simulink library "MBDS_Subsystems"  (R2018b)
settings: Solver=ode45  StartTime=0.0  StopTime=10.0  RelTol=1e-3
libraries: KIBES_Signal x1429, MBDS_Modules x44, simulink x2
(part 12 of 15)

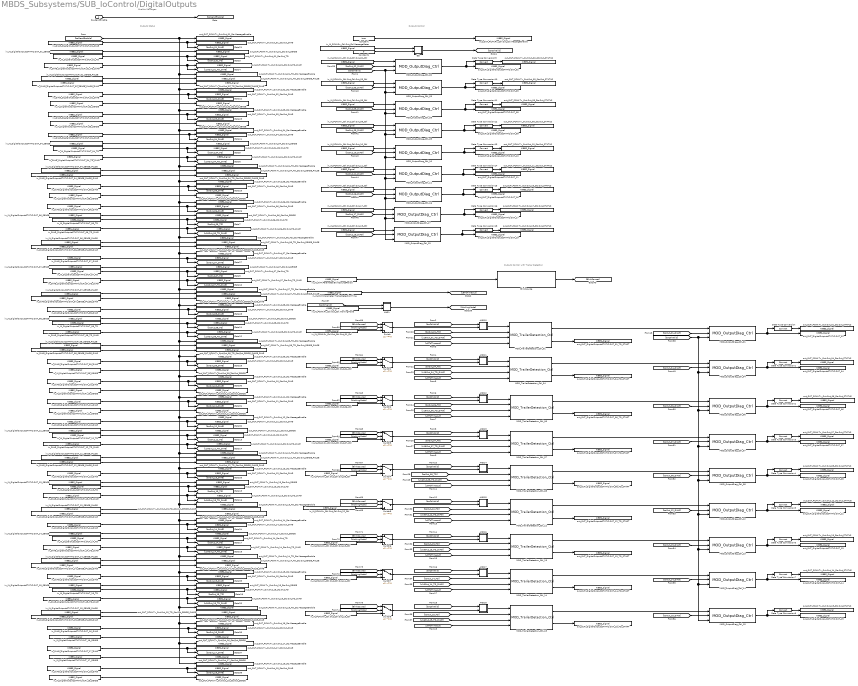
== system MBDS_Subsystems/SUB_IoControl/DigitalOutputs ==
  note: Outputs Control with Trailer Detection
  note: Outputs Control
  note: Enable Messages
  note: Outputs Status
  bo_SendEnable : Inport
  AND1 : Subsystem  InitFcn=|  mask(AND){MBDS_LibraryBlock=on, BitwiseMode=off, Inputs=2, UseBitMask=off, BitMask='A7', OutDataTypeStr=Inherit: Inherit via back propagation, MBDS_BlockVersion=08.20.02}
      | if(exist('MBDS_BlockCallback', 'file'))
      |    MBDS_BlockCallback('Update', gcb);
      | end
      mask prompts: MBDS_LibraryBlock "MBDS library block"; BitwiseMode "Use 'bitwise' mode"; Inputs "Number of input ports:"; UseBitMask "Use bit mask"; BitMask "Bit mask:"; OutDataTypeStr "Output data type:"; MBDS_BlockVersion "Version:"
      mask help: Logical or bitwise AND operator. For multiple inputs, operators are applied across the inputs. For a single input, operators are applied across the input vector. In bitwise mode a bit mask can be applied onto single input signals.
      mask init: same as MBDS_Subsystems/SUB_DateTime/AND
      mask Help: eval(['open([workdir(''library_dir:''),''\Blockset\help\'',get_param(gcb,''MaskType''),''.html''])'])
      mask Callback BitwiseMode:
      | if(exist('MBDS_BlockCallback', 'file'))
      |    MBDS_BlockCallback('BitwiseMode', gcb);
      | end
      mask Callback Inputs:
      | if(exist('MBDS_BlockCallback', 'file'))
      |    MBDS_BlockCallback('Inputs', gcb);
      | end
      mask Callback UseBitMask:
      | if(exist('MBDS_BlockCallback', 'file'))
      |    MBDS_BlockCallback('UseBitMask', gcb);
      | end
      mask Callback BitMask:
      | if(exist('MBDS_BlockCallback', 'file'))
      |    MBDS_BlockCallback('BitMask', gcb);
      | end
      mask TypeOptions OutDataTypeStr: Inherit: Inherit via back propagation | int8 | uint8 | int16 | uint16 | int32 | uint32 | boolean
      mask Callback OutDataTypeStr:
      | % Adopt Value
      | if(exist('MBDS_BlockCallback', 'file'))
      |    MBDS_BlockCallback('OutDataTypeStr', gcb);
      | end
      mask DialogControl ParameterTabVar0 Prompt: Main
      mask DialogControl ParameterTabVar01 Prompt: Signal Attributes
      mask DialogControl ParameterTabVar012 Prompt: Version
      mask Display:
      | % Show icon or block text
      | if(UseBitMask)
      |    if(isnumeric(BitMask))
      |       BitMaskString = ['0x',dec2hex(floor(BitMask))];
      |    elseif(ischar(BitMask))
      |       BitMaskString = ['0x',upper(BitMask)];
      |    else
      |       BitMaskString = '???';
      |    end
      |    disp(sprintf(['AND\n', BitMaskString]))
      | else
      |    disp('AND')
      | end
  AND10 : Subsystem  InitFcn=|  mask(AND){MBDS_LibraryBlock=on, BitwiseMode=off, Inputs=2, UseBitMask=off, BitMask='A7', OutDataTypeStr=Inherit: Inherit via back propagation, MBDS_BlockVersion=08.20.02}
      | if(exist('MBDS_BlockCallback', 'file'))
      |    MBDS_BlockCallback('Update', gcb);
      | end
      mask prompts: MBDS_LibraryBlock "MBDS library block"; BitwiseMode "Use 'bitwise' mode"; Inputs "Number of input ports:"; UseBitMask "Use bit mask"; BitMask "Bit mask:"; OutDataTypeStr "Output data type:"; MBDS_BlockVersion "Version:"
      mask help: Logical or bitwise AND operator. For multiple inputs, operators are applied across the inputs. For a single input, operators are applied across the input vector. In bitwise mode a bit mask can be applied onto single input signals.
      mask init: same as MBDS_Subsystems/SUB_DateTime/AND
      mask Help: eval(['open([workdir(''library_dir:''),''\Blockset\help\'',get_param(gcb,''MaskType''),''.html''])'])
      mask Callback BitwiseMode:
      | if(exist('MBDS_BlockCallback', 'file'))
      |    MBDS_BlockCallback('BitwiseMode', gcb);
      | end
      mask Callback Inputs:
      | if(exist('MBDS_BlockCallback', 'file'))
      |    MBDS_BlockCallback('Inputs', gcb);
      | end
      mask Callback UseBitMask:
      | if(exist('MBDS_BlockCallback', 'file'))
      |    MBDS_BlockCallback('UseBitMask', gcb);
      | end
      mask Callback BitMask:
      | if(exist('MBDS_BlockCallback', 'file'))
      |    MBDS_BlockCallback('BitMask', gcb);
      | end
      mask TypeOptions OutDataTypeStr: Inherit: Inherit via back propagation | int8 | uint8 | int16 | uint16 | int32 | uint32 | boolean
      mask Callback OutDataTypeStr:
      | % Adopt Value
      | if(exist('MBDS_BlockCallback', 'file'))
      |    MBDS_BlockCallback('OutDataTypeStr', gcb);
      | end
      mask DialogControl ParameterTabVar0 Prompt: Main
      mask DialogControl ParameterTabVar01 Prompt: Signal Attributes
      mask DialogControl ParameterTabVar012 Prompt: Version
      mask Display:
      | % Show icon or block text
      | if(UseBitMask)
      |    if(isnumeric(BitMask))
      |       BitMaskString = ['0x',dec2hex(floor(BitMask))];
      |    elseif(ischar(BitMask))
      |       BitMaskString = ['0x',upper(BitMask)];
      |    else
      |       BitMaskString = '???';
      |    end
      |    disp(sprintf(['AND\n', BitMaskString]))
      | else
      |    disp('AND')
      | end
  AND11 : Subsystem  InitFcn=|  mask(AND){MBDS_LibraryBlock=on, BitwiseMode=off, Inputs=2, UseBitMask=off, BitMask='A7', OutDataTypeStr=Inherit: Inherit via back propagation, MBDS_BlockVersion=08.20.02}
      | if(exist('MBDS_BlockCallback', 'file'))
      |    MBDS_BlockCallback('Update', gcb);
      | end
      mask prompts: MBDS_LibraryBlock "MBDS library block"; BitwiseMode "Use 'bitwise' mode"; Inputs "Number of input ports:"; UseBitMask "Use bit mask"; BitMask "Bit mask:"; OutDataTypeStr "Output data type:"; MBDS_BlockVersion "Version:"
      mask help: Logical or bitwise AND operator. For multiple inputs, operators are applied across the inputs. For a single input, operators are applied across the input vector. In bitwise mode a bit mask can be applied onto single input signals.
      mask init: same as MBDS_Subsystems/SUB_DateTime/AND
      mask Help: eval(['open([workdir(''library_dir:''),''\Blockset\help\'',get_param(gcb,''MaskType''),''.html''])'])
      mask Callback BitwiseMode:
      | if(exist('MBDS_BlockCallback', 'file'))
      |    MBDS_BlockCallback('BitwiseMode', gcb);
      | end
      mask Callback Inputs:
      | if(exist('MBDS_BlockCallback', 'file'))
      |    MBDS_BlockCallback('Inputs', gcb);
      | end
      mask Callback UseBitMask:
      | if(exist('MBDS_BlockCallback', 'file'))
      |    MBDS_BlockCallback('UseBitMask', gcb);
      | end
      mask Callback BitMask:
      | if(exist('MBDS_BlockCallback', 'file'))
      |    MBDS_BlockCallback('BitMask', gcb);
      | end
      mask TypeOptions OutDataTypeStr: Inherit: Inherit via back propagation | int8 | uint8 | int16 | uint16 | int32 | uint32 | boolean
      mask Callback OutDataTypeStr:
      | % Adopt Value
      | if(exist('MBDS_BlockCallback', 'file'))
      |    MBDS_BlockCallback('OutDataTypeStr', gcb);
      | end
      mask DialogControl ParameterTabVar0 Prompt: Main
      mask DialogControl ParameterTabVar01 Prompt: Signal Attributes
      mask DialogControl ParameterTabVar012 Prompt: Version
      mask Display:
      | % Show icon or block text
      | if(UseBitMask)
      |    if(isnumeric(BitMask))
      |       BitMaskString = ['0x',dec2hex(floor(BitMask))];
      |    elseif(ischar(BitMask))
      |       BitMaskString = ['0x',upper(BitMask)];
      |    else
      |       BitMaskString = '???';
      |    end
      |    disp(sprintf(['AND\n', BitMaskString]))
      | else
      |    disp('AND')
      | end
  AND12 : Subsystem  InitFcn=|  mask(AND){MBDS_LibraryBlock=on, BitwiseMode=off, Inputs=2, UseBitMask=off, BitMask='A7', OutDataTypeStr=Inherit: Inherit via back propagation, MBDS_BlockVersion=08.20.02}
      | if(exist('MBDS_BlockCallback', 'file'))
      |    MBDS_BlockCallback('Update', gcb);
      | end
      mask prompts: MBDS_LibraryBlock "MBDS library block"; BitwiseMode "Use 'bitwise' mode"; Inputs "Number of input ports:"; UseBitMask "Use bit mask"; BitMask "Bit mask:"; OutDataTypeStr "Output data type:"; MBDS_BlockVersion "Version:"
      mask help: Logical or bitwise AND operator. For multiple inputs, operators are applied across the inputs. For a single input, operators are applied across the input vector. In bitwise mode a bit mask can be applied onto single input signals.
      mask init: same as MBDS_Subsystems/SUB_DateTime/AND
      mask Help: eval(['open([workdir(''library_dir:''),''\Blockset\help\'',get_param(gcb,''MaskType''),''.html''])'])
      mask Callback BitwiseMode:
      | if(exist('MBDS_BlockCallback', 'file'))
      |    MBDS_BlockCallback('BitwiseMode', gcb);
      | end
      mask Callback Inputs:
      | if(exist('MBDS_BlockCallback', 'file'))
      |    MBDS_BlockCallback('Inputs', gcb);
      | end
      mask Callback UseBitMask:
      | if(exist('MBDS_BlockCallback', 'file'))
      |    MBDS_BlockCallback('UseBitMask', gcb);
      | end
      mask Callback BitMask:
      | if(exist('MBDS_BlockCallback', 'file'))
      |    MBDS_BlockCallback('BitMask', gcb);
      | end
      mask TypeOptions OutDataTypeStr: Inherit: Inherit via back propagation | int8 | uint8 | int16 | uint16 | int32 | uint32 | boolean
      mask Callback OutDataTypeStr:
      | % Adopt Value
      | if(exist('MBDS_BlockCallback', 'file'))
      |    MBDS_BlockCallback('OutDataTypeStr', gcb);
      | end
      mask DialogControl ParameterTabVar0 Prompt: Main
      mask DialogControl ParameterTabVar01 Prompt: Signal Attributes
      mask DialogControl ParameterTabVar012 Prompt: Version
      mask Display:
      | % Show icon or block text
      | if(UseBitMask)
      |    if(isnumeric(BitMask))
      |       BitMaskString = ['0x',dec2hex(floor(BitMask))];
      |    elseif(ischar(BitMask))
      |       BitMaskString = ['0x',upper(BitMask)];
      |    else
      |       BitMaskString = '???';
      |    end
      |    disp(sprintf(['AND\n', BitMaskString]))
      | else
      |    disp('AND')
      | end
  AND13 : Subsystem  InitFcn=|  mask(AND){MBDS_LibraryBlock=on, BitwiseMode=off, Inputs=2, UseBitMask=off, BitMask='A7', OutDataTypeStr=Inherit: Inherit via back propagation, MBDS_BlockVersion=08.20.02}
      | if(exist('MBDS_BlockCallback', 'file'))
      |    MBDS_BlockCallback('Update', gcb);
      | end
      mask prompts: MBDS_LibraryBlock "MBDS library block"; BitwiseMode "Use 'bitwise' mode"; Inputs "Number of input ports:"; UseBitMask "Use bit mask"; BitMask "Bit mask:"; OutDataTypeStr "Output data type:"; MBDS_BlockVersion "Version:"
      mask help: Logical or bitwise AND operator. For multiple inputs, operators are applied across the inputs. For a single input, operators are applied across the input vector. In bitwise mode a bit mask can be applied onto single input signals.
      mask init: same as MBDS_Subsystems/SUB_DateTime/AND
      mask Help: eval(['open([workdir(''library_dir:''),''\Blockset\help\'',get_param(gcb,''MaskType''),''.html''])'])
      mask Callback BitwiseMode:
      | if(exist('MBDS_BlockCallback', 'file'))
      |    MBDS_BlockCallback('BitwiseMode', gcb);
      | end
      mask Callback Inputs:
      | if(exist('MBDS_BlockCallback', 'file'))
      |    MBDS_BlockCallback('Inputs', gcb);
      | end
      mask Callback UseBitMask:
      | if(exist('MBDS_BlockCallback', 'file'))
      |    MBDS_BlockCallback('UseBitMask', gcb);
      | end
      mask Callback BitMask:
      | if(exist('MBDS_BlockCallback', 'file'))
      |    MBDS_BlockCallback('BitMask', gcb);
      | end
      mask TypeOptions OutDataTypeStr: Inherit: Inherit via back propagation | int8 | uint8 | int16 | uint16 | int32 | uint32 | boolean
      mask Callback OutDataTypeStr:
      | % Adopt Value
      | if(exist('MBDS_BlockCallback', 'file'))
      |    MBDS_BlockCallback('OutDataTypeStr', gcb);
      | end
      mask DialogControl ParameterTabVar0 Prompt: Main
      mask DialogControl ParameterTabVar01 Prompt: Signal Attributes
      mask DialogControl ParameterTabVar012 Prompt: Version
      mask Display:
      | % Show icon or block text
      | if(UseBitMask)
      |    if(isnumeric(BitMask))
      |       BitMaskString = ['0x',dec2hex(floor(BitMask))];
      |    elseif(ischar(BitMask))
      |       BitMaskString = ['0x',upper(BitMask)];
      |    else
      |       BitMaskString = '???';
      |    end
      |    disp(sprintf(['AND\n', BitMaskString]))
      | else
      |    disp('AND')
      | end
  AND14 : Subsystem  InitFcn=|  mask(AND){MBDS_LibraryBlock=on, BitwiseMode=off, Inputs=2, UseBitMask=off, BitMask='A7', OutDataTypeStr=Inherit: Inherit via back propagation, MBDS_BlockVersion=08.20.02}
      | if(exist('MBDS_BlockCallback', 'file'))
      |    MBDS_BlockCallback('Update', gcb);
      | end
      mask prompts: MBDS_LibraryBlock "MBDS library block"; BitwiseMode "Use 'bitwise' mode"; Inputs "Number of input ports:"; UseBitMask "Use bit mask"; BitMask "Bit mask:"; OutDataTypeStr "Output data type:"; MBDS_BlockVersion "Version:"
      mask help: Logical or bitwise AND operator. For multiple inputs, operators are applied across the inputs. For a single input, operators are applied across the input vector. In bitwise mode a bit mask can be applied onto single input signals.
      mask init: same as MBDS_Subsystems/SUB_DateTime/AND
      mask Help: eval(['open([workdir(''library_dir:''),''\Blockset\help\'',get_param(gcb,''MaskType''),''.html''])'])
      mask Callback BitwiseMode:
      | if(exist('MBDS_BlockCallback', 'file'))
      |    MBDS_BlockCallback('BitwiseMode', gcb);
      | end
      mask Callback Inputs:
      | if(exist('MBDS_BlockCallback', 'file'))
      |    MBDS_BlockCallback('Inputs', gcb);
      | end
      mask Callback UseBitMask:
      | if(exist('MBDS_BlockCallback', 'file'))
      |    MBDS_BlockCallback('UseBitMask', gcb);
      | end
      mask Callback BitMask:
      | if(exist('MBDS_BlockCallback', 'file'))
      |    MBDS_BlockCallback('BitMask', gcb);
      | end
      mask TypeOptions OutDataTypeStr: Inherit: Inherit via back propagation | int8 | uint8 | int16 | uint16 | int32 | uint32 | boolean
      mask Callback OutDataTypeStr:
      | % Adopt Value
      | if(exist('MBDS_BlockCallback', 'file'))
      |    MBDS_BlockCallback('OutDataTypeStr', gcb);
      | end
      mask DialogControl ParameterTabVar0 Prompt: Main
      mask DialogControl ParameterTabVar01 Prompt: Signal Attributes
      mask DialogControl ParameterTabVar012 Prompt: Version
      mask Display:
      | % Show icon or block text
      | if(UseBitMask)
      |    if(isnumeric(BitMask))
      |       BitMaskString = ['0x',dec2hex(floor(BitMask))];
      |    elseif(ischar(BitMask))
      |       BitMaskString = ['0x',upper(BitMask)];
      |    else
      |       BitMaskString = '???';
      |    end
      |    disp(sprintf(['AND\n', BitMaskString]))
      | else
      |    disp('AND')
      | end
  AND15 : Subsystem  InitFcn=|  mask(AND){MBDS_LibraryBlock=on, BitwiseMode=off, Inputs=2, UseBitMask=off, BitMask='A7', OutDataTypeStr=Inherit: Inherit via back propagation, MBDS_BlockVersion=08.20.02}
      | if(exist('MBDS_BlockCallback', 'file'))
      |    MBDS_BlockCallback('Update', gcb);
      | end
      mask prompts: MBDS_LibraryBlock "MBDS library block"; BitwiseMode "Use 'bitwise' mode"; Inputs "Number of input ports:"; UseBitMask "Use bit mask"; BitMask "Bit mask:"; OutDataTypeStr "Output data type:"; MBDS_BlockVersion "Version:"
      mask help: Logical or bitwise AND operator. For multiple inputs, operators are applied across the inputs. For a single input, operators are applied across the input vector. In bitwise mode a bit mask can be applied onto single input signals.
      mask init: same as MBDS_Subsystems/SUB_DateTime/AND
      mask Help: eval(['open([workdir(''library_dir:''),''\Blockset\help\'',get_param(gcb,''MaskType''),''.html''])'])
      mask Callback BitwiseMode:
      | if(exist('MBDS_BlockCallback', 'file'))
      |    MBDS_BlockCallback('BitwiseMode', gcb);
      | end
      mask Callback Inputs:
      | if(exist('MBDS_BlockCallback', 'file'))
      |    MBDS_BlockCallback('Inputs', gcb);
      | end
      mask Callback UseBitMask:
      | if(exist('MBDS_BlockCallback', 'file'))
      |    MBDS_BlockCallback('UseBitMask', gcb);
      | end
      mask Callback BitMask:
      | if(exist('MBDS_BlockCallback', 'file'))
      |    MBDS_BlockCallback('BitMask', gcb);
      | end
      mask TypeOptions OutDataTypeStr: Inherit: Inherit via back propagation | int8 | uint8 | int16 | uint16 | int32 | uint32 | boolean
      mask Callback OutDataTypeStr:
      | % Adopt Value
      | if(exist('MBDS_BlockCallback', 'file'))
      |    MBDS_BlockCallback('OutDataTypeStr', gcb);
      | end
      mask DialogControl ParameterTabVar0 Prompt: Main
      mask DialogControl ParameterTabVar01 Prompt: Signal Attributes
      mask DialogControl ParameterTabVar012 Prompt: Version
      mask Display:
      | % Show icon or block text
      | if(UseBitMask)
      |    if(isnumeric(BitMask))
      |       BitMaskString = ['0x',dec2hex(floor(BitMask))];
      |    elseif(ischar(BitMask))
      |       BitMaskString = ['0x',upper(BitMask)];
      |    else
      |       BitMaskString = '???';
      |    end
      |    disp(sprintf(['AND\n', BitMaskString]))
      | else
      |    disp('AND')
      | end
  AND16 : Subsystem  InitFcn=|  mask(AND){MBDS_LibraryBlock=on, BitwiseMode=off, Inputs=2, UseBitMask=off, BitMask='A7', OutDataTypeStr=Inherit: Inherit via back propagation, MBDS_BlockVersion=08.20.02}
      | if(exist('MBDS_BlockCallback', 'file'))
      |    MBDS_BlockCallback('Update', gcb);
      | end
      mask prompts: MBDS_LibraryBlock "MBDS library block"; BitwiseMode "Use 'bitwise' mode"; Inputs "Number of input ports:"; UseBitMask "Use bit mask"; BitMask "Bit mask:"; OutDataTypeStr "Output data type:"; MBDS_BlockVersion "Version:"
      mask help: Logical or bitwise AND operator. For multiple inputs, operators are applied across the inputs. For a single input, operators are applied across the input vector. In bitwise mode a bit mask can be applied onto single input signals.
      mask init: same as MBDS_Subsystems/SUB_DateTime/AND
      mask Help: eval(['open([workdir(''library_dir:''),''\Blockset\help\'',get_param(gcb,''MaskType''),''.html''])'])
      mask Callback BitwiseMode:
      | if(exist('MBDS_BlockCallback', 'file'))
      |    MBDS_BlockCallback('BitwiseMode', gcb);
      | end
      mask Callback Inputs:
      | if(exist('MBDS_BlockCallback', 'file'))
      |    MBDS_BlockCallback('Inputs', gcb);
      | end
      mask Callback UseBitMask:
      | if(exist('MBDS_BlockCallback', 'file'))
      |    MBDS_BlockCallback('UseBitMask', gcb);
      | end
      mask Callback BitMask:
      | if(exist('MBDS_BlockCallback', 'file'))
      |    MBDS_BlockCallback('BitMask', gcb);
      | end
      mask TypeOptions OutDataTypeStr: Inherit: Inherit via back propagation | int8 | uint8 | int16 | uint16 | int32 | uint32 | boolean
      mask Callback OutDataTypeStr:
      | % Adopt Value
      | if(exist('MBDS_BlockCallback', 'file'))
      |    MBDS_BlockCallback('OutDataTypeStr', gcb);
      | end
      mask DialogControl ParameterTabVar0 Prompt: Main
      mask DialogControl ParameterTabVar01 Prompt: Signal Attributes
      mask DialogControl ParameterTabVar012 Prompt: Version
      mask Display:
      | % Show icon or block text
      | if(UseBitMask)
      |    if(isnumeric(BitMask))
      |       BitMaskString = ['0x',dec2hex(floor(BitMask))];
      |    elseif(ischar(BitMask))
      |       BitMaskString = ['0x',upper(BitMask)];
      |    else
      |       BitMaskString = '???';
      |    end
      |    disp(sprintf(['AND\n', BitMaskString]))
      | else
      |    disp('AND')
      | end
  AND17 : Subsystem  InitFcn=|  mask(AND){MBDS_LibraryBlock=on, BitwiseMode=off, Inputs=2, UseBitMask=off, BitMask='A7', OutDataTypeStr=Inherit: Inherit via back propagation, MBDS_BlockVersion=08.20.02}
      | if(exist('MBDS_BlockCallback', 'file'))
      |    MBDS_BlockCallback('Update', gcb);
      | end
      mask prompts: MBDS_LibraryBlock "MBDS library block"; BitwiseMode "Use 'bitwise' mode"; Inputs "Number of input ports:"; UseBitMask "Use bit mask"; BitMask "Bit mask:"; OutDataTypeStr "Output data type:"; MBDS_BlockVersion "Version:"
      mask help: Logical or bitwise AND operator. For multiple inputs, operators are applied across the inputs. For a single input, operators are applied across the input vector. In bitwise mode a bit mask can be applied onto single input signals.
      mask init: same as MBDS_Subsystems/SUB_DateTime/AND
      mask Help: eval(['open([workdir(''library_dir:''),''\Blockset\help\'',get_param(gcb,''MaskType''),''.html''])'])
      mask Callback BitwiseMode:
      | if(exist('MBDS_BlockCallback', 'file'))
      |    MBDS_BlockCallback('BitwiseMode', gcb);
      | end
      mask Callback Inputs:
      | if(exist('MBDS_BlockCallback', 'file'))
      |    MBDS_BlockCallback('Inputs', gcb);
      | end
      mask Callback UseBitMask:
      | if(exist('MBDS_BlockCallback', 'file'))
      |    MBDS_BlockCallback('UseBitMask', gcb);
      | end
      mask Callback BitMask:
      | if(exist('MBDS_BlockCallback', 'file'))
      |    MBDS_BlockCallback('BitMask', gcb);
      | end
      mask TypeOptions OutDataTypeStr: Inherit: Inherit via back propagation | int8 | uint8 | int16 | uint16 | int32 | uint32 | boolean
      mask Callback OutDataTypeStr:
      | % Adopt Value
      | if(exist('MBDS_BlockCallback', 'file'))
      |    MBDS_BlockCallback('OutDataTypeStr', gcb);
      | end
      mask DialogControl ParameterTabVar0 Prompt: Main
      mask DialogControl ParameterTabVar01 Prompt: Signal Attributes
      mask DialogControl ParameterTabVar012 Prompt: Version
      mask Display:
      | % Show icon or block text
      | if(UseBitMask)
      |    if(isnumeric(BitMask))
      |       BitMaskString = ['0x',dec2hex(floor(BitMask))];
      |    elseif(ischar(BitMask))
      |       BitMaskString = ['0x',upper(BitMask)];
      |    else
      |       BitMaskString = '???';
      |    end
      |    disp(sprintf(['AND\n', BitMaskString]))
      | else
      |    disp('AND')
      | end
  AND18 : Subsystem  InitFcn=|  mask(AND){MBDS_LibraryBlock=on, BitwiseMode=off, Inputs=2, UseBitMask=off, BitMask='A7', OutDataTypeStr=Inherit: Inherit via back propagation, MBDS_BlockVersion=08.20.02}
      | if(exist('MBDS_BlockCallback', 'file'))
      |    MBDS_BlockCallback('Update', gcb);
      | end
      mask prompts: MBDS_LibraryBlock "MBDS library block"; BitwiseMode "Use 'bitwise' mode"; Inputs "Number of input ports:"; UseBitMask "Use bit mask"; BitMask "Bit mask:"; OutDataTypeStr "Output data type:"; MBDS_BlockVersion "Version:"
      mask help: Logical or bitwise AND operator. For multiple inputs, operators are applied across the inputs. For a single input, operators are applied across the input vector. In bitwise mode a bit mask can be applied onto single input signals.
      mask init: same as MBDS_Subsystems/SUB_DateTime/AND
      mask Help: eval(['open([workdir(''library_dir:''),''\Blockset\help\'',get_param(gcb,''MaskType''),''.html''])'])
      mask Callback BitwiseMode:
      | if(exist('MBDS_BlockCallback', 'file'))
      |    MBDS_BlockCallback('BitwiseMode', gcb);
      | end
      mask Callback Inputs:
      | if(exist('MBDS_BlockCallback', 'file'))
      |    MBDS_BlockCallback('Inputs', gcb);
      | end
      mask Callback UseBitMask:
      | if(exist('MBDS_BlockCallback', 'file'))
      |    MBDS_BlockCallback('UseBitMask', gcb);
      | end
      mask Callback BitMask:
      | if(exist('MBDS_BlockCallback', 'file'))
      |    MBDS_BlockCallback('BitMask', gcb);
      | end
      mask TypeOptions OutDataTypeStr: Inherit: Inherit via back propagation | int8 | uint8 | int16 | uint16 | int32 | uint32 | boolean
      mask Callback OutDataTypeStr:
      | % Adopt Value
      | if(exist('MBDS_BlockCallback', 'file'))
      |    MBDS_BlockCallback('OutDataTypeStr', gcb);
      | end
      mask DialogControl ParameterTabVar0 Prompt: Main
      mask DialogControl ParameterTabVar01 Prompt: Signal Attributes
      mask DialogControl ParameterTabVar012 Prompt: Version
      mask Display:
      | % Show icon or block text
      | if(UseBitMask)
      |    if(isnumeric(BitMask))
      |       BitMaskString = ['0x',dec2hex(floor(BitMask))];
      |    elseif(ischar(BitMask))
      |       BitMaskString = ['0x',upper(BitMask)];
      |    else
      |       BitMaskString = '???';
      |    end
      |    disp(sprintf(['AND\n', BitMaskString]))
      | else
      |    disp('AND')
      | end
  BlinkSource : Stateflow chart  TreatAsAtomicUnit=on
      settings: CopyFcn=|
      | if(exist('MBDS_BlockCallback', 'file'))
      |    MBDS_BlockCallback('Copy', gcb);
      | end
  Constant : Constant  InitFcn=|  Value=true
      | if(exist('MBDS_BlockCallback', 'file'))
      |    MBDS_BlockCallback('Update', gcb);  
      | end
  Constant1 : Constant  InitFcn=|  Value=0  OutDataTypeStr=uint16
      | if(exist('MBDS_BlockCallback', 'file'))
      |    MBDS_BlockCallback('Update', gcb);  
      | end
  Data Type Conversion : DataTypeConversion  InitFcn=|  SaturateOnIntegerOverflow=on
      | try
      |    MBDS_BlockCallback('Update', gcb);
      | end
      settings: AttributesFormatString=Saturate: %<SaturateOnIntegerOverflow>
  Data Type Conversion1 : DataTypeConversion  InitFcn=|  SaturateOnIntegerOverflow=on
      | try
      |    MBDS_BlockCallback('Update', gcb);
      | end
      settings: AttributesFormatString=Saturate: %<SaturateOnIntegerOverflow>
  Data Type Conversion10 : DataTypeConversion  InitFcn=|  SaturateOnIntegerOverflow=on
      | try
      |    MBDS_BlockCallback('Update', gcb);
      | end
      settings: AttributesFormatString=Saturate: %<SaturateOnIntegerOverflow>
  Data Type Conversion11 : DataTypeConversion  InitFcn=|  SaturateOnIntegerOverflow=on
      | try
      |    MBDS_BlockCallback('Update', gcb);
      | end
      settings: AttributesFormatString=Saturate: %<SaturateOnIntegerOverflow>
  Data Type Conversion12 : DataTypeConversion  InitFcn=|  SaturateOnIntegerOverflow=on
      | try
      |    MBDS_BlockCallback('Update', gcb);
      | end
      settings: AttributesFormatString=Saturate: %<SaturateOnIntegerOverflow>
  Data Type Conversion13 : DataTypeConversion  InitFcn=|  SaturateOnIntegerOverflow=on
      | try
      |    MBDS_BlockCallback('Update', gcb);
      | end
      settings: AttributesFormatString=Saturate: %<SaturateOnIntegerOverflow>
  Data Type Conversion14 : DataTypeConversion  InitFcn=|  SaturateOnIntegerOverflow=on
      | try
      |    MBDS_BlockCallback('Update', gcb);
      | end
      settings: AttributesFormatString=Saturate: %<SaturateOnIntegerOverflow>
  Data Type Conversion15 : DataTypeConversion  InitFcn=|  SaturateOnIntegerOverflow=on
      | try
      |    MBDS_BlockCallback('Update', gcb);
      | end
      settings: AttributesFormatString=Saturate: %<SaturateOnIntegerOverflow>
  Data Type Conversion16 : DataTypeConversion  InitFcn=|  SaturateOnIntegerOverflow=on
      | try
      |    MBDS_BlockCallback('Update', gcb);
      | end
      settings: AttributesFormatString=Saturate: %<SaturateOnIntegerOverflow>
  Data Type Conversion18 : DataTypeConversion  InitFcn=|  SaturateOnIntegerOverflow=on
      | try
      |    MBDS_BlockCallback('Update', gcb);
      | end
      settings: AttributesFormatString=Saturate: %<SaturateOnIntegerOverflow>
  Data Type Conversion2 : DataTypeConversion  InitFcn=|  SaturateOnIntegerOverflow=on
      | try
      |    MBDS_BlockCallback('Update', gcb);
      | end
      settings: AttributesFormatString=Saturate: %<SaturateOnIntegerOverflow>
  Data Type Conversion3 : DataTypeConversion  InitFcn=|  SaturateOnIntegerOverflow=on
      | try
      |    MBDS_BlockCallback('Update', gcb);
      | end
      settings: AttributesFormatString=Saturate: %<SaturateOnIntegerOverflow>
  Data Type Conversion4 : DataTypeConversion  InitFcn=|  SaturateOnIntegerOverflow=on
      | try
      |    MBDS_BlockCallback('Update', gcb);
      | end
      settings: AttributesFormatString=Saturate: %<SaturateOnIntegerOverflow>
  Data Type Conversion5 : DataTypeConversion  InitFcn=|  SaturateOnIntegerOverflow=on
      | try
      |    MBDS_BlockCallback('Update', gcb);
      | end
      settings: AttributesFormatString=Saturate: %<SaturateOnIntegerOverflow>
  Data Type Conversion6 : DataTypeConversion  InitFcn=|  SaturateOnIntegerOverflow=on
      | try
      |    MBDS_BlockCallback('Update', gcb);
      | end
      settings: AttributesFormatString=Saturate: %<SaturateOnIntegerOverflow>
  Data Type Conversion7 : DataTypeConversion  InitFcn=|  SaturateOnIntegerOverflow=on
      | try
      |    MBDS_BlockCallback('Update', gcb);
      | end
      settings: AttributesFormatString=Saturate: %<SaturateOnIntegerOverflow>
  Data Type Conversion8 : DataTypeConversion  InitFcn=|  SaturateOnIntegerOverflow=on
      | try
      |    MBDS_BlockCallback('Update', gcb);
      | end
      settings: AttributesFormatString=Saturate: %<SaturateOnIntegerOverflow>
  Data Type Conversion9 : DataTypeConversion  InitFcn=|  SaturateOnIntegerOverflow=on
      | try
      |    MBDS_BlockCallback('Update', gcb);
      | end
      settings: AttributesFormatString=Saturate: %<SaturateOnIntegerOverflow>
  EQ : Subsystem  InitFcn=|  mask(EQ){MBDS_LibraryBlock=on, InputSameDT=on, MBDS_BlockVersion=08.20.02}
      | if(exist('MBDS_BlockCallback', 'file'))
      |    MBDS_BlockCallback('Update', gcb);
      | end
      mask prompts: MBDS_LibraryBlock "MBDS library block"; InputSameDT "Require all inputs to have the same data type"; MBDS_BlockVersion "Block version:"
      mask help: The block compares if both input signals are equal.
      mask init: same as MBDS_Subsystems/SUB_DateTime/AND
      mask Help: eval(['open([workdir(''library_dir:''),''\Blockset\help\'',get_param(gcb,''MaskType''),''.html''])'])
      mask Callback InputSameDT:
      | % Adopt value
      | if(exist('MBDS_BlockCallback', 'file'))
      |    MBDS_BlockCallback('InputSameDT', gcb);
      | end
      mask DialogControl ParameterTabVar0 Prompt: Signal Attributes
      mask DialogControl ParameterTabVar01 Prompt: Version
      mask Display:
      | % Show icon or block text
      | if(exist('MBDS_BlockCallback', 'file'))
      |    image(imread('EQ.tif','tif'),[0.35,0.35,0.355,0.25])
      |    disp('')
      | else
      |    disp(sprintf('=='));
      | end
  MOD_OutputDiag_Ctrl_01 : MBDS_Modules/MOD_OutputDiag_Ctrl  Description=Controls output based on diagnostic signal  MBDS_ElementType=Module  MBDS_WorkStatus=In Work  MBDS_LastModified=2021-03-24-09:50:46
      settings: SourceProductName=MBDS Project Library
  MOD_OutputDiag_Ctrl_02 : MBDS_Modules/MOD_OutputDiag_Ctrl  Description=Controls output based on diagnostic signal  MBDS_ElementType=Module  MBDS_WorkStatus=In Work  MBDS_LastModified=2021-03-24-09:50:46
      settings: SourceProductName=MBDS Project Library
  MOD_OutputDiag_Ctrl_03 : MBDS_Modules/MOD_OutputDiag_Ctrl  Description=Controls output based on diagnostic signal  MBDS_ElementType=Module  MBDS_WorkStatus=In Work  MBDS_LastModified=2021-03-24-09:50:46
      settings: SourceProductName=MBDS Project Library
  MOD_OutputDiag_Ctrl_04 : MBDS_Modules/MOD_OutputDiag_Ctrl  Description=Controls output based on diagnostic signal  MBDS_ElementType=Module  MBDS_WorkStatus=In Work  MBDS_LastModified=2021-03-24-09:50:46
      settings: SourceProductName=MBDS Project Library
  MOD_OutputDiag_Ctrl_05 : MBDS_Modules/MOD_OutputDiag_Ctrl  Description=Controls output based on diagnostic signal  MBDS_ElementType=Module  MBDS_WorkStatus=In Work  MBDS_LastModified=2021-03-24-09:50:46
      settings: SourceProductName=MBDS Project Library
  MOD_OutputDiag_Ctrl_06 : MBDS_Modules/MOD_OutputDiag_Ctrl  Description=Controls output based on diagnostic signal  MBDS_ElementType=Module  MBDS_WorkStatus=In Work  MBDS_LastModified=2021-03-24-09:50:46
      settings: SourceProductName=MBDS Project Library
  MOD_OutputDiag_Ctrl_07 : MBDS_Modules/MOD_OutputDiag_Ctrl  Description=Controls output based on diagnostic signal  MBDS_ElementType=Module  MBDS_WorkStatus=In Work  MBDS_LastModified=2021-03-24-09:50:46
      settings: SourceProductName=MBDS Project Library
  MOD_OutputDiag_Ctrl_08 : MBDS_Modules/MOD_OutputDiag_Ctrl  Description=Controls output based on diagnostic signal  MBDS_ElementType=Module  MBDS_WorkStatus=In Work  MBDS_LastModified=2021-03-24-09:50:46
      settings: SourceProductName=MBDS Project Library
  MOD_OutputDiag_Ctrl_09 : MBDS_Modules/MOD_OutputDiag_Ctrl  Description=Controls output based on diagnostic signal  MBDS_ElementType=Module  MBDS_WorkStatus=In Work  MBDS_LastModified=2021-03-24-09:50:46
      settings: SourceProductName=MBDS Project Library
  MOD_OutputDiag_Ctrl_{10..17,19} (9 alike) : MBDS_Modules/MOD_OutputDiag_Ctrl  Description=Controls output based on diagnostic signal  MBDS_ElementType=Module  MBDS_WorkStatus=In Work  MBDS_LastModified=2021-03-24-09:50:46
      settings: SourceProductName=MBDS Project Library
  MOD_TrailerDetection_Ctrl_01 : MBDS_Modules/MOD_TrailerDetection_Ctrl  Description=Control outputs with Trailer detection hardware.  MBDS_ElementType=Module  MBDS_WorkStatus=In Work  MBDS_LastModified=2020-12-22-13:33:50
      settings: SourceProductName=MBDS Project Library
  MOD_TrailerDetection_Ctrl_04 : MBDS_Modules/MOD_TrailerDetection_Ctrl  Description=Control outputs with Trailer detection hardware.  MBDS_ElementType=Module  MBDS_WorkStatus=In Work  MBDS_LastModified=2020-12-22-13:33:50
      settings: SourceProductName=MBDS Project Library
  MOD_TrailerDetection_Ctrl_06 : MBDS_Modules/MOD_TrailerDetection_Ctrl  Description=Control outputs with Trailer detection hardware.  MBDS_ElementType=Module  MBDS_WorkStatus=In Work  MBDS_LastModified=2020-12-22-13:33:50
      settings: SourceProductName=MBDS Project Library
  MOD_TrailerDetection_Ctrl_07 : MBDS_Modules/MOD_TrailerDetection_Ctrl  Description=Control outputs with Trailer detection hardware.  MBDS_ElementType=Module  MBDS_WorkStatus=In Work  MBDS_LastModified=2020-12-22-13:33:50
      settings: SourceProductName=MBDS Project Library
  MOD_TrailerDetection_Ctrl_08 : MBDS_Modules/MOD_TrailerDetection_Ctrl  Description=Control outputs with Trailer detection hardware.  MBDS_ElementType=Module  MBDS_WorkStatus=In Work  MBDS_LastModified=2020-12-22-13:33:50
      settings: SourceProductName=MBDS Project Library
  MOD_TrailerDetection_Ctrl_{12..15} (4 alike) : MBDS_Modules/MOD_TrailerDetection_Ctrl  Description=Control outputs with Trailer detection hardware.  MBDS_ElementType=Module  MBDS_WorkStatus=In Work  MBDS_LastModified=2020-12-22-13:33:50
      settings: SourceProductName=MBDS Project Library
  Switch : Switch  InitFcn=|  Criteria=u2 ~= 0  OutDataTypeStr=Inherit: Inherit via back propagation  mask(Switch){MBDS_LibraryBlock=on, OutDataTypeStr_=Inherit: Inherit via back propagation, SaturateOnIntegerOverflow_=off, InputSameDT_=off, MBDS_BlockVersion=08.20.02}
      | if(exist('MBDS_BlockCallback', 'file'))
      |    MBDS_BlockCallback('Update', gcb);  
      | end
      mask prompts: MBDS_LibraryBlock "MBDS library block"; OutDataTypeStr_ "Output data type:"; SaturateOnIntegerOverflow_ "Saturate on integer overflow"; InputSameDT_ "Require all inputs to have the same data type"; MBDS_BlockVersion "Block version:"
      mask help: Pass through input 1 when input 2 is not equal to zero; otherwise pass through input 3. The inputs are numbered top to bottom (or left to right). The first and third input ports are data ports, and the second input port is the control port.
      mask init: same as MBDS_Subsystems/SUB_DateTime/AND
      mask Help: eval(['open([workdir(''library_dir:''),''\Blockset\help\'',get_param(gcb,''MaskType''),''.html''])'])
      mask TypeOptions OutDataTypeStr_: Inherit: Inherit via back propagation | single | int8 | uint8 | int16 | uint16 | int32 | uint32
      mask DialogControl ParameterTabVar0 Prompt: Signal Attributes
      mask DialogControl ParameterTabVar01 Prompt: Version
  Switch1 : Switch  InitFcn=|  Criteria=u2 ~= 0  OutDataTypeStr=Inherit: Inherit via back propagation  mask(Switch){MBDS_LibraryBlock=on, OutDataTypeStr_=Inherit: Inherit via back propagation, SaturateOnIntegerOverflow_=off, InputSameDT_=off, MBDS_BlockVersion=08.20.02}
      | if(exist('MBDS_BlockCallback', 'file'))
      |    MBDS_BlockCallback('Update', gcb);  
      | end
      mask prompts: MBDS_LibraryBlock "MBDS library block"; OutDataTypeStr_ "Output data type:"; SaturateOnIntegerOverflow_ "Saturate on integer overflow"; InputSameDT_ "Require all inputs to have the same data type"; MBDS_BlockVersion "Block version:"
      mask help: Pass through input 1 when input 2 is not equal to zero; otherwise pass through input 3. The inputs are numbered top to bottom (or left to right). The first and third input ports are data ports, and the second input port is the control port.
      mask init: same as MBDS_Subsystems/SUB_DateTime/AND
      mask Help: eval(['open([workdir(''library_dir:''),''\Blockset\help\'',get_param(gcb,''MaskType''),''.html''])'])
      mask TypeOptions OutDataTypeStr_: Inherit: Inherit via back propagation | single | int8 | uint8 | int16 | uint16 | int32 | uint32
      mask DialogControl ParameterTabVar0 Prompt: Signal Attributes
      mask DialogControl ParameterTabVar01 Prompt: Version
  Switch2 : Switch  InitFcn=|  Criteria=u2 ~= 0  OutDataTypeStr=Inherit: Inherit via back propagation  mask(Switch){MBDS_LibraryBlock=on, OutDataTypeStr_=Inherit: Inherit via back propagation, SaturateOnIntegerOverflow_=off, InputSameDT_=off, MBDS_BlockVersion=08.20.02}
      | if(exist('MBDS_BlockCallback', 'file'))
      |    MBDS_BlockCallback('Update', gcb);  
      | end
      mask prompts: MBDS_LibraryBlock "MBDS library block"; OutDataTypeStr_ "Output data type:"; SaturateOnIntegerOverflow_ "Saturate on integer overflow"; InputSameDT_ "Require all inputs to have the same data type"; MBDS_BlockVersion "Block version:"
      mask help: Pass through input 1 when input 2 is not equal to zero; otherwise pass through input 3. The inputs are numbered top to bottom (or left to right). The first and third input ports are data ports, and the second input port is the control port.
      mask init: same as MBDS_Subsystems/SUB_DateTime/AND
      mask Help: eval(['open([workdir(''library_dir:''),''\Blockset\help\'',get_param(gcb,''MaskType''),''.html''])'])
      mask TypeOptions OutDataTypeStr_: Inherit: Inherit via back propagation | single | int8 | uint8 | int16 | uint16 | int32 | uint32
      mask DialogControl ParameterTabVar0 Prompt: Signal Attributes
      mask DialogControl ParameterTabVar01 Prompt: Version
  Switch3 : Switch  InitFcn=|  Criteria=u2 ~= 0  OutDataTypeStr=Inherit: Inherit via back propagation  mask(Switch){MBDS_LibraryBlock=on, OutDataTypeStr_=Inherit: Inherit via back propagation, SaturateOnIntegerOverflow_=off, InputSameDT_=off, MBDS_BlockVersion=08.20.02}
      | if(exist('MBDS_BlockCallback', 'file'))
      |    MBDS_BlockCallback('Update', gcb);  
      | end
      mask prompts: MBDS_LibraryBlock "MBDS library block"; OutDataTypeStr_ "Output data type:"; SaturateOnIntegerOverflow_ "Saturate on integer overflow"; InputSameDT_ "Require all inputs to have the same data type"; MBDS_BlockVersion "Block version:"
      mask help: Pass through input 1 when input 2 is not equal to zero; otherwise pass through input 3. The inputs are numbered top to bottom (or left to right). The first and third input ports are data ports, and the second input port is the control port.
      mask init: same as MBDS_Subsystems/SUB_DateTime/AND
      mask Help: eval(['open([workdir(''library_dir:''),''\Blockset\help\'',get_param(gcb,''MaskType''),''.html''])'])
      mask TypeOptions OutDataTypeStr_: Inherit: Inherit via back propagation | single | int8 | uint8 | int16 | uint16 | int32 | uint32
      mask DialogControl ParameterTabVar0 Prompt: Signal Attributes
      mask DialogControl ParameterTabVar01 Prompt: Version
  Switch4 : Switch  InitFcn=|  Criteria=u2 ~= 0  OutDataTypeStr=Inherit: Inherit via back propagation  mask(Switch){MBDS_LibraryBlock=on, OutDataTypeStr_=Inherit: Inherit via back propagation, SaturateOnIntegerOverflow_=off, InputSameDT_=off, MBDS_BlockVersion=08.20.02}
      | if(exist('MBDS_BlockCallback', 'file'))
      |    MBDS_BlockCallback('Update', gcb);  
      | end
      mask prompts: MBDS_LibraryBlock "MBDS library block"; OutDataTypeStr_ "Output data type:"; SaturateOnIntegerOverflow_ "Saturate on integer overflow"; InputSameDT_ "Require all inputs to have the same data type"; MBDS_BlockVersion "Block version:"
      mask help: Pass through input 1 when input 2 is not equal to zero; otherwise pass through input 3. The inputs are numbered top to bottom (or left to right). The first and third input ports are data ports, and the second input port is the control port.
      mask init: same as MBDS_Subsystems/SUB_DateTime/AND
      mask Help: eval(['open([workdir(''library_dir:''),''\Blockset\help\'',get_param(gcb,''MaskType''),''.html''])'])
      mask TypeOptions OutDataTypeStr_: Inherit: Inherit via back propagation | single | int8 | uint8 | int16 | uint16 | int32 | uint32
      mask DialogControl ParameterTabVar0 Prompt: Signal Attributes
      mask DialogControl ParameterTabVar01 Prompt: Version
  Switch5 : Switch  InitFcn=|  Criteria=u2 ~= 0  OutDataTypeStr=Inherit: Inherit via back propagation  mask(Switch){MBDS_LibraryBlock=on, OutDataTypeStr_=Inherit: Inherit via back propagation, SaturateOnIntegerOverflow_=off, InputSameDT_=off, MBDS_BlockVersion=08.20.02}
      | if(exist('MBDS_BlockCallback', 'file'))
      |    MBDS_BlockCallback('Update', gcb);  
      | end
      mask prompts: MBDS_LibraryBlock "MBDS library block"; OutDataTypeStr_ "Output data type:"; SaturateOnIntegerOverflow_ "Saturate on integer overflow"; InputSameDT_ "Require all inputs to have the same data type"; MBDS_BlockVersion "Block version:"
      mask help: Pass through input 1 when input 2 is not equal to zero; otherwise pass through input 3. The inputs are numbered top to bottom (or left to right). The first and third input ports are data ports, and the second input port is the control port.
      mask init: same as MBDS_Subsystems/SUB_DateTime/AND
      mask Help: eval(['open([workdir(''library_dir:''),''\Blockset\help\'',get_param(gcb,''MaskType''),''.html''])'])
      mask TypeOptions OutDataTypeStr_: Inherit: Inherit via back propagation | single | int8 | uint8 | int16 | uint16 | int32 | uint32
      mask DialogControl ParameterTabVar0 Prompt: Signal Attributes
      mask DialogControl ParameterTabVar01 Prompt: Version
  Switch6 : Switch  InitFcn=|  Criteria=u2 ~= 0  OutDataTypeStr=Inherit: Inherit via back propagation  mask(Switch){MBDS_LibraryBlock=on, OutDataTypeStr_=Inherit: Inherit via back propagation, SaturateOnIntegerOverflow_=off, InputSameDT_=off, MBDS_BlockVersion=08.20.02}
      | if(exist('MBDS_BlockCallback', 'file'))
      |    MBDS_BlockCallback('Update', gcb);  
      | end
      mask prompts: MBDS_LibraryBlock "MBDS library block"; OutDataTypeStr_ "Output data type:"; SaturateOnIntegerOverflow_ "Saturate on integer overflow"; InputSameDT_ "Require all inputs to have the same data type"; MBDS_BlockVersion "Block version:"
      mask help: Pass through input 1 when input 2 is not equal to zero; otherwise pass through input 3. The inputs are numbered top to bottom (or left to right). The first and third input ports are data ports, and the second input port is the control port.
      mask init: same as MBDS_Subsystems/SUB_DateTime/AND
      mask Help: eval(['open([workdir(''library_dir:''),''\Blockset\help\'',get_param(gcb,''MaskType''),''.html''])'])
      mask TypeOptions OutDataTypeStr_: Inherit: Inherit via back propagation | single | int8 | uint8 | int16 | uint16 | int32 | uint32
      mask DialogControl ParameterTabVar0 Prompt: Signal Attributes
      mask DialogControl ParameterTabVar01 Prompt: Version
  Switch7 : Switch  InitFcn=|  Criteria=u2 ~= 0  OutDataTypeStr=Inherit: Inherit via back propagation  mask(Switch){MBDS_LibraryBlock=on, OutDataTypeStr_=Inherit: Inherit via back propagation, SaturateOnIntegerOverflow_=off, InputSameDT_=off, MBDS_BlockVersion=08.20.02}
      | if(exist('MBDS_BlockCallback', 'file'))
      |    MBDS_BlockCallback('Update', gcb);  
      | end
      mask prompts: MBDS_LibraryBlock "MBDS library block"; OutDataTypeStr_ "Output data type:"; SaturateOnIntegerOverflow_ "Saturate on integer overflow"; InputSameDT_ "Require all inputs to have the same data type"; MBDS_BlockVersion "Block version:"
      mask help: Pass through input 1 when input 2 is not equal to zero; otherwise pass through input 3. The inputs are numbered top to bottom (or left to right). The first and third input ports are data ports, and the second input port is the control port.
      mask init: same as MBDS_Subsystems/SUB_DateTime/AND
      mask Help: eval(['open([workdir(''library_dir:''),''\Blockset\help\'',get_param(gcb,''MaskType''),''.html''])'])
      mask TypeOptions OutDataTypeStr_: Inherit: Inherit via back propagation | single | int8 | uint8 | int16 | uint16 | int32 | uint32
      mask DialogControl ParameterTabVar0 Prompt: Signal Attributes
      mask DialogControl ParameterTabVar01 Prompt: Version
  Switch8 : Switch  InitFcn=|  Criteria=u2 ~= 0  OutDataTypeStr=Inherit: Inherit via back propagation  mask(Switch){MBDS_LibraryBlock=on, OutDataTypeStr_=Inherit: Inherit via back propagation, SaturateOnIntegerOverflow_=off, InputSameDT_=off, MBDS_BlockVersion=08.20.02}
      | if(exist('MBDS_BlockCallback', 'file'))
      |    MBDS_BlockCallback('Update', gcb);  
      | end
      mask prompts: MBDS_LibraryBlock "MBDS library block"; OutDataTypeStr_ "Output data type:"; SaturateOnIntegerOverflow_ "Saturate on integer overflow"; InputSameDT_ "Require all inputs to have the same data type"; MBDS_BlockVersion "Block version:"
      mask help: Pass through input 1 when input 2 is not equal to zero; otherwise pass through input 3. The inputs are numbered top to bottom (or left to right). The first and third input ports are data ports, and the second input port is the control port.
      mask init: same as MBDS_Subsystems/SUB_DateTime/AND
      mask Help: eval(['open([workdir(''library_dir:''),''\Blockset\help\'',get_param(gcb,''MaskType''),''.html''])'])
      mask TypeOptions OutDataTypeStr_: Inherit: Inherit via back propagation | single | int8 | uint8 | int16 | uint16 | int32 | uint32
      mask DialogControl ParameterTabVar0 Prompt: Signal Attributes
      mask DialogControl ParameterTabVar01 Prompt: Version
  in_DIAG_DigitalOutputsSTATIC.OUT_01_DIAG : KIBES_Signal/KIBES_Signal  MBDS_LibraryBlock=on  DatabaseKey=305  SignalName=DIAG_DigitalOutputsSTATIC.OUT_01_DIAG  SymbolName=DIAG_DigitalOutputsSTATIC_OUT_01_DIAG_000305  DataType=uint16  Init=1  Slope=1  Bias=0  DataSize=1  fpDataType=uint16  BlockIOType=Inport  DeviceType=0
  in_DIAG_DigitalOutputsSTATIC.OUT_01_SENSE_PULSE_DIAG : KIBES_Signal/KIBES_Signal  MBDS_LibraryBlock=on  DatabaseKey=2209  SignalName=DIAG_DigitalOutputsSTATIC.OUT_01_SENSE_PULSE_DIAG  SymbolName=DIAG_DigitalOutputsSTATIC_OUT_01_SENSE_PULSE_DIAG_002209  DataType=uint16  Init=1  Slope=1  Bias=0  DataSize=1  fpDataType=uint16  BlockIOType=Inport  DeviceType=0
  in_DIAG_DigitalOutputsSTATIC.OUT_01_TD_DIAG : KIBES_Signal/KIBES_Signal  MBDS_LibraryBlock=on  DatabaseKey=264  SignalName=DIAG_DigitalOutputsSTATIC.OUT_01_TD_DIAG  SymbolName=DIAG_DigitalOutputsSTATIC_OUT_01_TD_DIAG_000264  DataType=uint16  Init=1  Slope=1  Bias=0  DataSize=1  fpDataType=uint16  BlockIOType=Inport  DeviceType=0
  in_DIAG_DigitalOutputsSTATIC.OUT_02_DIAG : KIBES_Signal/KIBES_Signal  MBDS_LibraryBlock=on  DatabaseKey=250  SignalName=DIAG_DigitalOutputsSTATIC.OUT_02_DIAG  SymbolName=DIAG_DigitalOutputsSTATIC_OUT_02_DIAG_000250  DataType=uint16  Init=1  Slope=1  Bias=0  DataSize=1  fpDataType=uint16  BlockIOType=Inport  DeviceType=0
  in_DIAG_DigitalOutputsSTATIC.OUT_03_DIAG : KIBES_Signal/KIBES_Signal  MBDS_LibraryBlock=on  DatabaseKey=253  SignalName=DIAG_DigitalOutputsSTATIC.OUT_03_DIAG  SymbolName=DIAG_DigitalOutputsSTATIC_OUT_03_DIAG_000253  DataType=uint16  Init=1  Slope=1  Bias=0  DataSize=1  fpDataType=uint16  BlockIOType=Inport  DeviceType=0
  in_DIAG_DigitalOutputsSTATIC.OUT_04_DIAG : KIBES_Signal/KIBES_Signal  MBDS_LibraryBlock=on  DatabaseKey=256  SignalName=DIAG_DigitalOutputsSTATIC.OUT_04_DIAG  SymbolName=DIAG_DigitalOutputsSTATIC_OUT_04_DIAG_000256  DataType=uint16  Init=1  Slope=1  Bias=0  DataSize=1  fpDataType=uint16  BlockIOType=Inport  DeviceType=0
  in_DIAG_DigitalOutputsSTATIC.OUT_04_SENSE_PULSE_DIAG : KIBES_Signal/KIBES_Signal  MBDS_LibraryBlock=on  DatabaseKey=2211  SignalName=DIAG_DigitalOutputsSTATIC.OUT_04_SENSE_PULSE_DIAG  SymbolName=DIAG_DigitalOutputsSTATIC_OUT_04_SENSE_PULSE_DIAG_002211  DataType=uint16  Init=1  Slope=1  Bias=0  DataSize=1  fpDataType=uint16  BlockIOType=Inport  DeviceType=0
  in_DIAG_DigitalOutputsSTATIC.OUT_04_TD_DIAG : KIBES_Signal/KIBES_Signal  MBDS_LibraryBlock=on  DatabaseKey=319  SignalName=DIAG_DigitalOutputsSTATIC.OUT_04_TD_DIAG  SymbolName=DIAG_DigitalOutputsSTATIC_OUT_04_TD_DIAG_000319  DataType=uint16  Init=1  Slope=1  Bias=0  DataSize=1  fpDataType=uint16  BlockIOType=Inport  DeviceType=0
  in_DIAG_DigitalOutputsSTATIC.OUT_05_DIAG : KIBES_Signal/KIBES_Signal  MBDS_LibraryBlock=on  DatabaseKey=259  SignalName=DIAG_DigitalOutputsSTATIC.OUT_05_DIAG  SymbolName=DIAG_DigitalOutputsSTATIC_OUT_05_DIAG_000259  DataType=uint16  Init=1  Slope=1  Bias=0  DataSize=1  fpDataType=uint16  BlockIOType=Inport  DeviceType=0
  in_DIAG_DigitalOutputsSTATIC.OUT_06_DIAG : KIBES_Signal/KIBES_Signal  MBDS_LibraryBlock=on  DatabaseKey=262  SignalName=DIAG_DigitalOutputsSTATIC.OUT_06_DIAG  SymbolName=DIAG_DigitalOutputsSTATIC_OUT_06_DIAG_000262  DataType=uint16  Init=1  Slope=1  Bias=0  DataSize=1  fpDataType=uint16  BlockIOType=Inport  DeviceType=0
  in_DIAG_DigitalOutputsSTATIC.OUT_06_SENSE_PULSE_DIAG : KIBES_Signal/KIBES_Signal  MBDS_LibraryBlock=on  DatabaseKey=2203  SignalName=DIAG_DigitalOutputsSTATIC.OUT_06_SENSE_PULSE_DIAG  SymbolName=DIAG_DigitalOutputsSTATIC_OUT_06_SENSE_PULSE_DIAG_002203  DataType=uint16  Init=1  Slope=1  Bias=0  DataSize=1  fpDataType=uint16  BlockIOType=Inport  DeviceType=0
  in_DIAG_DigitalOutputsSTATIC.OUT_06_TD_DIAG : KIBES_Signal/KIBES_Signal  MBDS_LibraryBlock=on  DatabaseKey=287  SignalName=DIAG_DigitalOutputsSTATIC.OUT_06_TD_DIAG  SymbolName=DIAG_DigitalOutputsSTATIC_OUT_06_TD_DIAG_000287  DataType=uint16  Init=1  Slope=1  Bias=0  DataSize=1  fpDataType=uint16  BlockIOType=Inport  DeviceType=0
  in_DIAG_DigitalOutputsSTATIC.OUT_07_DIAG : KIBES_Signal/KIBES_Signal  MBDS_LibraryBlock=on  DatabaseKey=289  SignalName=DIAG_DigitalOutputsSTATIC.OUT_07_DIAG  SymbolName=DIAG_DigitalOutputsSTATIC_OUT_07_DIAG_000289  DataType=uint16  Init=1  Slope=1  Bias=0  DataSize=1  fpDataType=uint16  BlockIOType=Inport  DeviceType=0
  in_DIAG_DigitalOutputsSTATIC.OUT_07_SENSE_PULSE_DIAG : KIBES_Signal/KIBES_Signal  MBDS_LibraryBlock=on  DatabaseKey=2205  SignalName=DIAG_DigitalOutputsSTATIC.OUT_07_SENSE_PULSE_DIAG  SymbolName=DIAG_DigitalOutputsSTATIC_OUT_07_SENSE_PULSE_DIAG_002205  DataType=uint16  Init=1  Slope=1  Bias=0  DataSize=1  fpDataType=uint16  BlockIOType=Inport  DeviceType=0
  in_DIAG_DigitalOutputsSTATIC.OUT_07_TD_DIAG : KIBES_Signal/KIBES_Signal  MBDS_LibraryBlock=on  DatabaseKey=294  SignalName=DIAG_DigitalOutputsSTATIC.OUT_07_TD_DIAG  SymbolName=DIAG_DigitalOutputsSTATIC_OUT_07_TD_DIAG_000294  DataType=uint16  Init=1  Slope=1  Bias=0  DataSize=1  fpDataType=uint16  BlockIOType=Inport  DeviceType=0
  in_DIAG_DigitalOutputsSTATIC.OUT_08_DIAG : KIBES_Signal/KIBES_Signal  MBDS_LibraryBlock=on  DatabaseKey=298  SignalName=DIAG_DigitalOutputsSTATIC.OUT_08_DIAG  SymbolName=DIAG_DigitalOutputsSTATIC_OUT_08_DIAG_000298  DataType=uint16  Init=1  Slope=1  Bias=0  DataSize=1  fpDataType=uint16  BlockIOType=Inport  DeviceType=0
  in_DIAG_DigitalOutputsSTATIC.OUT_08_SENSE_PULSE_DIAG : KIBES_Signal/KIBES_Signal  MBDS_LibraryBlock=on  DatabaseKey=2207  SignalName=DIAG_DigitalOutputsSTATIC.OUT_08_SENSE_PULSE_DIAG  SymbolName=DIAG_DigitalOutputsSTATIC_OUT_08_SENSE_PULSE_DIAG_002207  DataType=uint16  Init=1  Slope=1  Bias=0  DataSize=1  fpDataType=uint16  BlockIOType=Inport  DeviceType=0
  in_DIAG_DigitalOutputsSTATIC.OUT_08_TD_DIAG : KIBES_Signal/KIBES_Signal  MBDS_LibraryBlock=on  DatabaseKey=303  SignalName=DIAG_DigitalOutputsSTATIC.OUT_08_TD_DIAG  SymbolName=DIAG_DigitalOutputsSTATIC_OUT_08_TD_DIAG_000303  DataType=uint16  Init=1  Slope=1  Bias=0  DataSize=1  fpDataType=uint16  BlockIOType=Inport  DeviceType=0
  in_DIAG_DigitalOutputsSTATIC.OUT_09_DIAG : KIBES_Signal/KIBES_Signal  MBDS_LibraryBlock=on  DatabaseKey=265  SignalName=DIAG_DigitalOutputsSTATIC.OUT_09_DIAG  SymbolName=DIAG_DigitalOutputsSTATIC_OUT_09_DIAG_000265  DataType=uint16  Init=1  Slope=1  Bias=0  DataSize=1  fpDataType=uint16  BlockIOType=Inport  DeviceType=0
  in_DIAG_DigitalOutputsSTATIC.OUT_10_DIAG : KIBES_Signal/KIBES_Signal  MBDS_LibraryBlock=on  DatabaseKey=269  SignalName=DIAG_DigitalOutputsSTATIC.OUT_10_DIAG  SymbolName=DIAG_DigitalOutputsSTATIC_OUT_10_DIAG_000269  DataType=uint16  Init=1  Slope=1  Bias=0  DataSize=1  fpDataType=uint16  BlockIOType=Inport  DeviceType=0
  in_DIAG_DigitalOutputsSTATIC.OUT_11_DIAG : KIBES_Signal/KIBES_Signal  MBDS_LibraryBlock=on  DatabaseKey=272  SignalName=DIAG_DigitalOutputsSTATIC.OUT_11_DIAG  SymbolName=DIAG_DigitalOutputsSTATIC_OUT_11_DIAG_000272  DataType=uint16  Init=1  Slope=1  Bias=0  DataSize=1  fpDataType=uint16  BlockIOType=Inport  DeviceType=0
  in_DIAG_DigitalOutputsSTATIC.OUT_12_DIAG : KIBES_Signal/KIBES_Signal  MBDS_LibraryBlock=on  DatabaseKey=284  SignalName=DIAG_DigitalOutputsSTATIC.OUT_12_DIAG  SymbolName=DIAG_DigitalOutputsSTATIC_OUT_12_DIAG_000284  DataType=uint16  Init=1  Slope=1  Bias=0  DataSize=1  fpDataType=uint16  BlockIOType=Inport  DeviceType=0
  in_DIAG_DigitalOutputsSTATIC.OUT_12_SENSE_PULSE_DIAG : KIBES_Signal/KIBES_Signal  MBDS_LibraryBlock=on  DatabaseKey=2213  SignalName=DIAG_DigitalOutputsSTATIC.OUT_12_SENSE_PULSE_DIAG  SymbolName=DIAG_DigitalOutputsSTATIC_OUT_12_SENSE_PULSE_DIAG_002213  DataType=uint16  Init=1  Slope=1  Bias=0  DataSize=1  fpDataType=uint16  BlockIOType=Inport  DeviceType=0
  in_DIAG_DigitalOutputsSTATIC.OUT_12_TD_DIAG : KIBES_Signal/KIBES_Signal  MBDS_LibraryBlock=on  DatabaseKey=325  SignalName=DIAG_DigitalOutputsSTATIC.OUT_12_TD_DIAG  SymbolName=DIAG_DigitalOutputsSTATIC_OUT_12_TD_DIAG_000325  DataType=uint16  Init=1  Slope=1  Bias=0  DataSize=1  fpDataType=uint16  BlockIOType=Inport  DeviceType=0
  in_DIAG_DigitalOutputsSTATIC.OUT_13_DIAG : KIBES_Signal/KIBES_Signal  MBDS_LibraryBlock=on  DatabaseKey=327  SignalName=DIAG_DigitalOutputsSTATIC.OUT_13_DIAG  SymbolName=DIAG_DigitalOutputsSTATIC_OUT_13_DIAG_000327  DataType=uint16  Init=1  Slope=1  Bias=0  DataSize=1  fpDataType=uint16  BlockIOType=Inport  DeviceType=0
  in_DIAG_DigitalOutputsSTATIC.OUT_13_SENSE_PULSE_DIAG : KIBES_Signal/KIBES_Signal  MBDS_LibraryBlock=on  DatabaseKey=2215  SignalName=DIAG_DigitalOutputsSTATIC.OUT_13_SENSE_PULSE_DIAG  SymbolName=DIAG_DigitalOutputsSTATIC_OUT_13_SENSE_PULSE_DIAG_002215  DataType=uint16  Init=1  Slope=1  Bias=0  DataSize=1  fpDataType=uint16  BlockIOType=Inport  DeviceType=0
  in_DIAG_DigitalOutputsSTATIC.OUT_13_TD_DIAG : KIBES_Signal/KIBES_Signal  MBDS_LibraryBlock=on  DatabaseKey=332  SignalName=DIAG_DigitalOutputsSTATIC.OUT_13_TD_DIAG  SymbolName=DIAG_DigitalOutputsSTATIC_OUT_13_TD_DIAG_000332  DataType=uint16  Init=1  Slope=1  Bias=0  DataSize=1  fpDataType=uint16  BlockIOType=Inport  DeviceType=0
  in_DIAG_DigitalOutputsSTATIC.OUT_14_DIAG : KIBES_Signal/KIBES_Signal  MBDS_LibraryBlock=on  DatabaseKey=334  SignalName=DIAG_DigitalOutputsSTATIC.OUT_14_DIAG  SymbolName=DIAG_DigitalOutputsSTATIC_OUT_14_DIAG_000334  DataType=uint16  Init=1  Slope=1  Bias=0  DataSize=1  fpDataType=uint16  BlockIOType=Inport  DeviceType=0
  in_DIAG_DigitalOutputsSTATIC.OUT_14_SENSE_PULSE_DIAG : KIBES_Signal/KIBES_Signal  MBDS_LibraryBlock=on  DatabaseKey=2217  SignalName=DIAG_DigitalOutputsSTATIC.OUT_14_SENSE_PULSE_DIAG  SymbolName=DIAG_DigitalOutputsSTATIC_OUT_14_SENSE_PULSE_DIAG_002217  DataType=uint16  Init=1  Slope=1  Bias=0  DataSize=1  fpDataType=uint16  BlockIOType=Inport  DeviceType=0
  in_DIAG_DigitalOutputsSTATIC.OUT_14_TD_DIAG : KIBES_Signal/KIBES_Signal  MBDS_LibraryBlock=on  DatabaseKey=339  SignalName=DIAG_DigitalOutputsSTATIC.OUT_14_TD_DIAG  SymbolName=DIAG_DigitalOutputsSTATIC_OUT_14_TD_DIAG_000339  DataType=uint16  Init=1  Slope=1  Bias=0  DataSize=1  fpDataType=uint16  BlockIOType=Inport  DeviceType=0
  in_DIAG_DigitalOutputsSTATIC.OUT_15_DIAG : KIBES_Signal/KIBES_Signal  MBDS_LibraryBlock=on  DatabaseKey=344  SignalName=DIAG_DigitalOutputsSTATIC.OUT_15_DIAG  SymbolName=DIAG_DigitalOutputsSTATIC_OUT_15_DIAG_000344  DataType=uint16  Init=1  Slope=1  Bias=0  DataSize=1  fpDataType=uint16  BlockIOType=Inport  DeviceType=0
  in_DIAG_DigitalOutputsSTATIC.OUT_15_SENSE_PULSE_DIAG : KIBES_Signal/KIBES_Signal  MBDS_LibraryBlock=on  DatabaseKey=2219  SignalName=DIAG_DigitalOutputsSTATIC.OUT_15_SENSE_PULSE_DIAG  SymbolName=DIAG_DigitalOutputsSTATIC_OUT_15_SENSE_PULSE_DIAG_002219  DataType=uint16  Init=1  Slope=1  Bias=0  DataSize=1  fpDataType=uint16  BlockIOType=Inport  DeviceType=0
  in_DIAG_DigitalOutputsSTATIC.OUT_15_TD_DIAG : KIBES_Signal/KIBES_Signal  MBDS_LibraryBlock=on  DatabaseKey=349  SignalName=DIAG_DigitalOutputsSTATIC.OUT_15_TD_DIAG  SymbolName=DIAG_DigitalOutputsSTATIC_OUT_15_TD_DIAG_000349  DataType=uint16  Init=1  Slope=1  Bias=0  DataSize=1  fpDataType=uint16  BlockIOType=Inport  DeviceType=0
  in_DIAG_DigitalOutputsSTATIC.OUT_16_DIAG : KIBES_Signal/KIBES_Signal  MBDS_LibraryBlock=on  DatabaseKey=275  SignalName=DIAG_DigitalOutputsSTATIC.OUT_16_DIAG  SymbolName=DIAG_DigitalOutputsSTATIC_OUT_16_DIAG_000275  DataType=uint16  Init=1  Slope=1  Bias=0  DataSize=1  fpDataType=uint16  BlockIOType=Inport  DeviceType=0
  in_DIAG_DigitalOutputsSTATIC.OUT_17_DIAG : KIBES_Signal/KIBES_Signal  MBDS_LibraryBlock=on  DatabaseKey=278  SignalName=DIAG_DigitalOutputsSTATIC.OUT_17_DIAG  SymbolName=DIAG_DigitalOutputsSTATIC_OUT_17_DIAG_000278  DataType=uint16  Init=1  Slope=1  Bias=0  DataSize=1  fpDataType=uint16  BlockIOType=Inport  DeviceType=0
  in_DIAG_DigitalOutputsSTATIC.OUT_19_DIAG : KIBES_Signal/KIBES_Signal  MBDS_LibraryBlock=on  DatabaseKey=310  SignalName=DIAG_DigitalOutputsSTATIC.OUT_19_DIAG  SymbolName=DIAG_DigitalOutputsSTATIC_OUT_19_DIAG_000310  DataType=uint16  Init=1  Slope=1  Bias=0  DataSize=1  fpDataType=uint16  BlockIOType=Inport  DeviceType=0
  in_IN_DigitalOutputsSTATIC.OUT_01_SENSE : KIBES_Signal/KIBES_Signal  MBDS_LibraryBlock=on  DatabaseKey=306  SignalName=IN_DigitalOutputsSTATIC.OUT_01_SENSE  SymbolName=IN_DigitalOutputsSTATIC_OUT_01_SENSE_000306  DataType=uint16  Init=0  Slope=1  Bias=0  DataSize=1  fpDataType=uint16  BlockIOType=Inport  DeviceType=0
  in_IN_DigitalOutputsSTATIC.OUT_01_SENSE_PULSE : KIBES_Signal/KIBES_Signal  MBDS_LibraryBlock=on  DatabaseKey=2208  SignalName=IN_DigitalOutputsSTATIC.OUT_01_SENSE_PULSE  SymbolName=IN_DigitalOutputsSTATIC_OUT_01_SENSE_PULSE_002208  DataType=uint16  Init=0  Slope=1  Bias=0  DataSize=1  fpDataType=uint16  BlockIOType=Inport  DeviceType=0
  in_IN_DigitalOutputsSTATIC.OUT_01_TD : KIBES_Signal/KIBES_Signal  MBDS_LibraryBlock=on  DatabaseKey=314  SignalName=IN_DigitalOutputsSTATIC.OUT_01_TD  SymbolName=IN_DigitalOutputsSTATIC_OUT_01_TD_000314  DataType=boolean  Init=0  Slope=1  Bias=0  DataSize=1  fpDataType=boolean  BlockIOType=Inport  DeviceType=0
  in_IN_DigitalOutputsSTATIC.OUT_02_SENSE : KIBES_Signal/KIBES_Signal  MBDS_LibraryBlock=on  DatabaseKey=251  SignalName=IN_DigitalOutputsSTATIC.OUT_02_SENSE  SymbolName=IN_DigitalOutputsSTATIC_OUT_02_SENSE_000251  DataType=uint16  Init=0  Slope=1  Bias=0  DataSize=1  fpDataType=uint16  BlockIOType=Inport  DeviceType=0
  in_IN_DigitalOutputsSTATIC.OUT_03_SENSE : KIBES_Signal/KIBES_Signal  MBDS_LibraryBlock=on  DatabaseKey=254  SignalName=IN_DigitalOutputsSTATIC.OUT_03_SENSE  SymbolName=IN_DigitalOutputsSTATIC_OUT_03_SENSE_000254  DataType=uint16  Init=0  Slope=1  Bias=0  DataSize=1  fpDataType=uint16  BlockIOType=Inport  DeviceType=0
  in_IN_DigitalOutputsSTATIC.OUT_04_SENSE : KIBES_Signal/KIBES_Signal  MBDS_LibraryBlock=on  DatabaseKey=257  SignalName=IN_DigitalOutputsSTATIC.OUT_04_SENSE  SymbolName=IN_DigitalOutputsSTATIC_OUT_04_SENSE_000257  DataType=uint16  Init=0  Slope=1  Bias=0  DataSize=1  fpDataType=uint16  BlockIOType=Inport  DeviceType=0
  in_IN_DigitalOutputsSTATIC.OUT_04_SENSE_PULSE : KIBES_Signal/KIBES_Signal  MBDS_LibraryBlock=on  DatabaseKey=2210  SignalName=IN_DigitalOutputsSTATIC.OUT_04_SENSE_PULSE  SymbolName=IN_DigitalOutputsSTATIC_OUT_04_SENSE_PULSE_002210  DataType=uint16  Init=0  Slope=1  Bias=0  DataSize=1  fpDataType=uint16  BlockIOType=Inport  DeviceType=0
  in_IN_DigitalOutputsSTATIC.OUT_04_TD : KIBES_Signal/KIBES_Signal  MBDS_LibraryBlock=on  DatabaseKey=318  SignalName=IN_DigitalOutputsSTATIC.OUT_04_TD  SymbolName=IN_DigitalOutputsSTATIC_OUT_04_TD_000318  DataType=boolean  Init=0  Slope=1  Bias=0  DataSize=1  fpDataType=boolean  BlockIOType=Inport  DeviceType=0
  in_IN_DigitalOutputsSTATIC.OUT_05_SENSE : KIBES_Signal/KIBES_Signal  MBDS_LibraryBlock=on  DatabaseKey=260  SignalName=IN_DigitalOutputsSTATIC.OUT_05_SENSE  SymbolName=IN_DigitalOutputsSTATIC_OUT_05_SENSE_000260  DataType=uint16  Init=0  Slope=1  Bias=0  DataSize=1  fpDataType=uint16  BlockIOType=Inport  DeviceType=0
  in_IN_DigitalOutputsSTATIC.OUT_06_SENSE : KIBES_Signal/KIBES_Signal  MBDS_LibraryBlock=on  DatabaseKey=263  SignalName=IN_DigitalOutputsSTATIC.OUT_06_SENSE  SymbolName=IN_DigitalOutputsSTATIC_OUT_06_SENSE_000263  DataType=uint16  Init=0  Slope=1  Bias=0  DataSize=1  fpDataType=uint16  BlockIOType=Inport  DeviceType=0
  in_IN_DigitalOutputsSTATIC.OUT_06_SENSE_PULSE : KIBES_Signal/KIBES_Signal  MBDS_LibraryBlock=on  DatabaseKey=2202  SignalName=IN_DigitalOutputsSTATIC.OUT_06_SENSE_PULSE  SymbolName=IN_DigitalOutputsSTATIC_OUT_06_SENSE_PULSE_002202  DataType=uint16  Init=0  Slope=1  Bias=0  DataSize=1  fpDataType=uint16  BlockIOType=Inport  DeviceType=0
  in_IN_DigitalOutputsSTATIC.OUT_06_TD : KIBES_Signal/KIBES_Signal  MBDS_LibraryBlock=on  DatabaseKey=286  SignalName=IN_DigitalOutputsSTATIC.OUT_06_TD  SymbolName=IN_DigitalOutputsSTATIC_OUT_06_TD_000286  DataType=boolean  Init=0  Slope=1  Bias=0  DataSize=1  fpDataType=boolean  BlockIOType=Inport  DeviceType=0
  in_IN_DigitalOutputsSTATIC.OUT_07_SENSE : KIBES_Signal/KIBES_Signal  MBDS_LibraryBlock=on  DatabaseKey=290  SignalName=IN_DigitalOutputsSTATIC.OUT_07_SENSE  SymbolName=IN_DigitalOutputsSTATIC_OUT_07_SENSE_000290  DataType=uint16  Init=0  Slope=1  Bias=0  DataSize=1  fpDataType=uint16  BlockIOType=Inport  DeviceType=0
  in_IN_DigitalOutputsSTATIC.OUT_07_SENSE_PULSE : KIBES_Signal/KIBES_Signal  MBDS_LibraryBlock=on  DatabaseKey=2204  SignalName=IN_DigitalOutputsSTATIC.OUT_07_SENSE_PULSE  SymbolName=IN_DigitalOutputsSTATIC_OUT_07_SENSE_PULSE_002204  DataType=uint16  Init=0  Slope=1  Bias=0  DataSize=1  fpDataType=uint16  BlockIOType=Inport  DeviceType=0
  in_IN_DigitalOutputsSTATIC.OUT_07_TD : KIBES_Signal/KIBES_Signal  MBDS_LibraryBlock=on  DatabaseKey=293  SignalName=IN_DigitalOutputsSTATIC.OUT_07_TD  SymbolName=IN_DigitalOutputsSTATIC_OUT_07_TD_000293  DataType=boolean  Init=0  Slope=1  Bias=0  DataSize=1  fpDataType=boolean  BlockIOType=Inport  DeviceType=0
  in_IN_DigitalOutputsSTATIC.OUT_08_SENSE : KIBES_Signal/KIBES_Signal  MBDS_LibraryBlock=on  DatabaseKey=299  SignalName=IN_DigitalOutputsSTATIC.OUT_08_SENSE  SymbolName=IN_DigitalOutputsSTATIC_OUT_08_SENSE_000299  DataType=uint16  Init=0  Slope=1  Bias=0  DataSize=1  fpDataType=uint16  BlockIOType=Inport  DeviceType=0
  in_IN_DigitalOutputsSTATIC.OUT_08_SENSE_PULSE : KIBES_Signal/KIBES_Signal  MBDS_LibraryBlock=on  DatabaseKey=2206  SignalName=IN_DigitalOutputsSTATIC.OUT_08_SENSE_PULSE  SymbolName=IN_DigitalOutputsSTATIC_OUT_08_SENSE_PULSE_002206  DataType=uint16  Init=0  Slope=1  Bias=0  DataSize=1  fpDataType=uint16  BlockIOType=Inport  DeviceType=0
  in_IN_DigitalOutputsSTATIC.OUT_08_TD : KIBES_Signal/KIBES_Signal  MBDS_LibraryBlock=on  DatabaseKey=302  SignalName=IN_DigitalOutputsSTATIC.OUT_08_TD  SymbolName=IN_DigitalOutputsSTATIC_OUT_08_TD_000302  DataType=boolean  Init=0  Slope=1  Bias=0  DataSize=1  fpDataType=boolean  BlockIOType=Inport  DeviceType=0
  in_IN_DigitalOutputsSTATIC.OUT_09_SENSE : KIBES_Signal/KIBES_Signal  MBDS_LibraryBlock=on  DatabaseKey=267  SignalName=IN_DigitalOutputsSTATIC.OUT_09_SENSE  SymbolName=IN_DigitalOutputsSTATIC_OUT_09_SENSE_000267  DataType=uint16  Init=0  Slope=1  Bias=0  DataSize=1  fpDataType=uint16  BlockIOType=Inport  DeviceType=0
  in_IN_DigitalOutputsSTATIC.OUT_10_SENSE : KIBES_Signal/KIBES_Signal  MBDS_LibraryBlock=on  DatabaseKey=270  SignalName=IN_DigitalOutputsSTATIC.OUT_10_SENSE  SymbolName=IN_DigitalOutputsSTATIC_OUT_10_SENSE_000270  DataType=uint16  Init=0  Slope=1  Bias=0  DataSize=1  fpDataType=uint16  BlockIOType=Inport  DeviceType=0
  in_IN_DigitalOutputsSTATIC.OUT_11_SENSE : KIBES_Signal/KIBES_Signal  MBDS_LibraryBlock=on  DatabaseKey=273  SignalName=IN_DigitalOutputsSTATIC.OUT_11_SENSE  SymbolName=IN_DigitalOutputsSTATIC_OUT_11_SENSE_000273  DataType=uint16  Init=0  Slope=1  Bias=0  DataSize=1  fpDataType=uint16  BlockIOType=Inport  DeviceType=0
  in_IN_DigitalOutputsSTATIC.OUT_12_SENSE : KIBES_Signal/KIBES_Signal  MBDS_LibraryBlock=on  DatabaseKey=285  SignalName=IN_DigitalOutputsSTATIC.OUT_12_SENSE  SymbolName=IN_DigitalOutputsSTATIC_OUT_12_SENSE_000285  DataType=uint16  Init=0  Slope=1  Bias=0  DataSize=1  fpDataType=uint16  BlockIOType=Inport  DeviceType=0
  in_IN_DigitalOutputsSTATIC.OUT_12_SENSE_PULSE : KIBES_Signal/KIBES_Signal  MBDS_LibraryBlock=on  DatabaseKey=2212  SignalName=IN_DigitalOutputsSTATIC.OUT_12_SENSE_PULSE  SymbolName=IN_DigitalOutputsSTATIC_OUT_12_SENSE_PULSE_002212  DataType=uint16  Init=0  Slope=1  Bias=0  DataSize=1  fpDataType=uint16  BlockIOType=Inport  DeviceType=0
  in_IN_DigitalOutputsSTATIC.OUT_12_TD : KIBES_Signal/KIBES_Signal  MBDS_LibraryBlock=on  DatabaseKey=324  SignalName=IN_DigitalOutputsSTATIC.OUT_12_TD  SymbolName=IN_DigitalOutputsSTATIC_OUT_12_TD_000324  DataType=boolean  Init=0  Slope=1  Bias=0  DataSize=1  fpDataType=boolean  BlockIOType=Inport  DeviceType=0
  in_IN_DigitalOutputsSTATIC.OUT_13_SENSE : KIBES_Signal/KIBES_Signal  MBDS_LibraryBlock=on  DatabaseKey=328  SignalName=IN_DigitalOutputsSTATIC.OUT_13_SENSE  SymbolName=IN_DigitalOutputsSTATIC_OUT_13_SENSE_000328  DataType=uint16  Init=0  Slope=1  Bias=0  DataSize=1  fpDataType=uint16  BlockIOType=Inport  DeviceType=0
  in_IN_DigitalOutputsSTATIC.OUT_13_SENSE_PULSE : KIBES_Signal/KIBES_Signal  MBDS_LibraryBlock=on  DatabaseKey=2214  SignalName=IN_DigitalOutputsSTATIC.OUT_13_SENSE_PULSE  SymbolName=IN_DigitalOutputsSTATIC_OUT_13_SENSE_PULSE_002214  DataType=uint16  Init=0  Slope=1  Bias=0  DataSize=1  fpDataType=uint16  BlockIOType=Inport  DeviceType=0
  in_IN_DigitalOutputsSTATIC.OUT_13_TD : KIBES_Signal/KIBES_Signal  MBDS_LibraryBlock=on  DatabaseKey=331  SignalName=IN_DigitalOutputsSTATIC.OUT_13_TD  SymbolName=IN_DigitalOutputsSTATIC_OUT_13_TD_000331  DataType=boolean  Init=0  Slope=1  Bias=0  DataSize=1  fpDataType=boolean  BlockIOType=Inport  DeviceType=0
  in_IN_DigitalOutputsSTATIC.OUT_14_SENSE : KIBES_Signal/KIBES_Signal  MBDS_LibraryBlock=on  DatabaseKey=335  SignalName=IN_DigitalOutputsSTATIC.OUT_14_SENSE  SymbolName=IN_DigitalOutputsSTATIC_OUT_14_SENSE_000335  DataType=uint16  Init=0  Slope=1  Bias=0  DataSize=1  fpDataType=uint16  BlockIOType=Inport  DeviceType=0
  in_IN_DigitalOutputsSTATIC.OUT_14_SENSE_PULSE : KIBES_Signal/KIBES_Signal  MBDS_LibraryBlock=on  DatabaseKey=2216  SignalName=IN_DigitalOutputsSTATIC.OUT_14_SENSE_PULSE  SymbolName=IN_DigitalOutputsSTATIC_OUT_14_SENSE_PULSE_002216  DataType=uint16  Init=0  Slope=1  Bias=0  DataSize=1  fpDataType=uint16  BlockIOType=Inport  DeviceType=0
  in_IN_DigitalOutputsSTATIC.OUT_14_TD : KIBES_Signal/KIBES_Signal  MBDS_LibraryBlock=on  DatabaseKey=338  SignalName=IN_DigitalOutputsSTATIC.OUT_14_TD  SymbolName=IN_DigitalOutputsSTATIC_OUT_14_TD_000338  DataType=boolean  Init=0  Slope=1  Bias=0  DataSize=1  fpDataType=boolean  BlockIOType=Inport  DeviceType=0
  in_IN_DigitalOutputsSTATIC.OUT_15_SENSE : KIBES_Signal/KIBES_Signal  MBDS_LibraryBlock=on  DatabaseKey=345  SignalName=IN_DigitalOutputsSTATIC.OUT_15_SENSE  SymbolName=IN_DigitalOutputsSTATIC_OUT_15_SENSE_000345  DataType=uint16  Init=0  Slope=1  Bias=0  DataSize=1  fpDataType=uint16  BlockIOType=Inport  DeviceType=0
  in_IN_DigitalOutputsSTATIC.OUT_15_SENSE_PULSE : KIBES_Signal/KIBES_Signal  MBDS_LibraryBlock=on  DatabaseKey=2218  SignalName=IN_DigitalOutputsSTATIC.OUT_15_SENSE_PULSE  SymbolName=IN_DigitalOutputsSTATIC_OUT_15_SENSE_PULSE_002218  DataType=uint16  Init=0  Slope=1  Bias=0  DataSize=1  fpDataType=uint16  BlockIOType=Inport  DeviceType=0
  in_IN_DigitalOutputsSTATIC.OUT_15_TD : KIBES_Signal/KIBES_Signal  MBDS_LibraryBlock=on  DatabaseKey=348  SignalName=IN_DigitalOutputsSTATIC.OUT_15_TD  SymbolName=IN_DigitalOutputsSTATIC_OUT_15_TD_000348  DataType=boolean  Init=0  Slope=1  Bias=0  DataSize=1  fpDataType=boolean  BlockIOType=Inport  DeviceType=0
  in_IN_DigitalOutputsSTATIC.OUT_16_SENSE : KIBES_Signal/KIBES_Signal  MBDS_LibraryBlock=on  DatabaseKey=276  SignalName=IN_DigitalOutputsSTATIC.OUT_16_SENSE  SymbolName=IN_DigitalOutputsSTATIC_OUT_16_SENSE_000276  DataType=uint16  Init=0  Slope=1  Bias=0  DataSize=1  fpDataType=uint16  BlockIOType=Inport  DeviceType=0
  in_IN_DigitalOutputsSTATIC.OUT_17_SENSE : KIBES_Signal/KIBES_Signal  MBDS_LibraryBlock=on  DatabaseKey=279  SignalName=IN_DigitalOutputsSTATIC.OUT_17_SENSE  SymbolName=IN_DigitalOutputsSTATIC_OUT_17_SENSE_000279  DataType=uint16  Init=0  Slope=1  Bias=0  DataSize=1  fpDataType=uint16  BlockIOType=Inport  DeviceType=0
  in_IN_DigitalOutputsSTATIC.OUT_19_SENSE : KIBES_Signal/KIBES_Signal  MBDS_LibraryBlock=on  DatabaseKey=311  SignalName=IN_DigitalOutputsSTATIC.OUT_19_SENSE  SymbolName=IN_DigitalOutputsSTATIC_OUT_19_SENSE_000311  DataType=uint16  Init=0  Slope=1  Bias=0  DataSize=1  fpDataType=uint16  BlockIOType=Inport  DeviceType=0
  in_IN_NVM.Parameter.BlinkSourcePeriod : KIBES_Signal/KIBES_Signal  MBDS_LibraryBlock=on  DatabaseKey=2687  SignalName=IN_NVM.Parameter.BlinkSourcePeriod  SymbolName=IN_NVM_Parameter_BlinkSourcePeriod_002687  DataType=uint16  Init=12  Slope=1  Bias=0  DataSize=1  fpDataType=uint16  BlockIOType=Inport  DeviceType=0
  in_IN_NVM.Parameter.TrailerDetectionTime : KIBES_Signal/KIBES_Signal  MBDS_LibraryBlock=on  DatabaseKey=2695  SignalName=IN_NVM.Parameter.TrailerDetectionTime  SymbolName=IN_NVM_Parameter_TrailerDetectionTime_002695  DataType=uint8  Init=2  Slope=1  Bias=0  DataSize=1  fpDataType=uint8  BlockIOType=Inport  DeviceType=0
  in_IN_PCAN.Rx_Ctrl.Out_Ctrl.MessageState : KIBES_Signal/KIBES_Signal  MBDS_LibraryBlock=on  DatabaseKey=1715  SignalName=IN_PCAN.Rx_Ctrl.Out_Ctrl.MessageState  SymbolName=IN_PCAN_Rx_Ctrl_Out_Ctrl_MessageState_001715  DataType=uint16  Init=0  Slope=1  Bias=0  DataSize=1  fpDataType=uint16  BlockIOType=Inport  DeviceType=0
  in_IN_PCAN.Rx_Ctrl.Out_Ctrl.Out_01_Ctrl : KIBES_Signal/KIBES_Signal  MBDS_LibraryBlock=on  DatabaseKey=1703  SignalName=IN_PCAN.Rx_Ctrl.Out_Ctrl.Out_01_Ctrl  SymbolName=IN_PCAN_Rx_Ctrl_Out_Ctrl_Out_01_Ctrl_001703  DataType=boolean  Init=0  Slope=1  Bias=0  DataSize=1  fpDataType=boolean  BlockIOType=Inport  DeviceType=0
  in_IN_PCAN.Rx_Ctrl.Out_Ctrl.Out_02_Ctrl : KIBES_Signal/KIBES_Signal  MBDS_LibraryBlock=on  DatabaseKey=1702  SignalName=IN_PCAN.Rx_Ctrl.Out_Ctrl.Out_02_Ctrl  SymbolName=IN_PCAN_Rx_Ctrl_Out_Ctrl_Out_02_Ctrl_001702  DataType=boolean  Init=0  Slope=1  Bias=0  DataSize=1  fpDataType=boolean  BlockIOType=Inport  DeviceType=0
  in_IN_PCAN.Rx_Ctrl.Out_Ctrl.Out_03_Ctrl : KIBES_Signal/KIBES_Signal  MBDS_LibraryBlock=on  DatabaseKey=1701  SignalName=IN_PCAN.Rx_Ctrl.Out_Ctrl.Out_03_Ctrl  SymbolName=IN_PCAN_Rx_Ctrl_Out_Ctrl_Out_03_Ctrl_001701  DataType=boolean  Init=0  Slope=1  Bias=0  DataSize=1  fpDataType=boolean  BlockIOType=Inport  DeviceType=0
  in_IN_PCAN.Rx_Ctrl.Out_Ctrl.Out_04_Ctrl : KIBES_Signal/KIBES_Signal  MBDS_LibraryBlock=on  DatabaseKey=1700  SignalName=IN_PCAN.Rx_Ctrl.Out_Ctrl.Out_04_Ctrl  SymbolName=IN_PCAN_Rx_Ctrl_Out_Ctrl_Out_04_Ctrl_001700  DataType=boolean  Init=0  Slope=1  Bias=0  DataSize=1  fpDataType=boolean  BlockIOType=Inport  DeviceType=0
  in_IN_PCAN.Rx_Ctrl.Out_Ctrl.Out_05_Ctrl : KIBES_Signal/KIBES_Signal  MBDS_LibraryBlock=on  DatabaseKey=1699  SignalName=IN_PCAN.Rx_Ctrl.Out_Ctrl.Out_05_Ctrl  SymbolName=IN_PCAN_Rx_Ctrl_Out_Ctrl_Out_05_Ctrl_001699  DataType=boolean  Init=0  Slope=1  Bias=0  DataSize=1  fpDataType=boolean  BlockIOType=Inport  DeviceType=0
  in_IN_PCAN.Rx_Ctrl.Out_Ctrl.Out_06_Ctrl : KIBES_Signal/KIBES_Signal  MBDS_LibraryBlock=on  DatabaseKey=1698  SignalName=IN_PCAN.Rx_Ctrl.Out_Ctrl.Out_06_Ctrl  SymbolName=IN_PCAN_Rx_Ctrl_Out_Ctrl_Out_06_Ctrl_001698  DataType=boolean  Init=0  Slope=1  Bias=0  DataSize=1  fpDataType=boolean  BlockIOType=Inport  DeviceType=0
  in_IN_PCAN.Rx_Ctrl.Out_Ctrl.Out_07_Ctrl : KIBES_Signal/KIBES_Signal  MBDS_LibraryBlock=on  DatabaseKey=1697  SignalName=IN_PCAN.Rx_Ctrl.Out_Ctrl.Out_07_Ctrl  SymbolName=IN_PCAN_Rx_Ctrl_Out_Ctrl_Out_07_Ctrl_001697  DataType=boolean  Init=0  Slope=1  Bias=0  DataSize=1  fpDataType=boolean  BlockIOType=Inport  DeviceType=0
  in_IN_PCAN.Rx_Ctrl.Out_Ctrl.Out_08_Ctrl : KIBES_Signal/KIBES_Signal  MBDS_LibraryBlock=on  DatabaseKey=1696  SignalName=IN_PCAN.Rx_Ctrl.Out_Ctrl.Out_08_Ctrl  SymbolName=IN_PCAN_Rx_Ctrl_Out_Ctrl_Out_08_Ctrl_001696  DataType=boolean  Init=0  Slope=1  Bias=0  DataSize=1  fpDataType=boolean  BlockIOType=Inport  DeviceType=0
  in_IN_PCAN.Rx_Ctrl.Out_Ctrl.Out_09_Ctrl : KIBES_Signal/KIBES_Signal  MBDS_LibraryBlock=on  DatabaseKey=1695  SignalName=IN_PCAN.Rx_Ctrl.Out_Ctrl.Out_09_Ctrl  SymbolName=IN_PCAN_Rx_Ctrl_Out_Ctrl_Out_09_Ctrl_001695  DataType=boolean  Init=0  Slope=1  Bias=0  DataSize=1  fpDataType=boolean  BlockIOType=Inport  DeviceType=0
  in_IN_PCAN.Rx_Ctrl.Out_Ctrl.Out_10_Ctrl : KIBES_Signal/KIBES_Signal  MBDS_LibraryBlock=on  DatabaseKey=1694  SignalName=IN_PCAN.Rx_Ctrl.Out_Ctrl.Out_10_Ctrl  SymbolName=IN_PCAN_Rx_Ctrl_Out_Ctrl_Out_10_Ctrl_001694  DataType=boolean  Init=0  Slope=1  Bias=0  DataSize=1  fpDataType=boolean  BlockIOType=Inport  DeviceType=0
  in_IN_PCAN.Rx_Ctrl.Out_Ctrl.Out_11_Ctrl : KIBES_Signal/KIBES_Signal  MBDS_LibraryBlock=on  DatabaseKey=1693  SignalName=IN_PCAN.Rx_Ctrl.Out_Ctrl.Out_11_Ctrl  SymbolName=IN_PCAN_Rx_Ctrl_Out_Ctrl_Out_11_Ctrl_001693  DataType=boolean  Init=0  Slope=1  Bias=0  DataSize=1  fpDataType=boolean  BlockIOType=Inport  DeviceType=0
  in_IN_PCAN.Rx_Ctrl.Out_Ctrl.Out_12_Ctrl : KIBES_Signal/KIBES_Signal  MBDS_LibraryBlock=on  DatabaseKey=1692  SignalName=IN_PCAN.Rx_Ctrl.Out_Ctrl.Out_12_Ctrl  SymbolName=IN_PCAN_Rx_Ctrl_Out_Ctrl_Out_12_Ctrl_001692  DataType=boolean  Init=0  Slope=1  Bias=0  DataSize=1  fpDataType=boolean  BlockIOType=Inport  DeviceType=0
  in_IN_PCAN.Rx_Ctrl.Out_Ctrl.Out_13_Ctrl : KIBES_Signal/KIBES_Signal  MBDS_LibraryBlock=on  DatabaseKey=1691  SignalName=IN_PCAN.Rx_Ctrl.Out_Ctrl.Out_13_Ctrl  SymbolName=IN_PCAN_Rx_Ctrl_Out_Ctrl_Out_13_Ctrl_001691  DataType=boolean  Init=0  Slope=1  Bias=0  DataSize=1  fpDataType=boolean  BlockIOType=Inport  DeviceType=0
  in_IN_PCAN.Rx_Ctrl.Out_Ctrl.Out_14_Ctrl : KIBES_Signal/KIBES_Signal  MBDS_LibraryBlock=on  DatabaseKey=1690  SignalName=IN_PCAN.Rx_Ctrl.Out_Ctrl.Out_14_Ctrl  SymbolName=IN_PCAN_Rx_Ctrl_Out_Ctrl_Out_14_Ctrl_001690  DataType=boolean  Init=0  Slope=1  Bias=0  DataSize=1  fpDataType=boolean  BlockIOType=Inport  DeviceType=0
  in_IN_PCAN.Rx_Ctrl.Out_Ctrl.Out_15_Ctrl : KIBES_Signal/KIBES_Signal  MBDS_LibraryBlock=on  DatabaseKey=1689  SignalName=IN_PCAN.Rx_Ctrl.Out_Ctrl.Out_15_Ctrl  SymbolName=IN_PCAN_Rx_Ctrl_Out_Ctrl_Out_15_Ctrl_001689  DataType=boolean  Init=0  Slope=1  Bias=0  DataSize=1  fpDataType=boolean  BlockIOType=Inport  DeviceType=0
  in_IN_PCAN.Rx_Ctrl.Out_Ctrl.Out_16_Ctrl : KIBES_Signal/KIBES_Signal  MBDS_LibraryBlock=on  DatabaseKey=1688  SignalName=IN_PCAN.Rx_Ctrl.Out_Ctrl.Out_16_Ctrl  SymbolName=IN_PCAN_Rx_Ctrl_Out_Ctrl_Out_16_Ctrl_001688  DataType=boolean  Init=0  Slope=1  Bias=0  DataSize=1  fpDataType=boolean  BlockIOType=Inport  DeviceType=0
  in_IN_PCAN.Rx_Ctrl.Out_Ctrl.Out_17_Ctrl : KIBES_Signal/KIBES_Signal  MBDS_LibraryBlock=on  DatabaseKey=1687  SignalName=IN_PCAN.Rx_Ctrl.Out_Ctrl.Out_17_Ctrl  SymbolName=IN_PCAN_Rx_Ctrl_Out_Ctrl_Out_17_Ctrl_001687  DataType=boolean  Init=0  Slope=1  Bias=0  DataSize=1  fpDataType=boolean  BlockIOType=Inport  DeviceType=0
  in_IN_PCAN.Rx_Ctrl.Out_Ctrl.Out_19_Ctrl : KIBES_Signal/KIBES_Signal  MBDS_LibraryBlock=on  DatabaseKey=1685  SignalName=IN_PCAN.Rx_Ctrl.Out_Ctrl.Out_19_Ctrl  SymbolName=IN_PCAN_Rx_Ctrl_Out_Ctrl_Out_19_Ctrl_001685  DataType=boolean  Init=0  Slope=1  Bias=0  DataSize=1  fpDataType=boolean  BlockIOType=Inport  DeviceType=0
  in_IN_PCAN.Rx_Ctrl.Out_Ctrl.WorkingMode : KIBES_Signal/KIBES_Signal  MBDS_LibraryBlock=on  DatabaseKey=2686  SignalName=IN_PCAN.Rx_Ctrl.Out_Ctrl.WorkingMode  SymbolName=IN_PCAN_Rx_Ctrl_Out_Ctrl_WorkingMode_002686  DataType=boolean  Init=0  Slope=1  Bias=0  DataSize=1  fpDataType=boolean  BlockIOType=Inport  DeviceType=0
  out_OUT_DigitalOutputsSTATIC.OUT_01 : KIBES_Signal/KIBES_Signal  MBDS_LibraryBlock=on  DatabaseKey=304  SignalName=OUT_DigitalOutputsSTATIC.OUT_01  SymbolName=OUT_DigitalOutputsSTATIC_OUT_01_000304  DataType=boolean  Init=0  Slope=1  Bias=0  DataSize=1  fpDataType=boolean  BlockIOType=Outport  DeviceType=0
  out_OUT_DigitalOutputsSTATIC.OUT_01_TD_START : KIBES_Signal/KIBES_Signal  MBDS_LibraryBlock=on  DatabaseKey=315  SignalName=OUT_DigitalOutputsSTATIC.OUT_01_TD_START  SymbolName=OUT_DigitalOutputsSTATIC_OUT_01_TD_START_000315  DataType=boolean  Init=0  Slope=1  Bias=0  DataSize=1  fpDataType=boolean  BlockIOType=Outport  DeviceType=0
  out_OUT_DigitalOutputsSTATIC.OUT_02 : KIBES_Signal/KIBES_Signal  MBDS_LibraryBlock=on  DatabaseKey=249  SignalName=OUT_DigitalOutputsSTATIC.OUT_02  SymbolName=OUT_DigitalOutputsSTATIC_OUT_02_000249  DataType=boolean  Init=0  Slope=1  Bias=0  DataSize=1  fpDataType=boolean  BlockIOType=Outport  DeviceType=0
  out_OUT_DigitalOutputsSTATIC.OUT_03 : KIBES_Signal/KIBES_Signal  MBDS_LibraryBlock=on  DatabaseKey=252  SignalName=OUT_DigitalOutputsSTATIC.OUT_03  SymbolName=OUT_DigitalOutputsSTATIC_OUT_03_000252  DataType=boolean  Init=0  Slope=1  Bias=0  DataSize=1  fpDataType=boolean  BlockIOType=Outport  DeviceType=0
  out_OUT_DigitalOutputsSTATIC.OUT_04 : KIBES_Signal/KIBES_Signal  MBDS_LibraryBlock=on  DatabaseKey=255  SignalName=OUT_DigitalOutputsSTATIC.OUT_04  SymbolName=OUT_DigitalOutputsSTATIC_OUT_04_000255  DataType=boolean  Init=0  Slope=1  Bias=0  DataSize=1  fpDataType=boolean  BlockIOType=Outport  DeviceType=0
  out_OUT_DigitalOutputsSTATIC.OUT_04_TD_START : KIBES_Signal/KIBES_Signal  MBDS_LibraryBlock=on  DatabaseKey=320  SignalName=OUT_DigitalOutputsSTATIC.OUT_04_TD_START  SymbolName=OUT_DigitalOutputsSTATIC_OUT_04_TD_START_000320  DataType=boolean  Init=0  Slope=1  Bias=0  DataSize=1  fpDataType=boolean  BlockIOType=Outport  DeviceType=0
  out_OUT_DigitalOutputsSTATIC.OUT_05 : KIBES_Signal/KIBES_Signal  MBDS_LibraryBlock=on  DatabaseKey=258  SignalName=OUT_DigitalOutputsSTATIC.OUT_05  SymbolName=OUT_DigitalOutputsSTATIC_OUT_05_000258  DataType=boolean  Init=0  Slope=1  Bias=0  DataSize=1  fpDataType=boolean  BlockIOType=Outport  DeviceType=0
  out_OUT_DigitalOutputsSTATIC.OUT_06 : KIBES_Signal/KIBES_Signal  MBDS_LibraryBlock=on  DatabaseKey=261  SignalName=OUT_DigitalOutputsSTATIC.OUT_06  SymbolName=OUT_DigitalOutputsSTATIC_OUT_06_000261  DataType=boolean  Init=0  Slope=1  Bias=0  DataSize=1  fpDataType=boolean  BlockIOType=Outport  DeviceType=0
  out_OUT_DigitalOutputsSTATIC.OUT_06_TD_START : KIBES_Signal/KIBES_Signal  MBDS_LibraryBlock=on  DatabaseKey=295  SignalName=OUT_DigitalOutputsSTATIC.OUT_06_TD_START  SymbolName=OUT_DigitalOutputsSTATIC_OUT_06_TD_START_000295  DataType=boolean  Init=0  Slope=1  Bias=0  DataSize=1  fpDataType=boolean  BlockIOType=Outport  DeviceType=0
  out_OUT_DigitalOutputsSTATIC.OUT_07 : KIBES_Signal/KIBES_Signal  MBDS_LibraryBlock=on  DatabaseKey=288  SignalName=OUT_DigitalOutputsSTATIC.OUT_07  SymbolName=OUT_DigitalOutputsSTATIC_OUT_07_000288  DataType=boolean  Init=0  Slope=1  Bias=0  DataSize=1  fpDataType=boolean  BlockIOType=Outport  DeviceType=0
  out_OUT_DigitalOutputsSTATIC.OUT_07_TD_START : KIBES_Signal/KIBES_Signal  MBDS_LibraryBlock=on  DatabaseKey=296  SignalName=OUT_DigitalOutputsSTATIC.OUT_07_TD_START  SymbolName=OUT_DigitalOutputsSTATIC_OUT_07_TD_START_000296  DataType=boolean  Init=0  Slope=1  Bias=0  DataSize=1  fpDataType=boolean  BlockIOType=Outport  DeviceType=0
  out_OUT_DigitalOutputsSTATIC.OUT_08 : KIBES_Signal/KIBES_Signal  MBDS_LibraryBlock=on  DatabaseKey=297  SignalName=OUT_DigitalOutputsSTATIC.OUT_08  SymbolName=OUT_DigitalOutputsSTATIC_OUT_08_000297  DataType=boolean  Init=0  Slope=1  Bias=0  DataSize=1  fpDataType=boolean  BlockIOType=Outport  DeviceType=0
  out_OUT_DigitalOutputsSTATIC.OUT_08_TD_START : KIBES_Signal/KIBES_Signal  MBDS_LibraryBlock=on  DatabaseKey=321  SignalName=OUT_DigitalOutputsSTATIC.OUT_08_TD_START  SymbolName=OUT_DigitalOutputsSTATIC_OUT_08_TD_START_000321  DataType=boolean  Init=0  Slope=1  Bias=0  DataSize=1  fpDataType=boolean  BlockIOType=Outport  DeviceType=0
  out_OUT_DigitalOutputsSTATIC.OUT_09 : KIBES_Signal/KIBES_Signal  MBDS_LibraryBlock=on  DatabaseKey=266  SignalName=OUT_DigitalOutputsSTATIC.OUT_09  SymbolName=OUT_DigitalOutputsSTATIC_OUT_09_000266  DataType=boolean  Init=0  Slope=1  Bias=0  DataSize=1  fpDataType=boolean  BlockIOType=Outport  DeviceType=0
  out_OUT_DigitalOutputsSTATIC.OUT_10 : KIBES_Signal/KIBES_Signal  MBDS_LibraryBlock=on  DatabaseKey=268  SignalName=OUT_DigitalOutputsSTATIC.OUT_10  SymbolName=OUT_DigitalOutputsSTATIC_OUT_10_000268  DataType=boolean  Init=0  Slope=1  Bias=0  DataSize=1  fpDataType=boolean  BlockIOType=Outport  DeviceType=0
  out_OUT_DigitalOutputsSTATIC.OUT_11 : KIBES_Signal/KIBES_Signal  MBDS_LibraryBlock=on  DatabaseKey=271  SignalName=OUT_DigitalOutputsSTATIC.OUT_11  SymbolName=OUT_DigitalOutputsSTATIC_OUT_11_000271  DataType=boolean  Init=0  Slope=1  Bias=0  DataSize=1  fpDataType=boolean  BlockIOType=Outport  DeviceType=0
  out_OUT_DigitalOutputsSTATIC.OUT_12 : KIBES_Signal/KIBES_Signal  MBDS_LibraryBlock=on  DatabaseKey=283  SignalName=OUT_DigitalOutputsSTATIC.OUT_12  SymbolName=OUT_DigitalOutputsSTATIC_OUT_12_000283  DataType=boolean  Init=0  Slope=1  Bias=0  DataSize=1  fpDataType=boolean  BlockIOType=Outport  DeviceType=0
  out_OUT_DigitalOutputsSTATIC.OUT_12_TD_START : KIBES_Signal/KIBES_Signal  MBDS_LibraryBlock=on  DatabaseKey=350  SignalName=OUT_DigitalOutputsSTATIC.OUT_12_TD_START  SymbolName=OUT_DigitalOutputsSTATIC_OUT_12_TD_START_000350  DataType=boolean  Init=0  Slope=1  Bias=0  DataSize=1  fpDataType=boolean  BlockIOType=Outport  DeviceType=0
  out_OUT_DigitalOutputsSTATIC.OUT_13 : KIBES_Signal/KIBES_Signal  MBDS_LibraryBlock=on  DatabaseKey=326  SignalName=OUT_DigitalOutputsSTATIC.OUT_13  SymbolName=OUT_DigitalOutputsSTATIC_OUT_13_000326  DataType=boolean  Init=0  Slope=1  Bias=0  DataSize=1  fpDataType=boolean  BlockIOType=Outport  DeviceType=0
  out_OUT_DigitalOutputsSTATIC.OUT_13_TD_START : KIBES_Signal/KIBES_Signal  MBDS_LibraryBlock=on  DatabaseKey=351  SignalName=OUT_DigitalOutputsSTATIC.OUT_13_TD_START  SymbolName=OUT_DigitalOutputsSTATIC_OUT_13_TD_START_000351  DataType=boolean  Init=0  Slope=1  Bias=0  DataSize=1  fpDataType=boolean  BlockIOType=Outport  DeviceType=0
  out_OUT_DigitalOutputsSTATIC.OUT_14 : KIBES_Signal/KIBES_Signal  MBDS_LibraryBlock=on  DatabaseKey=333  SignalName=OUT_DigitalOutputsSTATIC.OUT_14  SymbolName=OUT_DigitalOutputsSTATIC_OUT_14_000333  DataType=boolean  Init=0  Slope=1  Bias=0  DataSize=1  fpDataType=boolean  BlockIOType=Outport  DeviceType=0
  out_OUT_DigitalOutputsSTATIC.OUT_14_TD_START : KIBES_Signal/KIBES_Signal  MBDS_LibraryBlock=on  DatabaseKey=352  SignalName=OUT_DigitalOutputsSTATIC.OUT_14_TD_START  SymbolName=OUT_DigitalOutputsSTATIC_OUT_14_TD_START_000352  DataType=boolean  Init=0  Slope=1  Bias=0  DataSize=1  fpDataType=boolean  BlockIOType=Outport  DeviceType=0
  out_OUT_DigitalOutputsSTATIC.OUT_15 : KIBES_Signal/KIBES_Signal  MBDS_LibraryBlock=on  DatabaseKey=343  SignalName=OUT_DigitalOutputsSTATIC.OUT_15  SymbolName=OUT_DigitalOutputsSTATIC_OUT_15_000343  DataType=boolean  Init=0  Slope=1  Bias=0  DataSize=1  fpDataType=boolean  BlockIOType=Outport  DeviceType=0
  out_OUT_DigitalOutputsSTATIC.OUT_15_TD_START : KIBES_Signal/KIBES_Signal  MBDS_LibraryBlock=on  DatabaseKey=353  SignalName=OUT_DigitalOutputsSTATIC.OUT_15_TD_START  SymbolName=OUT_DigitalOutputsSTATIC_OUT_15_TD_START_000353  DataType=boolean  Init=0  Slope=1  Bias=0  DataSize=1  fpDataType=boolean  BlockIOType=Outport  DeviceType=0
  out_OUT_DigitalOutputsSTATIC.OUT_16 : KIBES_Signal/KIBES_Signal  MBDS_LibraryBlock=on  DatabaseKey=274  SignalName=OUT_DigitalOutputsSTATIC.OUT_16  SymbolName=OUT_DigitalOutputsSTATIC_OUT_16_000274  DataType=boolean  Init=0  Slope=1  Bias=0  DataSize=1  fpDataType=boolean  BlockIOType=Outport  DeviceType=0
  out_OUT_DigitalOutputsSTATIC.OUT_17 : KIBES_Signal/KIBES_Signal  MBDS_LibraryBlock=on  DatabaseKey=277  SignalName=OUT_DigitalOutputsSTATIC.OUT_17  SymbolName=OUT_DigitalOutputsSTATIC_OUT_17_000277  DataType=boolean  Init=0  Slope=1  Bias=0  DataSize=1  fpDataType=boolean  BlockIOType=Outport  DeviceType=0
  out_OUT_DigitalOutputsSTATIC.OUT_19 : KIBES_Signal/KIBES_Signal  MBDS_LibraryBlock=on  DatabaseKey=309  SignalName=OUT_DigitalOutputsSTATIC.OUT_19  SymbolName=OUT_DigitalOutputsSTATIC_OUT_19_000309  DataType=boolean  Init=0  Slope=1  Bias=0  DataSize=1  fpDataType=boolean  BlockIOType=Outport  DeviceType=0
  out_OUT_PCAN.Rx_Ctrl.Out_Ctrl.MessageEnable : KIBES_Signal/KIBES_Signal  MBDS_LibraryBlock=on  DatabaseKey=1714  SignalName=OUT_PCAN.Rx_Ctrl.Out_Ctrl.MessageEnable  SymbolName=OUT_PCAN_Rx_Ctrl_Out_Ctrl_MessageEnable_001714  DataType=boolean  Init=0  Slope=1  Bias=0  DataSize=1  fpDataType=boolean  BlockIOType=Outport  DeviceType=0
  out_OUT_PCAN.Tx_Out.Out_01_Sts.MessageEnable : KIBES_Signal/KIBES_Signal  MBDS_LibraryBlock=on  DatabaseKey=1649  SignalName=OUT_PCAN.Tx_Out.Out_01_Sts.MessageEnable  SymbolName=OUT_PCAN_Tx_Out_Out_01_Sts_MessageEnable_001649  DataType=boolean  Init=0  Slope=1  Bias=0  DataSize=1  fpDataType=boolean  BlockIOType=Outport  DeviceType=0
  out_OUT_PCAN.Tx_Out.Out_01_Sts.Out_DIAG : KIBES_Signal/KIBES_Signal  MBDS_LibraryBlock=on  DatabaseKey=1543  SignalName=OUT_PCAN.Tx_Out.Out_01_Sts.Out_DIAG  SymbolName=OUT_PCAN_Tx_Out_Out_01_Sts_Out_DIAG_001543  DataType=uint16  Init=0  Slope=1  Bias=0  DataSize=1  fpDataType=uint16  BlockIOType=Outport  DeviceType=0
  out_OUT_PCAN.Tx_Out.Out_01_Sts.Out_SENSE : KIBES_Signal/KIBES_Signal  MBDS_LibraryBlock=on  DatabaseKey=1542  SignalName=OUT_PCAN.Tx_Out.Out_01_Sts.Out_SENSE  SymbolName=OUT_PCAN_Tx_Out_Out_01_Sts_Out_SENSE_001542  DataType=uint16  Init=0  Slope=1  Bias=0  DataSize=1  fpDataType=uint16  BlockIOType=Outport  DeviceType=0
  out_OUT_PCAN.Tx_Out.Out_01_Sts.Out_STATUS : KIBES_Signal/KIBES_Signal  MBDS_LibraryBlock=on  DatabaseKey=1544  SignalName=OUT_PCAN.Tx_Out.Out_01_Sts.Out_STATUS  SymbolName=OUT_PCAN_Tx_Out_Out_01_Sts_Out_STATUS_001544  DataType=uint8  Init=0  Slope=1  Bias=0  DataSize=1  fpDataType=uint8  BlockIOType=Outport  DeviceType=0
  out_OUT_PCAN.Tx_Out.Out_01_Sts.Out_TD : KIBES_Signal/KIBES_Signal  MBDS_LibraryBlock=on  DatabaseKey=1540  SignalName=OUT_PCAN.Tx_Out.Out_01_Sts.Out_TD  SymbolName=OUT_PCAN_Tx_Out_Out_01_Sts_Out_TD_001540  DataType=boolean  Init=0  Slope=1  Bias=0  DataSize=1  fpDataType=boolean  BlockIOType=Outport  DeviceType=0
  out_OUT_PCAN.Tx_Out.Out_01_Sts.Out_TD_DIAG : KIBES_Signal/KIBES_Signal  MBDS_LibraryBlock=on  DatabaseKey=1541  SignalName=OUT_PCAN.Tx_Out.Out_01_Sts.Out_TD_DIAG  SymbolName=OUT_PCAN_Tx_Out_Out_01_Sts_Out_TD_DIAG_001541  DataType=uint16  Init=0  Slope=1  Bias=0  DataSize=1  fpDataType=uint16  BlockIOType=Outport  DeviceType=0
  out_OUT_PCAN.Tx_Out.Out_01_TD_Sts.MessageEnable : KIBES_Signal/KIBES_Signal  MBDS_LibraryBlock=on  DatabaseKey=2191  SignalName=OUT_PCAN.Tx_Out.Out_01_TD_Sts.MessageEnable  SymbolName=OUT_PCAN_Tx_Out_Out_01_TD_Sts_MessageEnable_002191  DataType=boolean  Init=0  Slope=1  Bias=0  DataSize=1  fpDataType=boolean  BlockIOType=Outport  DeviceType=0
  out_OUT_PCAN.Tx_Out.Out_01_TD_Sts.Out_SENSE_PULSE : KIBES_Signal/KIBES_Signal  MBDS_LibraryBlock=on  DatabaseKey=2169  SignalName=OUT_PCAN.Tx_Out.Out_01_TD_Sts.Out_SENSE_PULSE  SymbolName=OUT_PCAN_Tx_Out_Out_01_TD_Sts_Out_SENSE_PULSE_002169  DataType=uint16  Init=0  Slope=1  Bias=0  DataSize=1  fpDataType=uint16  BlockIOType=Outport  DeviceType=0
  out_OUT_PCAN.Tx_Out.Out_01_TD_Sts.Out_SENSE_PULSE_DIAG : KIBES_Signal/KIBES_Signal  MBDS_LibraryBlock=on  DatabaseKey=2170  SignalName=OUT_PCAN.Tx_Out.Out_01_TD_Sts.Out_SENSE_PULSE_DIAG  SymbolName=OUT_PCAN_Tx_Out_Out_01_TD_Sts_Out_SENSE_PULSE_DIAG_002170  DataType=uint16  Init=0  Slope=1  Bias=0  DataSize=1  fpDataType=uint16  BlockIOType=Outport  DeviceType=0
  out_OUT_PCAN.Tx_Out.Out_02_Sts.MessageEnable : KIBES_Signal/KIBES_Signal  MBDS_LibraryBlock=on  DatabaseKey=1650  SignalName=OUT_PCAN.Tx_Out.Out_02_Sts.MessageEnable  SymbolName=OUT_PCAN_Tx_Out_Out_02_Sts_MessageEnable_001650  DataType=boolean  Init=0  Slope=1  Bias=0  DataSize=1  fpDataType=boolean  BlockIOType=Outport  DeviceType=0
  out_OUT_PCAN.Tx_Out.Out_02_Sts.Out_DIAG : KIBES_Signal/KIBES_Signal  MBDS_LibraryBlock=on  DatabaseKey=1546  SignalName=OUT_PCAN.Tx_Out.Out_02_Sts.Out_DIAG  SymbolName=OUT_PCAN_Tx_Out_Out_02_Sts_Out_DIAG_001546  DataType=uint16  Init=0  Slope=1  Bias=0  DataSize=1  fpDataType=uint16  BlockIOType=Outport  DeviceType=0
  out_OUT_PCAN.Tx_Out.Out_02_Sts.Out_SENSE : KIBES_Signal/KIBES_Signal  MBDS_LibraryBlock=on  DatabaseKey=1545  SignalName=OUT_PCAN.Tx_Out.Out_02_Sts.Out_SENSE  SymbolName=OUT_PCAN_Tx_Out_Out_02_Sts_Out_SENSE_001545  DataType=uint16  Init=0  Slope=1  Bias=0  DataSize=1  fpDataType=uint16  BlockIOType=Outport  DeviceType=0
  out_OUT_PCAN.Tx_Out.Out_02_Sts.Out_STATUS : KIBES_Signal/KIBES_Signal  MBDS_LibraryBlock=on  DatabaseKey=1547  SignalName=OUT_PCAN.Tx_Out.Out_02_Sts.Out_STATUS  SymbolName=OUT_PCAN_Tx_Out_Out_02_Sts_Out_STATUS_001547  DataType=uint8  Init=0  Slope=1  Bias=0  DataSize=1  fpDataType=uint8  BlockIOType=Outport  DeviceType=0
  out_OUT_PCAN.Tx_Out.Out_03_Sts.MessageEnable : KIBES_Signal/KIBES_Signal  MBDS_LibraryBlock=on  DatabaseKey=1651  SignalName=OUT_PCAN.Tx_Out.Out_03_Sts.MessageEnable  SymbolName=OUT_PCAN_Tx_Out_Out_03_Sts_MessageEnable_001651  DataType=boolean  Init=0  Slope=1  Bias=0  DataSize=1  fpDataType=boolean  BlockIOType=Outport  DeviceType=0
  out_OUT_PCAN.Tx_Out.Out_03_Sts.Out_DIAG : KIBES_Signal/KIBES_Signal  MBDS_LibraryBlock=on  DatabaseKey=1549  SignalName=OUT_PCAN.Tx_Out.Out_03_Sts.Out_DIAG  SymbolName=OUT_PCAN_Tx_Out_Out_03_Sts_Out_DIAG_001549  DataType=uint16  Init=0  Slope=1  Bias=0  DataSize=1  fpDataType=uint16  BlockIOType=Outport  DeviceType=0
  out_OUT_PCAN.Tx_Out.Out_03_Sts.Out_SENSE : KIBES_Signal/KIBES_Signal  MBDS_LibraryBlock=on  DatabaseKey=1548  SignalName=OUT_PCAN.Tx_Out.Out_03_Sts.Out_SENSE  SymbolName=OUT_PCAN_Tx_Out_Out_03_Sts_Out_SENSE_001548  DataType=uint16  Init=0  Slope=1  Bias=0  DataSize=1  fpDataType=uint16  BlockIOType=Outport  DeviceType=0
  out_OUT_PCAN.Tx_Out.Out_03_Sts.Out_STATUS : KIBES_Signal/KIBES_Signal  MBDS_LibraryBlock=on  DatabaseKey=1550  SignalName=OUT_PCAN.Tx_Out.Out_03_Sts.Out_STATUS  SymbolName=OUT_PCAN_Tx_Out_Out_03_Sts_Out_STATUS_001550  DataType=uint8  Init=0  Slope=1  Bias=0  DataSize=1  fpDataType=uint8  BlockIOType=Outport  DeviceType=0
  out_OUT_PCAN.Tx_Out.Out_04_Sts.MessageEnable : KIBES_Signal/KIBES_Signal  MBDS_LibraryBlock=on  DatabaseKey=1652  SignalName=OUT_PCAN.Tx_Out.Out_04_Sts.MessageEnable  SymbolName=OUT_PCAN_Tx_Out_Out_04_Sts_MessageEnable_001652  DataType=boolean  Init=0  Slope=1  Bias=0  DataSize=1  fpDataType=boolean  BlockIOType=Outport  DeviceType=0
  out_OUT_PCAN.Tx_Out.Out_04_Sts.Out_DIAG : KIBES_Signal/KIBES_Signal  MBDS_LibraryBlock=on  DatabaseKey=1554  SignalName=OUT_PCAN.Tx_Out.Out_04_Sts.Out_DIAG  SymbolName=OUT_PCAN_Tx_Out_Out_04_Sts_Out_DIAG_001554  DataType=uint16  Init=0  Slope=1  Bias=0  DataSize=1  fpDataType=uint16  BlockIOType=Outport  DeviceType=0
  out_OUT_PCAN.Tx_Out.Out_04_Sts.Out_SENSE : KIBES_Signal/KIBES_Signal  MBDS_LibraryBlock=on  DatabaseKey=1553  SignalName=OUT_PCAN.Tx_Out.Out_04_Sts.Out_SENSE  SymbolName=OUT_PCAN_Tx_Out_Out_04_Sts_Out_SENSE_001553  DataType=uint16  Init=0  Slope=1  Bias=0  DataSize=1  fpDataType=uint16  BlockIOType=Outport  DeviceType=0
  out_OUT_PCAN.Tx_Out.Out_04_Sts.Out_STATUS : KIBES_Signal/KIBES_Signal  MBDS_LibraryBlock=on  DatabaseKey=1555  SignalName=OUT_PCAN.Tx_Out.Out_04_Sts.Out_STATUS  SymbolName=OUT_PCAN_Tx_Out_Out_04_Sts_Out_STATUS_001555  DataType=uint8  Init=0  Slope=1  Bias=0  DataSize=1  fpDataType=uint8  BlockIOType=Outport  DeviceType=0
  out_OUT_PCAN.Tx_Out.Out_04_Sts.Out_TD : KIBES_Signal/KIBES_Signal  MBDS_LibraryBlock=on  DatabaseKey=1552  SignalName=OUT_PCAN.Tx_Out.Out_04_Sts.Out_TD  SymbolName=OUT_PCAN_Tx_Out_Out_04_Sts_Out_TD_001552  DataType=boolean  Init=0  Slope=1  Bias=0  DataSize=1  fpDataType=boolean  BlockIOType=Outport  DeviceType=0
  out_OUT_PCAN.Tx_Out.Out_04_Sts.Out_TD_DIAG : KIBES_Signal/KIBES_Signal  MBDS_LibraryBlock=on  DatabaseKey=1551  SignalName=OUT_PCAN.Tx_Out.Out_04_Sts.Out_TD_DIAG  SymbolName=OUT_PCAN_Tx_Out_Out_04_Sts_Out_TD_DIAG_001551  DataType=uint16  Init=0  Slope=1  Bias=0  DataSize=1  fpDataType=uint16  BlockIOType=Outport  DeviceType=0
  out_OUT_PCAN.Tx_Out.Out_04_TD_Sts.MessageEnable : KIBES_Signal/KIBES_Signal  MBDS_LibraryBlock=on  DatabaseKey=2192  SignalName=OUT_PCAN.Tx_Out.Out_04_TD_Sts.MessageEnable  SymbolName=OUT_PCAN_Tx_Out_Out_04_TD_Sts_MessageEnable_002192  DataType=boolean  Init=0  Slope=1  Bias=0  DataSize=1  fpDataType=boolean  BlockIOType=Outport  DeviceType=0
  out_OUT_PCAN.Tx_Out.Out_04_TD_Sts.Out_SENSE_PULSE : KIBES_Signal/KIBES_Signal  MBDS_LibraryBlock=on  DatabaseKey=2171  SignalName=OUT_PCAN.Tx_Out.Out_04_TD_Sts.Out_SENSE_PULSE  SymbolName=OUT_PCAN_Tx_Out_Out_04_TD_Sts_Out_SENSE_PULSE_002171  DataType=uint16  Init=0  Slope=1  Bias=0  DataSize=1  fpDataType=uint16  BlockIOType=Outport  DeviceType=0
  out_OUT_PCAN.Tx_Out.Out_04_TD_Sts.Out_SENSE_PULSE_DIAG : KIBES_Signal/KIBES_Signal  MBDS_LibraryBlock=on  DatabaseKey=2172  SignalName=OUT_PCAN.Tx_Out.Out_04_TD_Sts.Out_SENSE_PULSE_DIAG  SymbolName=OUT_PCAN_Tx_Out_Out_04_TD_Sts_Out_SENSE_PULSE_DIAG_002172  DataType=uint16  Init=0  Slope=1  Bias=0  DataSize=1  fpDataType=uint16  BlockIOType=Outport  DeviceType=0
  out_OUT_PCAN.Tx_Out.Out_05_Sts.MessageEnable : KIBES_Signal/KIBES_Signal  MBDS_LibraryBlock=on  DatabaseKey=1653  SignalName=OUT_PCAN.Tx_Out.Out_05_Sts.MessageEnable  SymbolName=OUT_PCAN_Tx_Out_Out_05_Sts_MessageEnable_001653  DataType=boolean  Init=0  Slope=1  Bias=0  DataSize=1  fpDataType=boolean  BlockIOType=Outport  DeviceType=0
  out_OUT_PCAN.Tx_Out.Out_05_Sts.Out_DIAG : KIBES_Signal/KIBES_Signal  MBDS_LibraryBlock=on  DatabaseKey=1557  SignalName=OUT_PCAN.Tx_Out.Out_05_Sts.Out_DIAG  SymbolName=OUT_PCAN_Tx_Out_Out_05_Sts_Out_DIAG_001557  DataType=uint16  Init=0  Slope=1  Bias=0  DataSize=1  fpDataType=uint16  BlockIOType=Outport  DeviceType=0
  out_OUT_PCAN.Tx_Out.Out_05_Sts.Out_SENSE : KIBES_Signal/KIBES_Signal  MBDS_LibraryBlock=on  DatabaseKey=1556  SignalName=OUT_PCAN.Tx_Out.Out_05_Sts.Out_SENSE  SymbolName=OUT_PCAN_Tx_Out_Out_05_Sts_Out_SENSE_001556  DataType=uint16  Init=0  Slope=1  Bias=0  DataSize=1  fpDataType=uint16  BlockIOType=Outport  DeviceType=0
  out_OUT_PCAN.Tx_Out.Out_05_Sts.Out_STATUS : KIBES_Signal/KIBES_Signal  MBDS_LibraryBlock=on  DatabaseKey=1558  SignalName=OUT_PCAN.Tx_Out.Out_05_Sts.Out_STATUS  SymbolName=OUT_PCAN_Tx_Out_Out_05_Sts_Out_STATUS_001558  DataType=uint8  Init=0  Slope=1  Bias=0  DataSize=1  fpDataType=uint8  BlockIOType=Outport  DeviceType=0
  out_OUT_PCAN.Tx_Out.Out_06_Sts.MessageEnable : KIBES_Signal/KIBES_Signal  MBDS_LibraryBlock=on  DatabaseKey=1654  SignalName=OUT_PCAN.Tx_Out.Out_06_Sts.MessageEnable  SymbolName=OUT_PCAN_Tx_Out_Out_06_Sts_MessageEnable_001654  DataType=boolean  Init=0  Slope=1  Bias=0  DataSize=1  fpDataType=boolean  BlockIOType=Outport  DeviceType=0
  out_OUT_PCAN.Tx_Out.Out_06_Sts.Out_DIAG : KIBES_Signal/KIBES_Signal  MBDS_LibraryBlock=on  DatabaseKey=1562  SignalName=OUT_PCAN.Tx_Out.Out_06_Sts.Out_DIAG  SymbolName=OUT_PCAN_Tx_Out_Out_06_Sts_Out_DIAG_001562  DataType=uint16  Init=0  Slope=1  Bias=0  DataSize=1  fpDataType=uint16  BlockIOType=Outport  DeviceType=0
  out_OUT_PCAN.Tx_Out.Out_06_Sts.Out_SENSE : KIBES_Signal/KIBES_Signal  MBDS_LibraryBlock=on  DatabaseKey=1561  SignalName=OUT_PCAN.Tx_Out.Out_06_Sts.Out_SENSE  SymbolName=OUT_PCAN_Tx_Out_Out_06_Sts_Out_SENSE_001561  DataType=uint16  Init=0  Slope=1  Bias=0  DataSize=1  fpDataType=uint16  BlockIOType=Outport  DeviceType=0
  out_OUT_PCAN.Tx_Out.Out_06_Sts.Out_STATUS : KIBES_Signal/KIBES_Signal  MBDS_LibraryBlock=on  DatabaseKey=1563  SignalName=OUT_PCAN.Tx_Out.Out_06_Sts.Out_STATUS  SymbolName=OUT_PCAN_Tx_Out_Out_06_Sts_Out_STATUS_001563  DataType=uint8  Init=0  Slope=1  Bias=0  DataSize=1  fpDataType=uint8  BlockIOType=Outport  DeviceType=0
  out_OUT_PCAN.Tx_Out.Out_06_Sts.Out_TD : KIBES_Signal/KIBES_Signal  MBDS_LibraryBlock=on  DatabaseKey=1560  SignalName=OUT_PCAN.Tx_Out.Out_06_Sts.Out_TD  SymbolName=OUT_PCAN_Tx_Out_Out_06_Sts_Out_TD_001560  DataType=boolean  Init=0  Slope=1  Bias=0  DataSize=1  fpDataType=boolean  BlockIOType=Outport  DeviceType=0
  out_OUT_PCAN.Tx_Out.Out_06_Sts.Out_TD_DIAG : KIBES_Signal/KIBES_Signal  MBDS_LibraryBlock=on  DatabaseKey=1559  SignalName=OUT_PCAN.Tx_Out.Out_06_Sts.Out_TD_DIAG  SymbolName=OUT_PCAN_Tx_Out_Out_06_Sts_Out_TD_DIAG_001559  DataType=uint16  Init=0  Slope=1  Bias=0  DataSize=1  fpDataType=uint16  BlockIOType=Outport  DeviceType=0
  out_OUT_PCAN.Tx_Out.Out_06_TD_Sts.MessageEnable : KIBES_Signal/KIBES_Signal  MBDS_LibraryBlock=on  DatabaseKey=2193  SignalName=OUT_PCAN.Tx_Out.Out_06_TD_Sts.MessageEnable  SymbolName=OUT_PCAN_Tx_Out_Out_06_TD_Sts_MessageEnable_002193  DataType=boolean  Init=0  Slope=1  Bias=0  DataSize=1  fpDataType=boolean  BlockIOType=Outport  DeviceType=0
  out_OUT_PCAN.Tx_Out.Out_06_TD_Sts.Out_SENSE_PULSE : KIBES_Signal/KIBES_Signal  MBDS_LibraryBlock=on  DatabaseKey=2173  SignalName=OUT_PCAN.Tx_Out.Out_06_TD_Sts.Out_SENSE_PULSE  SymbolName=OUT_PCAN_Tx_Out_Out_06_TD_Sts_Out_SENSE_PULSE_002173  DataType=uint16  Init=0  Slope=1  Bias=0  DataSize=1  fpDataType=uint16  BlockIOType=Outport  DeviceType=0
  out_OUT_PCAN.Tx_Out.Out_06_TD_Sts.Out_SENSE_PULSE_DIAG : KIBES_Signal/KIBES_Signal  MBDS_LibraryBlock=on  DatabaseKey=2174  SignalName=OUT_PCAN.Tx_Out.Out_06_TD_Sts.Out_SENSE_PULSE_DIAG  SymbolName=OUT_PCAN_Tx_Out_Out_06_TD_Sts_Out_SENSE_PULSE_DIAG_002174  DataType=uint16  Init=0  Slope=1  Bias=0  DataSize=1  fpDataType=uint16  BlockIOType=Outport  DeviceType=0
  out_OUT_PCAN.Tx_Out.Out_07_Sts.MessageEnable : KIBES_Signal/KIBES_Signal  MBDS_LibraryBlock=on  DatabaseKey=1655  SignalName=OUT_PCAN.Tx_Out.Out_07_Sts.MessageEnable  SymbolName=OUT_PCAN_Tx_Out_Out_07_Sts_MessageEnable_001655  DataType=boolean  Init=0  Slope=1  Bias=0  DataSize=1  fpDataType=boolean  BlockIOType=Outport  DeviceType=0
  out_OUT_PCAN.Tx_Out.Out_07_Sts.Out_DIAG : KIBES_Signal/KIBES_Signal  MBDS_LibraryBlock=on  DatabaseKey=1567  SignalName=OUT_PCAN.Tx_Out.Out_07_Sts.Out_DIAG  SymbolName=OUT_PCAN_Tx_Out_Out_07_Sts_Out_DIAG_001567  DataType=uint16  Init=0  Slope=1  Bias=0  DataSize=1  fpDataType=uint16  BlockIOType=Outport  DeviceType=0
  out_OUT_PCAN.Tx_Out.Out_07_Sts.Out_SENSE : KIBES_Signal/KIBES_Signal  MBDS_LibraryBlock=on  DatabaseKey=1566  SignalName=OUT_PCAN.Tx_Out.Out_07_Sts.Out_SENSE  SymbolName=OUT_PCAN_Tx_Out_Out_07_Sts_Out_SENSE_001566  DataType=uint16  Init=0  Slope=1  Bias=0  DataSize=1  fpDataType=uint16  BlockIOType=Outport  DeviceType=0
  out_OUT_PCAN.Tx_Out.Out_07_Sts.Out_STATUS : KIBES_Signal/KIBES_Signal  MBDS_LibraryBlock=on  DatabaseKey=1568  SignalName=OUT_PCAN.Tx_Out.Out_07_Sts.Out_STATUS  SymbolName=OUT_PCAN_Tx_Out_Out_07_Sts_Out_STATUS_001568  DataType=uint8  Init=0  Slope=1  Bias=0  DataSize=1  fpDataType=uint8  BlockIOType=Outport  DeviceType=0
  out_OUT_PCAN.Tx_Out.Out_07_Sts.Out_TD : KIBES_Signal/KIBES_Signal  MBDS_LibraryBlock=on  DatabaseKey=1565  SignalName=OUT_PCAN.Tx_Out.Out_07_Sts.Out_TD  SymbolName=OUT_PCAN_Tx_Out_Out_07_Sts_Out_TD_001565  DataType=boolean  Init=0  Slope=1  Bias=0  DataSize=1  fpDataType=boolean  BlockIOType=Outport  DeviceType=0
  out_OUT_PCAN.Tx_Out.Out_07_Sts.Out_TD_DIAG : KIBES_Signal/KIBES_Signal  MBDS_LibraryBlock=on  DatabaseKey=1564  SignalName=OUT_PCAN.Tx_Out.Out_07_Sts.Out_TD_DIAG  SymbolName=OUT_PCAN_Tx_Out_Out_07_Sts_Out_TD_DIAG_001564  DataType=uint16  Init=0  Slope=1  Bias=0  DataSize=1  fpDataType=uint16  BlockIOType=Outport  DeviceType=0
  out_OUT_PCAN.Tx_Out.Out_07_TD_Sts.MessageEnable : KIBES_Signal/KIBES_Signal  MBDS_LibraryBlock=on  DatabaseKey=2194  SignalName=OUT_PCAN.Tx_Out.Out_07_TD_Sts.MessageEnable  SymbolName=OUT_PCAN_Tx_Out_Out_07_TD_Sts_MessageEnable_002194  DataType=boolean  Init=0  Slope=1  Bias=0  DataSize=1  fpDataType=boolean  BlockIOType=Outport  DeviceType=0
  out_OUT_PCAN.Tx_Out.Out_07_TD_Sts.Out_SENSE_PULSE : KIBES_Signal/KIBES_Signal  MBDS_LibraryBlock=on  DatabaseKey=2175  SignalName=OUT_PCAN.Tx_Out.Out_07_TD_Sts.Out_SENSE_PULSE  SymbolName=OUT_PCAN_Tx_Out_Out_07_TD_Sts_Out_SENSE_PULSE_002175  DataType=uint16  Init=0  Slope=1  Bias=0  DataSize=1  fpDataType=uint16  BlockIOType=Outport  DeviceType=0
  out_OUT_PCAN.Tx_Out.Out_07_TD_Sts.Out_SENSE_PULSE_DIAG : KIBES_Signal/KIBES_Signal  MBDS_LibraryBlock=on  DatabaseKey=2176  SignalName=OUT_PCAN.Tx_Out.Out_07_TD_Sts.Out_SENSE_PULSE_DIAG  SymbolName=OUT_PCAN_Tx_Out_Out_07_TD_Sts_Out_SENSE_PULSE_DIAG_002176  DataType=uint16  Init=0  Slope=1  Bias=0  DataSize=1  fpDataType=uint16  BlockIOType=Outport  DeviceType=0
  out_OUT_PCAN.Tx_Out.Out_08_Sts.MessageEnable : KIBES_Signal/KIBES_Signal  MBDS_LibraryBlock=on  DatabaseKey=1656  SignalName=OUT_PCAN.Tx_Out.Out_08_Sts.MessageEnable  SymbolName=OUT_PCAN_Tx_Out_Out_08_Sts_MessageEnable_001656  DataType=boolean  Init=0  Slope=1  Bias=0  DataSize=1  fpDataType=boolean  BlockIOType=Outport  DeviceType=0
  out_OUT_PCAN.Tx_Out.Out_08_Sts.Out_DIAG : KIBES_Signal/KIBES_Signal  MBDS_LibraryBlock=on  DatabaseKey=1572  SignalName=OUT_PCAN.Tx_Out.Out_08_Sts.Out_DIAG  SymbolName=OUT_PCAN_Tx_Out_Out_08_Sts_Out_DIAG_001572  DataType=uint16  Init=0  Slope=1  Bias=0  DataSize=1  fpDataType=uint16  BlockIOType=Outport  DeviceType=0
  out_OUT_PCAN.Tx_Out.Out_08_Sts.Out_SENSE : KIBES_Signal/KIBES_Signal  MBDS_LibraryBlock=on  DatabaseKey=1571  SignalName=OUT_PCAN.Tx_Out.Out_08_Sts.Out_SENSE  SymbolName=OUT_PCAN_Tx_Out_Out_08_Sts_Out_SENSE_001571  DataType=uint16  Init=0  Slope=1  Bias=0  DataSize=1  fpDataType=uint16  BlockIOType=Outport  DeviceType=0
  out_OUT_PCAN.Tx_Out.Out_08_Sts.Out_STATUS : KIBES_Signal/KIBES_Signal  MBDS_LibraryBlock=on  DatabaseKey=1573  SignalName=OUT_PCAN.Tx_Out.Out_08_Sts.Out_STATUS  SymbolName=OUT_PCAN_Tx_Out_Out_08_Sts_Out_STATUS_001573  DataType=uint8  Init=0  Slope=1  Bias=0  DataSize=1  fpDataType=uint8  BlockIOType=Outport  DeviceType=0
  out_OUT_PCAN.Tx_Out.Out_08_Sts.Out_TD : KIBES_Signal/KIBES_Signal  MBDS_LibraryBlock=on  DatabaseKey=1570  SignalName=OUT_PCAN.Tx_Out.Out_08_Sts.Out_TD  SymbolName=OUT_PCAN_Tx_Out_Out_08_Sts_Out_TD_001570  DataType=boolean  Init=0  Slope=1  Bias=0  DataSize=1  fpDataType=boolean  BlockIOType=Outport  DeviceType=0
  out_OUT_PCAN.Tx_Out.Out_08_Sts.Out_TD_DIAG : KIBES_Signal/KIBES_Signal  MBDS_LibraryBlock=on  DatabaseKey=1569  SignalName=OUT_PCAN.Tx_Out.Out_08_Sts.Out_TD_DIAG  SymbolName=OUT_PCAN_Tx_Out_Out_08_Sts_Out_TD_DIAG_001569  DataType=uint16  Init=0  Slope=1  Bias=0  DataSize=1  fpDataType=uint16  BlockIOType=Outport  DeviceType=0
  out_OUT_PCAN.Tx_Out.Out_08_TD_Sts.MessageEnable : KIBES_Signal/KIBES_Signal  MBDS_LibraryBlock=on  DatabaseKey=2195  SignalName=OUT_PCAN.Tx_Out.Out_08_TD_Sts.MessageEnable  SymbolName=OUT_PCAN_Tx_Out_Out_08_TD_Sts_MessageEnable_002195  DataType=boolean  Init=0  Slope=1  Bias=0  DataSize=1  fpDataType=boolean  BlockIOType=Outport  DeviceType=0
  out_OUT_PCAN.Tx_Out.Out_08_TD_Sts.Out_SENSE_PULSE : KIBES_Signal/KIBES_Signal  MBDS_LibraryBlock=on  DatabaseKey=2177  SignalName=OUT_PCAN.Tx_Out.Out_08_TD_Sts.Out_SENSE_PULSE  SymbolName=OUT_PCAN_Tx_Out_Out_08_TD_Sts_Out_SENSE_PULSE_002177  DataType=uint16  Init=0  Slope=1  Bias=0  DataSize=1  fpDataType=uint16  BlockIOType=Outport  DeviceType=0
  out_OUT_PCAN.Tx_Out.Out_08_TD_Sts.Out_SENSE_PULSE_DIAG : KIBES_Signal/KIBES_Signal  MBDS_LibraryBlock=on  DatabaseKey=2178  SignalName=OUT_PCAN.Tx_Out.Out_08_TD_Sts.Out_SENSE_PULSE_DIAG  SymbolName=OUT_PCAN_Tx_Out_Out_08_TD_Sts_Out_SENSE_PULSE_DIAG_002178  DataType=uint16  Init=0  Slope=1  Bias=0  DataSize=1  fpDataType=uint16  BlockIOType=Outport  DeviceType=0
  out_OUT_PCAN.Tx_Out.Out_09_Sts.MessageEnable : KIBES_Signal/KIBES_Signal  MBDS_LibraryBlock=on  DatabaseKey=1657  SignalName=OUT_PCAN.Tx_Out.Out_09_Sts.MessageEnable  SymbolName=OUT_PCAN_Tx_Out_Out_09_Sts_MessageEnable_001657  DataType=boolean  Init=0  Slope=1  Bias=0  DataSize=1  fpDataType=boolean  BlockIOType=Outport  DeviceType=0
  out_OUT_PCAN.Tx_Out.Out_09_Sts.Out_DIAG : KIBES_Signal/KIBES_Signal  MBDS_LibraryBlock=on  DatabaseKey=1575  SignalName=OUT_PCAN.Tx_Out.Out_09_Sts.Out_DIAG  SymbolName=OUT_PCAN_Tx_Out_Out_09_Sts_Out_DIAG_001575  DataType=uint16  Init=0  Slope=1  Bias=0  DataSize=1  fpDataType=uint16  BlockIOType=Outport  DeviceType=0
  out_OUT_PCAN.Tx_Out.Out_09_Sts.Out_SENSE : KIBES_Signal/KIBES_Signal  MBDS_LibraryBlock=on  DatabaseKey=1574  SignalName=OUT_PCAN.Tx_Out.Out_09_Sts.Out_SENSE  SymbolName=OUT_PCAN_Tx_Out_Out_09_Sts_Out_SENSE_001574  DataType=uint16  Init=0  Slope=1  Bias=0  DataSize=1  fpDataType=uint16  BlockIOType=Outport  DeviceType=0
  out_OUT_PCAN.Tx_Out.Out_09_Sts.Out_STATUS : KIBES_Signal/KIBES_Signal  MBDS_LibraryBlock=on  DatabaseKey=1576  SignalName=OUT_PCAN.Tx_Out.Out_09_Sts.Out_STATUS  SymbolName=OUT_PCAN_Tx_Out_Out_09_Sts_Out_STATUS_001576  DataType=uint8  Init=0  Slope=1  Bias=0  DataSize=1  fpDataType=uint8  BlockIOType=Outport  DeviceType=0
  out_OUT_PCAN.Tx_Out.Out_10_Sts.MessageEnable : KIBES_Signal/KIBES_Signal  MBDS_LibraryBlock=on  DatabaseKey=1658  SignalName=OUT_PCAN.Tx_Out.Out_10_Sts.MessageEnable  SymbolName=OUT_PCAN_Tx_Out_Out_10_Sts_MessageEnable_001658  DataType=boolean  Init=0  Slope=1  Bias=0  DataSize=1  fpDataType=boolean  BlockIOType=Outport  DeviceType=0
  out_OUT_PCAN.Tx_Out.Out_10_Sts.Out_DIAG : KIBES_Signal/KIBES_Signal  MBDS_LibraryBlock=on  DatabaseKey=1578  SignalName=OUT_PCAN.Tx_Out.Out_10_Sts.Out_DIAG  SymbolName=OUT_PCAN_Tx_Out_Out_10_Sts_Out_DIAG_001578  DataType=uint16  Init=0  Slope=1  Bias=0  DataSize=1  fpDataType=uint16  BlockIOType=Outport  DeviceType=0
  out_OUT_PCAN.Tx_Out.Out_10_Sts.Out_SENSE : KIBES_Signal/KIBES_Signal  MBDS_LibraryBlock=on  DatabaseKey=1577  SignalName=OUT_PCAN.Tx_Out.Out_10_Sts.Out_SENSE  SymbolName=OUT_PCAN_Tx_Out_Out_10_Sts_Out_SENSE_001577  DataType=uint16  Init=0  Slope=1  Bias=0  DataSize=1  fpDataType=uint16  BlockIOType=Outport  DeviceType=0
  out_OUT_PCAN.Tx_Out.Out_10_Sts.Out_STATUS : KIBES_Signal/KIBES_Signal  MBDS_LibraryBlock=on  DatabaseKey=1579  SignalName=OUT_PCAN.Tx_Out.Out_10_Sts.Out_STATUS  SymbolName=OUT_PCAN_Tx_Out_Out_10_Sts_Out_STATUS_001579  DataType=uint8  Init=0  Slope=1  Bias=0  DataSize=1  fpDataType=uint8  BlockIOType=Outport  DeviceType=0
  out_OUT_PCAN.Tx_Out.Out_11_Sts.MessageEnable : KIBES_Signal/KIBES_Signal  MBDS_LibraryBlock=on  DatabaseKey=1659  SignalName=OUT_PCAN.Tx_Out.Out_11_Sts.MessageEnable  SymbolName=OUT_PCAN_Tx_Out_Out_11_Sts_MessageEnable_001659  DataType=boolean  Init=0  Slope=1  Bias=0  DataSize=1  fpDataType=boolean  BlockIOType=Outport  DeviceType=0
  out_OUT_PCAN.Tx_Out.Out_11_Sts.Out_DIAG : KIBES_Signal/KIBES_Signal  MBDS_LibraryBlock=on  DatabaseKey=1581  SignalName=OUT_PCAN.Tx_Out.Out_11_Sts.Out_DIAG  SymbolName=OUT_PCAN_Tx_Out_Out_11_Sts_Out_DIAG_001581  DataType=uint16  Init=0  Slope=1  Bias=0  DataSize=1  fpDataType=uint16  BlockIOType=Outport  DeviceType=0
  out_OUT_PCAN.Tx_Out.Out_11_Sts.Out_SENSE : KIBES_Signal/KIBES_Signal  MBDS_LibraryBlock=on  DatabaseKey=1580  SignalName=OUT_PCAN.Tx_Out.Out_11_Sts.Out_SENSE  SymbolName=OUT_PCAN_Tx_Out_Out_11_Sts_Out_SENSE_001580  DataType=uint16  Init=0  Slope=1  Bias=0  DataSize=1  fpDataType=uint16  BlockIOType=Outport  DeviceType=0
  out_OUT_PCAN.Tx_Out.Out_11_Sts.Out_STATUS : KIBES_Signal/KIBES_Signal  MBDS_LibraryBlock=on  DatabaseKey=1582  SignalName=OUT_PCAN.Tx_Out.Out_11_Sts.Out_STATUS  SymbolName=OUT_PCAN_Tx_Out_Out_11_Sts_Out_STATUS_001582  DataType=uint8  Init=0  Slope=1  Bias=0  DataSize=1  fpDataType=uint8  BlockIOType=Outport  DeviceType=0
  out_OUT_PCAN.Tx_Out.Out_12_Sts.MessageEnable : KIBES_Signal/KIBES_Signal  MBDS_LibraryBlock=on  DatabaseKey=1660  SignalName=OUT_PCAN.Tx_Out.Out_12_Sts.MessageEnable  SymbolName=OUT_PCAN_Tx_Out_Out_12_Sts_MessageEnable_001660  DataType=boolean  Init=0  Slope=1  Bias=0  DataSize=1  fpDataType=boolean  BlockIOType=Outport  DeviceType=0
  out_OUT_PCAN.Tx_Out.Out_12_Sts.Out_DIAG : KIBES_Signal/KIBES_Signal  MBDS_LibraryBlock=on  DatabaseKey=1586  SignalName=OUT_PCAN.Tx_Out.Out_12_Sts.Out_DIAG  SymbolName=OUT_PCAN_Tx_Out_Out_12_Sts_Out_DIAG_001586  DataType=uint16  Init=0  Slope=1  Bias=0  DataSize=1  fpDataType=uint16  BlockIOType=Outport  DeviceType=0
  out_OUT_PCAN.Tx_Out.Out_12_Sts.Out_SENSE : KIBES_Signal/KIBES_Signal  MBDS_LibraryBlock=on  DatabaseKey=1585  SignalName=OUT_PCAN.Tx_Out.Out_12_Sts.Out_SENSE  SymbolName=OUT_PCAN_Tx_Out_Out_12_Sts_Out_SENSE_001585  DataType=uint16  Init=0  Slope=1  Bias=0  DataSize=1  fpDataType=uint16  BlockIOType=Outport  DeviceType=0
  out_OUT_PCAN.Tx_Out.Out_12_Sts.Out_STATUS : KIBES_Signal/KIBES_Signal  MBDS_LibraryBlock=on  DatabaseKey=1587  SignalName=OUT_PCAN.Tx_Out.Out_12_Sts.Out_STATUS  SymbolName=OUT_PCAN_Tx_Out_Out_12_Sts_Out_STATUS_001587  DataType=uint8  Init=0  Slope=1  Bias=0  DataSize=1  fpDataType=uint8  BlockIOType=Outport  DeviceType=0
  out_OUT_PCAN.Tx_Out.Out_12_Sts.Out_TD : KIBES_Signal/KIBES_Signal  MBDS_LibraryBlock=on  DatabaseKey=1584  SignalName=OUT_PCAN.Tx_Out.Out_12_Sts.Out_TD  SymbolName=OUT_PCAN_Tx_Out_Out_12_Sts_Out_TD_001584  DataType=boolean  Init=0  Slope=1  Bias=0  DataSize=1  fpDataType=boolean  BlockIOType=Outport  DeviceType=0
  out_OUT_PCAN.Tx_Out.Out_12_Sts.Out_TD_DIAG : KIBES_Signal/KIBES_Signal  MBDS_LibraryBlock=on  DatabaseKey=1583  SignalName=OUT_PCAN.Tx_Out.Out_12_Sts.Out_TD_DIAG  SymbolName=OUT_PCAN_Tx_Out_Out_12_Sts_Out_TD_DIAG_001583  DataType=uint16  Init=0  Slope=1  Bias=0  DataSize=1  fpDataType=uint16  BlockIOType=Outport  DeviceType=0
  out_OUT_PCAN.Tx_Out.Out_12_TD_Sts.MessageEnable : KIBES_Signal/KIBES_Signal  MBDS_LibraryBlock=on  DatabaseKey=2196  SignalName=OUT_PCAN.Tx_Out.Out_12_TD_Sts.MessageEnable  SymbolName=OUT_PCAN_Tx_Out_Out_12_TD_Sts_MessageEnable_002196  DataType=boolean  Init=0  Slope=1  Bias=0  DataSize=1  fpDataType=boolean  BlockIOType=Outport  DeviceType=0
  out_OUT_PCAN.Tx_Out.Out_12_TD_Sts.Out_SENSE_PULSE : KIBES_Signal/KIBES_Signal  MBDS_LibraryBlock=on  DatabaseKey=2179  SignalName=OUT_PCAN.Tx_Out.Out_12_TD_Sts.Out_SENSE_PULSE  SymbolName=OUT_PCAN_Tx_Out_Out_12_TD_Sts_Out_SENSE_PULSE_002179  DataType=uint16  Init=0  Slope=1  Bias=0  DataSize=1  fpDataType=uint16  BlockIOType=Outport  DeviceType=0
  out_OUT_PCAN.Tx_Out.Out_12_TD_Sts.Out_SENSE_PULSE_DIAG : KIBES_Signal/KIBES_Signal  MBDS_LibraryBlock=on  DatabaseKey=2180  SignalName=OUT_PCAN.Tx_Out.Out_12_TD_Sts.Out_SENSE_PULSE_DIAG  SymbolName=OUT_PCAN_Tx_Out_Out_12_TD_Sts_Out_SENSE_PULSE_DIAG_002180  DataType=uint16  Init=0  Slope=1  Bias=0  DataSize=1  fpDataType=uint16  BlockIOType=Outport  DeviceType=0
  out_OUT_PCAN.Tx_Out.Out_13_Sts.MessageEnable : KIBES_Signal/KIBES_Signal  MBDS_LibraryBlock=on  DatabaseKey=1661  SignalName=OUT_PCAN.Tx_Out.Out_13_Sts.MessageEnable  SymbolName=OUT_PCAN_Tx_Out_Out_13_Sts_MessageEnable_001661  DataType=boolean  Init=0  Slope=1  Bias=0  DataSize=1  fpDataType=boolean  BlockIOType=Outport  DeviceType=0
  out_OUT_PCAN.Tx_Out.Out_13_Sts.Out_DIAG : KIBES_Signal/KIBES_Signal  MBDS_LibraryBlock=on  DatabaseKey=1591  SignalName=OUT_PCAN.Tx_Out.Out_13_Sts.Out_DIAG  SymbolName=OUT_PCAN_Tx_Out_Out_13_Sts_Out_DIAG_001591  DataType=uint16  Init=0  Slope=1  Bias=0  DataSize=1  fpDataType=uint16  BlockIOType=Outport  DeviceType=0
  out_OUT_PCAN.Tx_Out.Out_13_Sts.Out_SENSE : KIBES_Signal/KIBES_Signal  MBDS_LibraryBlock=on  DatabaseKey=1590  SignalName=OUT_PCAN.Tx_Out.Out_13_Sts.Out_SENSE  SymbolName=OUT_PCAN_Tx_Out_Out_13_Sts_Out_SENSE_001590  DataType=uint16  Init=0  Slope=1  Bias=0  DataSize=1  fpDataType=uint16  BlockIOType=Outport  DeviceType=0
  out_OUT_PCAN.Tx_Out.Out_13_Sts.Out_STATUS : KIBES_Signal/KIBES_Signal  MBDS_LibraryBlock=on  DatabaseKey=1592  SignalName=OUT_PCAN.Tx_Out.Out_13_Sts.Out_STATUS  SymbolName=OUT_PCAN_Tx_Out_Out_13_Sts_Out_STATUS_001592  DataType=uint8  Init=0  Slope=1  Bias=0  DataSize=1  fpDataType=uint8  BlockIOType=Outport  DeviceType=0
  out_OUT_PCAN.Tx_Out.Out_13_Sts.Out_TD : KIBES_Signal/KIBES_Signal  MBDS_LibraryBlock=on  DatabaseKey=1589  SignalName=OUT_PCAN.Tx_Out.Out_13_Sts.Out_TD  SymbolName=OUT_PCAN_Tx_Out_Out_13_Sts_Out_TD_001589  DataType=boolean  Init=0  Slope=1  Bias=0  DataSize=1  fpDataType=boolean  BlockIOType=Outport  DeviceType=0
  out_OUT_PCAN.Tx_Out.Out_13_Sts.Out_TD_DIAG : KIBES_Signal/KIBES_Signal  MBDS_LibraryBlock=on  DatabaseKey=1588  SignalName=OUT_PCAN.Tx_Out.Out_13_Sts.Out_TD_DIAG  SymbolName=OUT_PCAN_Tx_Out_Out_13_Sts_Out_TD_DIAG_001588  DataType=uint16  Init=0  Slope=1  Bias=0  DataSize=1  fpDataType=uint16  BlockIOType=Outport  DeviceType=0
  out_OUT_PCAN.Tx_Out.Out_13_TD_Sts.MessageEnable : KIBES_Signal/KIBES_Signal  MBDS_LibraryBlock=on  DatabaseKey=2197  SignalName=OUT_PCAN.Tx_Out.Out_13_TD_Sts.MessageEnable  SymbolName=OUT_PCAN_Tx_Out_Out_13_TD_Sts_MessageEnable_002197  DataType=boolean  Init=0  Slope=1  Bias=0  DataSize=1  fpDataType=boolean  BlockIOType=Outport  DeviceType=0
  out_OUT_PCAN.Tx_Out.Out_13_TD_Sts.Out_SENSE_PULSE : KIBES_Signal/KIBES_Signal  MBDS_LibraryBlock=on  DatabaseKey=2181  SignalName=OUT_PCAN.Tx_Out.Out_13_TD_Sts.Out_SENSE_PULSE  SymbolName=OUT_PCAN_Tx_Out_Out_13_TD_Sts_Out_SENSE_PULSE_002181  DataType=uint16  Init=0  Slope=1  Bias=0  DataSize=1  fpDataType=uint16  BlockIOType=Outport  DeviceType=0
  out_OUT_PCAN.Tx_Out.Out_13_TD_Sts.Out_SENSE_PULSE_DIAG : KIBES_Signal/KIBES_Signal  MBDS_LibraryBlock=on  DatabaseKey=2182  SignalName=OUT_PCAN.Tx_Out.Out_13_TD_Sts.Out_SENSE_PULSE_DIAG  SymbolName=OUT_PCAN_Tx_Out_Out_13_TD_Sts_Out_SENSE_PULSE_DIAG_002182  DataType=uint16  Init=0  Slope=1  Bias=0  DataSize=1  fpDataType=uint16  BlockIOType=Outport  DeviceType=0
  out_OUT_PCAN.Tx_Out.Out_14_Sts.MessageEnable : KIBES_Signal/KIBES_Signal  MBDS_LibraryBlock=on  DatabaseKey=1662  SignalName=OUT_PCAN.Tx_Out.Out_14_Sts.MessageEnable  SymbolName=OUT_PCAN_Tx_Out_Out_14_Sts_MessageEnable_001662  DataType=boolean  Init=0  Slope=1  Bias=0  DataSize=1  fpDataType=boolean  BlockIOType=Outport  DeviceType=0
  out_OUT_PCAN.Tx_Out.Out_14_Sts.Out_DIAG : KIBES_Signal/KIBES_Signal  MBDS_LibraryBlock=on  DatabaseKey=1596  SignalName=OUT_PCAN.Tx_Out.Out_14_Sts.Out_DIAG  SymbolName=OUT_PCAN_Tx_Out_Out_14_Sts_Out_DIAG_001596  DataType=uint16  Init=0  Slope=1  Bias=0  DataSize=1  fpDataType=uint16  BlockIOType=Outport  DeviceType=0
  out_OUT_PCAN.Tx_Out.Out_14_Sts.Out_SENSE : KIBES_Signal/KIBES_Signal  MBDS_LibraryBlock=on  DatabaseKey=1595  SignalName=OUT_PCAN.Tx_Out.Out_14_Sts.Out_SENSE  SymbolName=OUT_PCAN_Tx_Out_Out_14_Sts_Out_SENSE_001595  DataType=uint16  Init=0  Slope=1  Bias=0  DataSize=1  fpDataType=uint16  BlockIOType=Outport  DeviceType=0
  out_OUT_PCAN.Tx_Out.Out_14_Sts.Out_STATUS : KIBES_Signal/KIBES_Signal  MBDS_LibraryBlock=on  DatabaseKey=1597  SignalName=OUT_PCAN.Tx_Out.Out_14_Sts.Out_STATUS  SymbolName=OUT_PCAN_Tx_Out_Out_14_Sts_Out_STATUS_001597  DataType=uint8  Init=0  Slope=1  Bias=0  DataSize=1  fpDataType=uint8  BlockIOType=Outport  DeviceType=0
  out_OUT_PCAN.Tx_Out.Out_14_Sts.Out_TD : KIBES_Signal/KIBES_Signal  MBDS_LibraryBlock=on  DatabaseKey=1594  SignalName=OUT_PCAN.Tx_Out.Out_14_Sts.Out_TD  SymbolName=OUT_PCAN_Tx_Out_Out_14_Sts_Out_TD_001594  DataType=boolean  Init=0  Slope=1  Bias=0  DataSize=1  fpDataType=boolean  BlockIOType=Outport  DeviceType=0
  out_OUT_PCAN.Tx_Out.Out_14_Sts.Out_TD_DIAG : KIBES_Signal/KIBES_Signal  MBDS_LibraryBlock=on  DatabaseKey=1593  SignalName=OUT_PCAN.Tx_Out.Out_14_Sts.Out_TD_DIAG  SymbolName=OUT_PCAN_Tx_Out_Out_14_Sts_Out_TD_DIAG_001593  DataType=uint16  Init=0  Slope=1  Bias=0  DataSize=1  fpDataType=uint16  BlockIOType=Outport  DeviceType=0
  out_OUT_PCAN.Tx_Out.Out_14_TD_Sts.MessageEnable : KIBES_Signal/KIBES_Signal  MBDS_LibraryBlock=on  DatabaseKey=2198  SignalName=OUT_PCAN.Tx_Out.Out_14_TD_Sts.MessageEnable  SymbolName=OUT_PCAN_Tx_Out_Out_14_TD_Sts_MessageEnable_002198  DataType=boolean  Init=0  Slope=1  Bias=0  DataSize=1  fpDataType=boolean  BlockIOType=Outport  DeviceType=0
  out_OUT_PCAN.Tx_Out.Out_14_TD_Sts.Out_SENSE_PULSE : KIBES_Signal/KIBES_Signal  MBDS_LibraryBlock=on  DatabaseKey=2183  SignalName=OUT_PCAN.Tx_Out.Out_14_TD_Sts.Out_SENSE_PULSE  SymbolName=OUT_PCAN_Tx_Out_Out_14_TD_Sts_Out_SENSE_PULSE_002183  DataType=uint16  Init=0  Slope=1  Bias=0  DataSize=1  fpDataType=uint16  BlockIOType=Outport  DeviceType=0
  out_OUT_PCAN.Tx_Out.Out_14_TD_Sts.Out_SENSE_PULSE_DIAG : KIBES_Signal/KIBES_Signal  MBDS_LibraryBlock=on  DatabaseKey=2184  SignalName=OUT_PCAN.Tx_Out.Out_14_TD_Sts.Out_SENSE_PULSE_DIAG  SymbolName=OUT_PCAN_Tx_Out_Out_14_TD_Sts_Out_SENSE_PULSE_DIAG_002184  DataType=uint16  Init=0  Slope=1  Bias=0  DataSize=1  fpDataType=uint16  BlockIOType=Outport  DeviceType=0
  out_OUT_PCAN.Tx_Out.Out_15_Sts.MessageEnable : KIBES_Signal/KIBES_Signal  MBDS_LibraryBlock=on  DatabaseKey=1663  SignalName=OUT_PCAN.Tx_Out.Out_15_Sts.MessageEnable  SymbolName=OUT_PCAN_Tx_Out_Out_15_Sts_MessageEnable_001663  DataType=boolean  Init=0  Slope=1  Bias=0  DataSize=1  fpDataType=boolean  BlockIOType=Outport  DeviceType=0
  out_OUT_PCAN.Tx_Out.Out_15_Sts.Out_DIAG : KIBES_Signal/KIBES_Signal  MBDS_LibraryBlock=on  DatabaseKey=1601  SignalName=OUT_PCAN.Tx_Out.Out_15_Sts.Out_DIAG  SymbolName=OUT_PCAN_Tx_Out_Out_15_Sts_Out_DIAG_001601  DataType=uint16  Init=0  Slope=1  Bias=0  DataSize=1  fpDataType=uint16  BlockIOType=Outport  DeviceType=0
  out_OUT_PCAN.Tx_Out.Out_15_Sts.Out_SENSE : KIBES_Signal/KIBES_Signal  MBDS_LibraryBlock=on  DatabaseKey=1600  SignalName=OUT_PCAN.Tx_Out.Out_15_Sts.Out_SENSE  SymbolName=OUT_PCAN_Tx_Out_Out_15_Sts_Out_SENSE_001600  DataType=uint16  Init=0  Slope=1  Bias=0  DataSize=1  fpDataType=uint16  BlockIOType=Outport  DeviceType=0
  out_OUT_PCAN.Tx_Out.Out_15_Sts.Out_STATUS : KIBES_Signal/KIBES_Signal  MBDS_LibraryBlock=on  DatabaseKey=1602  SignalName=OUT_PCAN.Tx_Out.Out_15_Sts.Out_STATUS  SymbolName=OUT_PCAN_Tx_Out_Out_15_Sts_Out_STATUS_001602  DataType=uint8  Init=0  Slope=1  Bias=0  DataSize=1  fpDataType=uint8  BlockIOType=Outport  DeviceType=0
  out_OUT_PCAN.Tx_Out.Out_15_Sts.Out_TD : KIBES_Signal/KIBES_Signal  MBDS_LibraryBlock=on  DatabaseKey=1599  SignalName=OUT_PCAN.Tx_Out.Out_15_Sts.Out_TD  SymbolName=OUT_PCAN_Tx_Out_Out_15_Sts_Out_TD_001599  DataType=boolean  Init=0  Slope=1  Bias=0  DataSize=1  fpDataType=boolean  BlockIOType=Outport  DeviceType=0
  out_OUT_PCAN.Tx_Out.Out_15_Sts.Out_TD_DIAG : KIBES_Signal/KIBES_Signal  MBDS_LibraryBlock=on  DatabaseKey=1598  SignalName=OUT_PCAN.Tx_Out.Out_15_Sts.Out_TD_DIAG  SymbolName=OUT_PCAN_Tx_Out_Out_15_Sts_Out_TD_DIAG_001598  DataType=uint16  Init=0  Slope=1  Bias=0  DataSize=1  fpDataType=uint16  BlockIOType=Outport  DeviceType=0
  out_OUT_PCAN.Tx_Out.Out_15_TD_Sts.MessageEnable : KIBES_Signal/KIBES_Signal  MBDS_LibraryBlock=on  DatabaseKey=2199  SignalName=OUT_PCAN.Tx_Out.Out_15_TD_Sts.MessageEnable  SymbolName=OUT_PCAN_Tx_Out_Out_15_TD_Sts_MessageEnable_002199  DataType=boolean  Init=0  Slope=1  Bias=0  DataSize=1  fpDataType=boolean  BlockIOType=Outport  DeviceType=0
  out_OUT_PCAN.Tx_Out.Out_15_TD_Sts.Out_SENSE_PULSE : KIBES_Signal/KIBES_Signal  MBDS_LibraryBlock=on  DatabaseKey=2185  SignalName=OUT_PCAN.Tx_Out.Out_15_TD_Sts.Out_SENSE_PULSE  SymbolName=OUT_PCAN_Tx_Out_Out_15_TD_Sts_Out_SENSE_PULSE_002185  DataType=uint16  Init=0  Slope=1  Bias=0  DataSize=1  fpDataType=uint16  BlockIOType=Outport  DeviceType=0
  out_OUT_PCAN.Tx_Out.Out_15_TD_Sts.Out_SENSE_PULSE_DIAG : KIBES_Signal/KIBES_Signal  MBDS_LibraryBlock=on  DatabaseKey=2186  SignalName=OUT_PCAN.Tx_Out.Out_15_TD_Sts.Out_SENSE_PULSE_DIAG  SymbolName=OUT_PCAN_Tx_Out_Out_15_TD_Sts_Out_SENSE_PULSE_DIAG_002186  DataType=uint16  Init=0  Slope=1  Bias=0  DataSize=1  fpDataType=uint16  BlockIOType=Outport  DeviceType=0
  out_OUT_PCAN.Tx_Out.Out_16_Sts.MessageEnable : KIBES_Signal/KIBES_Signal  MBDS_LibraryBlock=on  DatabaseKey=1664  SignalName=OUT_PCAN.Tx_Out.Out_16_Sts.MessageEnable  SymbolName=OUT_PCAN_Tx_Out_Out_16_Sts_MessageEnable_001664  DataType=boolean  Init=0  Slope=1  Bias=0  DataSize=1  fpDataType=boolean  BlockIOType=Outport  DeviceType=0
  out_OUT_PCAN.Tx_Out.Out_16_Sts.Out_DIAG : KIBES_Signal/KIBES_Signal  MBDS_LibraryBlock=on  DatabaseKey=1604  SignalName=OUT_PCAN.Tx_Out.Out_16_Sts.Out_DIAG  SymbolName=OUT_PCAN_Tx_Out_Out_16_Sts_Out_DIAG_001604  DataType=uint16  Init=0  Slope=1  Bias=0  DataSize=1  fpDataType=uint16  BlockIOType=Outport  DeviceType=0
  out_OUT_PCAN.Tx_Out.Out_16_Sts.Out_SENSE : KIBES_Signal/KIBES_Signal  MBDS_LibraryBlock=on  DatabaseKey=1603  SignalName=OUT_PCAN.Tx_Out.Out_16_Sts.Out_SENSE  SymbolName=OUT_PCAN_Tx_Out_Out_16_Sts_Out_SENSE_001603  DataType=uint16  Init=0  Slope=1  Bias=0  DataSize=1  fpDataType=uint16  BlockIOType=Outport  DeviceType=0
  out_OUT_PCAN.Tx_Out.Out_16_Sts.Out_STATUS : KIBES_Signal/KIBES_Signal  MBDS_LibraryBlock=on  DatabaseKey=1605  SignalName=OUT_PCAN.Tx_Out.Out_16_Sts.Out_STATUS  SymbolName=OUT_PCAN_Tx_Out_Out_16_Sts_Out_STATUS_001605  DataType=uint8  Init=0  Slope=1  Bias=0  DataSize=1  fpDataType=uint8  BlockIOType=Outport  DeviceType=0
  out_OUT_PCAN.Tx_Out.Out_17_Sts.MessageEnable : KIBES_Signal/KIBES_Signal  MBDS_LibraryBlock=on  DatabaseKey=1665  SignalName=OUT_PCAN.Tx_Out.Out_17_Sts.MessageEnable  SymbolName=OUT_PCAN_Tx_Out_Out_17_Sts_MessageEnable_001665  DataType=boolean  Init=0  Slope=1  Bias=0  DataSize=1  fpDataType=boolean  BlockIOType=Outport  DeviceType=0
  out_OUT_PCAN.Tx_Out.Out_17_Sts.Out_DIAG : KIBES_Signal/KIBES_Signal  MBDS_LibraryBlock=on  DatabaseKey=1607  SignalName=OUT_PCAN.Tx_Out.Out_17_Sts.Out_DIAG  SymbolName=OUT_PCAN_Tx_Out_Out_17_Sts_Out_DIAG_001607  DataType=uint16  Init=0  Slope=1  Bias=0  DataSize=1  fpDataType=uint16  BlockIOType=Outport  DeviceType=0
  out_OUT_PCAN.Tx_Out.Out_17_Sts.Out_SENSE : KIBES_Signal/KIBES_Signal  MBDS_LibraryBlock=on  DatabaseKey=1606  SignalName=OUT_PCAN.Tx_Out.Out_17_Sts.Out_SENSE  SymbolName=OUT_PCAN_Tx_Out_Out_17_Sts_Out_SENSE_001606  DataType=uint16  Init=0  Slope=1  Bias=0  DataSize=1  fpDataType=uint16  BlockIOType=Outport  DeviceType=0
  out_OUT_PCAN.Tx_Out.Out_17_Sts.Out_STATUS : KIBES_Signal/KIBES_Signal  MBDS_LibraryBlock=on  DatabaseKey=1608  SignalName=OUT_PCAN.Tx_Out.Out_17_Sts.Out_STATUS  SymbolName=OUT_PCAN_Tx_Out_Out_17_Sts_Out_STATUS_001608  DataType=uint8  Init=0  Slope=1  Bias=0  DataSize=1  fpDataType=uint8  BlockIOType=Outport  DeviceType=0
  out_OUT_PCAN.Tx_Out.Out_19_Sts.MessageEnable : KIBES_Signal/KIBES_Signal  MBDS_LibraryBlock=on  DatabaseKey=1667  SignalName=OUT_PCAN.Tx_Out.Out_19_Sts.MessageEnable  SymbolName=OUT_PCAN_Tx_Out_Out_19_Sts_MessageEnable_001667  DataType=boolean  Init=0  Slope=1  Bias=0  DataSize=1  fpDataType=boolean  BlockIOType=Outport  DeviceType=0
  out_OUT_PCAN.Tx_Out.Out_19_Sts.Out_DIAG : KIBES_Signal/KIBES_Signal  MBDS_LibraryBlock=on  DatabaseKey=1613  SignalName=OUT_PCAN.Tx_Out.Out_19_Sts.Out_DIAG  SymbolName=OUT_PCAN_Tx_Out_Out_19_Sts_Out_DIAG_001613  DataType=uint16  Init=0  Slope=1  Bias=0  DataSize=1  fpDataType=uint16  BlockIOType=Outport  DeviceType=0
  out_OUT_PCAN.Tx_Out.Out_19_Sts.Out_SENSE : KIBES_Signal/KIBES_Signal  MBDS_LibraryBlock=on  DatabaseKey=1612  SignalName=OUT_PCAN.Tx_Out.Out_19_Sts.Out_SENSE  SymbolName=OUT_PCAN_Tx_Out_Out_19_Sts_Out_SENSE_001612  DataType=uint16  Init=0  Slope=1  Bias=0  DataSize=1  fpDataType=uint16  BlockIOType=Outport  DeviceType=0
  out_OUT_PCAN.Tx_Out.Out_19_Sts.Out_STATUS : KIBES_Signal/KIBES_Signal  MBDS_LibraryBlock=on  DatabaseKey=1614  SignalName=OUT_PCAN.Tx_Out.Out_19_Sts.Out_STATUS  SymbolName=OUT_PCAN_Tx_Out_Out_19_Sts_Out_STATUS_001614  DataType=uint8  Init=0  Slope=1  Bias=0  DataSize=1  fpDataType=uint8  BlockIOType=Outport  DeviceType=0
  wires:
  in_IN_NVM.Parameter.BlinkSourcePeriod/1 -> BlinkSource/1(u16_PeriodTime)
  BlinkSource/1(bo_Blink) -> [BlinkSource]
  in_IN_PCAN.Rx_Ctrl.Out_Ctrl.Out_15_Ctrl/1 -> Switch8/3
  [WorkingMode] -> Switch8/2
  [BlinkSource] -> Switch8/1
  in_IN_PCAN.Rx_Ctrl.Out_Ctrl.Out_14_Ctrl/1 -> Switch7/3
  [BlinkSource] -> Switch7/1
  [WorkingMode] -> Switch7/2
  in_IN_PCAN.Rx_Ctrl.Out_Ctrl.Out_13_Ctrl/1 -> Switch6/3
  [WorkingMode] -> Switch6/2
  [BlinkSource] -> Switch6/1
  in_IN_PCAN.Rx_Ctrl.Out_Ctrl.Out_12_Ctrl/1 -> Switch5/3
  [BlinkSource] -> Switch5/1
  [WorkingMode] -> Switch5/2
  in_IN_PCAN.Rx_Ctrl.Out_Ctrl.Out_08_Ctrl/1 -> Switch4/3
  [WorkingMode] -> Switch4/2
  [BlinkSource] -> Switch4/1
  in_IN_PCAN.Rx_Ctrl.Out_Ctrl.Out_07_Ctrl/1 -> Switch3/3
  [BlinkSource] -> Switch3/1
  [WorkingMode] -> Switch3/2
  in_IN_PCAN.Rx_Ctrl.Out_Ctrl.Out_06_Ctrl/1 -> Switch2/3
  [WorkingMode] -> Switch2/2
  [BlinkSource] -> Switch2/1
  [BlinkSource] -> Switch1/1
  in_IN_PCAN.Rx_Ctrl.Out_Ctrl.Out_04_Ctrl/1 -> Switch1/3
  [WorkingMode] -> Switch1/2
  Switch/1 -> AND10/2(u2)
  [BlinkSource] -> Switch/1
  [WorkingMode] -> Switch/2
  AND1/1(y) -> [WorkingMode]
  in_IN_PCAN.Rx_Ctrl.Out_Ctrl.WorkingMode/1 -> AND1/2(u2)
  [boCtrlValid] -> AND1/1(u1)
  [boOut_15_DIAG] -> MOD_OutputDiag_Ctrl_15/2
  [boOut_14_DIAG] -> MOD_OutputDiag_Ctrl_14/2
  [boOut_13_DIAG] -> MOD_OutputDiag_Ctrl_13/2
  [boOut_12_DIAG] -> MOD_OutputDiag_Ctrl_12/2
  [boOut_08_DIAG] -> MOD_OutputDiag_Ctrl_08/2
  [boOut_07_DIAG] -> MOD_OutputDiag_Ctrl_07/2
  [boOut_06_DIAG] -> MOD_OutputDiag_Ctrl_06/2
  [boOut_04_DIAG] -> MOD_OutputDiag_Ctrl_04/2
  [boOut_01_DIAG] -> MOD_OutputDiag_Ctrl_01/2
  [boOut_19_DIAG] -> MOD_OutputDiag_Ctrl_19/2
  [boOut_17_DIAG] -> MOD_OutputDiag_Ctrl_17/2
  [boOut_16_DIAG] -> MOD_OutputDiag_Ctrl_16/2
  [boOut_11_DIAG] -> MOD_OutputDiag_Ctrl_11/2
  [boOut_10_DIAG] -> MOD_OutputDiag_Ctrl_10/2
  [boOut_09_DIAG] -> MOD_OutputDiag_Ctrl_09/2
  [boOut_05_DIAG] -> MOD_OutputDiag_Ctrl_05/2
  [boOut_03_DIAG] -> MOD_OutputDiag_Ctrl_03/2
  [boOut_02_DIAG] -> MOD_OutputDiag_Ctrl_02/2
  MOD_TrailerDetection_Ctrl_15/1 -> MOD_OutputDiag_Ctrl_15/1
  MOD_TrailerDetection_Ctrl_14/1 -> MOD_OutputDiag_Ctrl_14/1
  MOD_TrailerDetection_Ctrl_13/1 -> MOD_OutputDiag_Ctrl_13/1
  MOD_TrailerDetection_Ctrl_12/1 -> MOD_OutputDiag_Ctrl_12/1
  MOD_TrailerDetection_Ctrl_08/1 -> MOD_OutputDiag_Ctrl_08/1
  MOD_TrailerDetection_Ctrl_07/1 -> MOD_OutputDiag_Ctrl_07/1
  MOD_TrailerDetection_Ctrl_06/1 -> MOD_OutputDiag_Ctrl_06/1
  MOD_TrailerDetection_Ctrl_04/1 -> MOD_OutputDiag_Ctrl_04/1
  [boCtrlValid] -> MOD_OutputDiag_Ctrl_01/3, MOD_OutputDiag_Ctrl_04/3, MOD_OutputDiag_Ctrl_06/3, MOD_OutputDiag_Ctrl_07/3, MOD_OutputDiag_Ctrl_08/3, MOD_OutputDiag_Ctrl_12/3, MOD_OutputDiag_Ctrl_13/3, MOD_OutputDiag_Ctrl_14/3, MOD_OutputDiag_Ctrl_15/3
  MOD_TrailerDetection_Ctrl_01/1 -> MOD_OutputDiag_Ctrl_01/1
  in_IN_PCAN.Rx_Ctrl.Out_Ctrl.Out_19_Ctrl/1 -> MOD_OutputDiag_Ctrl_19/1
  in_IN_PCAN.Rx_Ctrl.Out_Ctrl.Out_17_Ctrl/1 -> MOD_OutputDiag_Ctrl_17/1
  in_IN_PCAN.Rx_Ctrl.Out_Ctrl.Out_16_Ctrl/1 -> MOD_OutputDiag_Ctrl_16/1
  in_IN_PCAN.Rx_Ctrl.Out_Ctrl.Out_11_Ctrl/1 -> MOD_OutputDiag_Ctrl_11/1
  in_IN_PCAN.Rx_Ctrl.Out_Ctrl.Out_10_Ctrl/1 -> MOD_OutputDiag_Ctrl_10/1
  in_IN_PCAN.Rx_Ctrl.Out_Ctrl.Out_09_Ctrl/1 -> MOD_OutputDiag_Ctrl_09/1
  in_IN_PCAN.Rx_Ctrl.Out_Ctrl.Out_05_Ctrl/1 -> MOD_OutputDiag_Ctrl_05/1
  in_IN_PCAN.Rx_Ctrl.Out_Ctrl.Out_03_Ctrl/1 -> MOD_OutputDiag_Ctrl_03/1
  in_DIAG_DigitalOutputsSTATIC.OUT_15_SENSE_PULSE_DIAG/1 -> out_OUT_PCAN.Tx_Out.Out_15_TD_Sts.Out_SENSE_PULSE_DIAG/1
  in_IN_DigitalOutputsSTATIC.OUT_15_SENSE_PULSE/1 -> out_OUT_PCAN.Tx_Out.Out_15_TD_Sts.Out_SENSE_PULSE/1
  in_DIAG_DigitalOutputsSTATIC.OUT_14_SENSE_PULSE_DIAG/1 -> out_OUT_PCAN.Tx_Out.Out_14_TD_Sts.Out_SENSE_PULSE_DIAG/1
  in_IN_DigitalOutputsSTATIC.OUT_14_SENSE_PULSE/1 -> out_OUT_PCAN.Tx_Out.Out_14_TD_Sts.Out_SENSE_PULSE/1
  in_DIAG_DigitalOutputsSTATIC.OUT_13_SENSE_PULSE_DIAG/1 -> out_OUT_PCAN.Tx_Out.Out_13_TD_Sts.Out_SENSE_PULSE_DIAG/1
  in_IN_DigitalOutputsSTATIC.OUT_13_SENSE_PULSE/1 -> out_OUT_PCAN.Tx_Out.Out_13_TD_Sts.Out_SENSE_PULSE/1
  in_DIAG_DigitalOutputsSTATIC.OUT_12_SENSE_PULSE_DIAG/1 -> out_OUT_PCAN.Tx_Out.Out_12_TD_Sts.Out_SENSE_PULSE_DIAG/1
  in_IN_DigitalOutputsSTATIC.OUT_12_SENSE_PULSE/1 -> out_OUT_PCAN.Tx_Out.Out_12_TD_Sts.Out_SENSE_PULSE/1
  in_DIAG_DigitalOutputsSTATIC.OUT_08_SENSE_PULSE_DIAG/1 -> out_OUT_PCAN.Tx_Out.Out_08_TD_Sts.Out_SENSE_PULSE_DIAG/1
  in_IN_DigitalOutputsSTATIC.OUT_08_SENSE_PULSE/1 -> out_OUT_PCAN.Tx_Out.Out_08_TD_Sts.Out_SENSE_PULSE/1
  in_DIAG_DigitalOutputsSTATIC.OUT_06_SENSE_PULSE_DIAG/1 -> out_OUT_PCAN.Tx_Out.Out_06_TD_Sts.Out_SENSE_PULSE_DIAG/1
  in_IN_DigitalOutputsSTATIC.OUT_06_SENSE_PULSE/1 -> out_OUT_PCAN.Tx_Out.Out_06_TD_Sts.Out_SENSE_PULSE/1
  in_DIAG_DigitalOutputsSTATIC.OUT_07_SENSE_PULSE_DIAG/1 -> out_OUT_PCAN.Tx_Out.Out_07_TD_Sts.Out_SENSE_PULSE_DIAG/1
  in_IN_DigitalOutputsSTATIC.OUT_07_SENSE_PULSE/1 -> out_OUT_PCAN.Tx_Out.Out_07_TD_Sts.Out_SENSE_PULSE/1
  in_DIAG_DigitalOutputsSTATIC.OUT_04_SENSE_PULSE_DIAG/1 -> out_OUT_PCAN.Tx_Out.Out_04_TD_Sts.Out_SENSE_PULSE_DIAG/1
  in_IN_DigitalOutputsSTATIC.OUT_04_SENSE_PULSE/1 -> out_OUT_PCAN.Tx_Out.Out_04_TD_Sts.Out_SENSE_PULSE/1
  in_DIAG_DigitalOutputsSTATIC.OUT_01_SENSE_PULSE_DIAG/1 -> out_OUT_PCAN.Tx_Out.Out_01_TD_Sts.Out_SENSE_PULSE_DIAG/1
  in_IN_DigitalOutputsSTATIC.OUT_01_SENSE_PULSE/1 -> out_OUT_PCAN.Tx_Out.Out_01_TD_Sts.Out_SENSE_PULSE/1
  Data Type Conversion18/1 -> out_OUT_PCAN.Tx_Out.Out_19_Sts.Out_STATUS/1
  Data Type Conversion16/1 -> out_OUT_PCAN.Tx_Out.Out_17_Sts.Out_STATUS/1
  Data Type Conversion15/1 -> out_OUT_PCAN.Tx_Out.Out_16_Sts.Out_STATUS/1
  Data Type Conversion14/1 -> out_OUT_PCAN.Tx_Out.Out_11_Sts.Out_STATUS/1
  Data Type Conversion13/1 -> out_OUT_PCAN.Tx_Out.Out_10_Sts.Out_STATUS/1
  Data Type Conversion12/1 -> out_OUT_PCAN.Tx_Out.Out_09_Sts.Out_STATUS/1
  Data Type Conversion11/1 -> out_OUT_PCAN.Tx_Out.Out_05_Sts.Out_STATUS/1
  Data Type Conversion10/1 -> out_OUT_PCAN.Tx_Out.Out_03_Sts.Out_STATUS/1
  Data Type Conversion9/1 -> out_OUT_PCAN.Tx_Out.Out_02_Sts.Out_STATUS/1
  [boOut_15_TD] -> MOD_TrailerDetection_Ctrl_15/2
  Switch8/1 -> AND18/2(u2)
  MOD_TrailerDetection_Ctrl_15/2 -> out_OUT_DigitalOutputsSTATIC.OUT_15_TD_START/1
  Data Type Conversion8/1 -> out_OUT_PCAN.Tx_Out.Out_15_Sts.Out_STATUS/1
  [u8TdTimeout] -> MOD_TrailerDetection_Ctrl_15/4
  [u16Out_15_TD_DIAG] -> MOD_TrailerDetection_Ctrl_15/3
  MOD_OutputDiag_Ctrl_15/1 -> Data Type Conversion8/1, out_OUT_DigitalOutputsSTATIC.OUT_15/1
  AND18/1(y) -> MOD_TrailerDetection_Ctrl_15/1
  [boCtrlValid] -> AND18/1(u1)
  [u8TdTimeout] -> MOD_TrailerDetection_Ctrl_14/4
  [u16Out_14_TD_DIAG] -> MOD_TrailerDetection_Ctrl_14/3
  MOD_OutputDiag_Ctrl_14/1 -> Data Type Conversion7/1, out_OUT_DigitalOutputsSTATIC.OUT_14/1
  MOD_TrailerDetection_Ctrl_14/2 -> out_OUT_DigitalOutputsSTATIC.OUT_14_TD_START/1
  Switch7/1 -> AND17/2(u2)
  [boCtrlValid] -> AND17/1(u1)
  AND17/1(y) -> MOD_TrailerDetection_Ctrl_14/1
  Data Type Conversion7/1 -> out_OUT_PCAN.Tx_Out.Out_14_Sts.Out_STATUS/1
  [boOut_14_TD] -> MOD_TrailerDetection_Ctrl_14/2
  [boOut_13_TD] -> MOD_TrailerDetection_Ctrl_13/2
  Data Type Conversion6/1 -> out_OUT_PCAN.Tx_Out.Out_13_Sts.Out_STATUS/1
  [u16Out_13_TD_DIAG] -> MOD_TrailerDetection_Ctrl_13/3
  MOD_OutputDiag_Ctrl_13/1 -> Data Type Conversion6/1, out_OUT_DigitalOutputsSTATIC.OUT_13/1
  AND16/1(y) -> MOD_TrailerDetection_Ctrl_13/1
  Switch6/1 -> AND16/2(u2)
  [boCtrlValid] -> AND16/1(u1)
  [u8TdTimeout] -> MOD_TrailerDetection_Ctrl_13/4
  MOD_TrailerDetection_Ctrl_13/2 -> out_OUT_DigitalOutputsSTATIC.OUT_13_TD_START/1
  MOD_TrailerDetection_Ctrl_12/2 -> out_OUT_DigitalOutputsSTATIC.OUT_12_TD_START/1
  AND15/1(y) -> MOD_TrailerDetection_Ctrl_12/1
  MOD_OutputDiag_Ctrl_12/1 -> Data Type Conversion5/1, out_OUT_DigitalOutputsSTATIC.OUT_12/1
  [u8TdTimeout] -> MOD_TrailerDetection_Ctrl_12/4
  [boCtrlValid] -> AND15/1(u1)
  Data Type Conversion5/1 -> out_OUT_PCAN.Tx_Out.Out_12_Sts.Out_STATUS/1
  [u16Out_12_TD_DIAG] -> MOD_TrailerDetection_Ctrl_12/3
  [boOut_12_TD] -> MOD_TrailerDetection_Ctrl_12/2
  Switch5/1 -> AND15/2(u2)
  Data Type Conversion4/1 -> out_OUT_PCAN.Tx_Out.Out_08_Sts.Out_STATUS/1
  AND14/1(y) -> MOD_TrailerDetection_Ctrl_08/1
  [u16Out_08_TD_DIAG] -> MOD_TrailerDetection_Ctrl_08/3
  [boOut_08_TD] -> MOD_TrailerDetection_Ctrl_08/2
  [boCtrlValid] -> AND14/1(u1)
  [u8TdTimeout] -> MOD_TrailerDetection_Ctrl_08/4
  Switch4/1 -> AND14/2(u2)
  MOD_TrailerDetection_Ctrl_08/2 -> out_OUT_DigitalOutputsSTATIC.OUT_08_TD_START/1
  MOD_OutputDiag_Ctrl_08/1 -> Data Type Conversion4/1, out_OUT_DigitalOutputsSTATIC.OUT_08/1
  MOD_TrailerDetection_Ctrl_07/2 -> out_OUT_DigitalOutputsSTATIC.OUT_07_TD_START/1
  MOD_OutputDiag_Ctrl_07/1 -> out_OUT_DigitalOutputsSTATIC.OUT_07/1, Data Type Conversion3/1
  Switch3/1 -> AND13/2(u2)
  [boCtrlValid] -> AND13/1(u1)
  [u8TdTimeout] -> MOD_TrailerDetection_Ctrl_07/4
  AND13/1(y) -> MOD_TrailerDetection_Ctrl_07/1
  [boOut_07_TD] -> MOD_TrailerDetection_Ctrl_07/2
  [u16Out_07_TD_DIAG] -> MOD_TrailerDetection_Ctrl_07/3
  Data Type Conversion3/1 -> out_OUT_PCAN.Tx_Out.Out_07_Sts.Out_STATUS/1
  [u8TdTimeout] -> MOD_TrailerDetection_Ctrl_06/4
  [u16Out_06_TD_DIAG] -> MOD_TrailerDetection_Ctrl_06/3
  [boOut_06_TD] -> MOD_TrailerDetection_Ctrl_06/2
  Data Type Conversion2/1 -> out_OUT_PCAN.Tx_Out.Out_06_Sts.Out_STATUS/1
  MOD_OutputDiag_Ctrl_06/1 -> Data Type Conversion2/1, out_OUT_DigitalOutputsSTATIC.OUT_06/1
  MOD_TrailerDetection_Ctrl_06/2 -> out_OUT_DigitalOutputsSTATIC.OUT_06_TD_START/1
  AND12/1(y) -> MOD_TrailerDetection_Ctrl_06/1
  [boCtrlValid] -> AND12/1(u1)
  Switch2/1 -> AND12/2(u2)
  Switch1/1 -> AND11/2(u2)
  Data Type Conversion1/1 -> out_OUT_PCAN.Tx_Out.Out_04_Sts.Out_STATUS/1
  MOD_TrailerDetection_Ctrl_04/2 -> out_OUT_DigitalOutputsSTATIC.OUT_04_TD_START/1
  MOD_OutputDiag_Ctrl_04/1 -> out_OUT_DigitalOutputsSTATIC.OUT_04/1, Data Type Conversion1/1
  [u16Out_04_TD_DIAG] -> MOD_TrailerDetection_Ctrl_04/3
  [boOut_04_TD] -> MOD_TrailerDetection_Ctrl_04/2
  [u8TdTimeout] -> MOD_TrailerDetection_Ctrl_04/4
  [boCtrlValid] -> AND11/1(u1)
  AND11/1(y) -> MOD_TrailerDetection_Ctrl_04/1
  [u16Out_01_TD_DIAG] -> MOD_TrailerDetection_Ctrl_01/3
  [boOut_01_TD] -> MOD_TrailerDetection_Ctrl_01/2
  [u8TdTimeout] -> MOD_TrailerDetection_Ctrl_01/4
  in_IN_NVM.Parameter.TrailerDetectionTime/1 -> [u8TdTimeout]
  AND10/1(y) -> MOD_TrailerDetection_Ctrl_01/1
  in_IN_PCAN.Rx_Ctrl.Out_Ctrl.Out_01_Ctrl/1 -> Switch/3
  Data Type Conversion/1 -> out_OUT_PCAN.Tx_Out.Out_01_Sts.Out_STATUS/1
  MOD_TrailerDetection_Ctrl_01/2 -> out_OUT_DigitalOutputsSTATIC.OUT_01_TD_START/1
  MOD_OutputDiag_Ctrl_01/1 -> out_OUT_DigitalOutputsSTATIC.OUT_01/1, Data Type Conversion/1
  [boCtrlValid] -> AND10/1(u1)
  MOD_OutputDiag_Ctrl_19/1 -> out_OUT_DigitalOutputsSTATIC.OUT_19/1, Data Type Conversion18/1
  MOD_OutputDiag_Ctrl_17/1 -> out_OUT_DigitalOutputsSTATIC.OUT_17/1, Data Type Conversion16/1
  MOD_OutputDiag_Ctrl_16/1 -> out_OUT_DigitalOutputsSTATIC.OUT_16/1, Data Type Conversion15/1
  MOD_OutputDiag_Ctrl_11/1 -> out_OUT_DigitalOutputsSTATIC.OUT_11/1, Data Type Conversion14/1
  MOD_OutputDiag_Ctrl_10/1 -> out_OUT_DigitalOutputsSTATIC.OUT_10/1, Data Type Conversion13/1
  MOD_OutputDiag_Ctrl_09/1 -> out_OUT_DigitalOutputsSTATIC.OUT_09/1, Data Type Conversion12/1
  MOD_OutputDiag_Ctrl_05/1 -> out_OUT_DigitalOutputsSTATIC.OUT_05/1, Data Type Conversion11/1
  MOD_OutputDiag_Ctrl_03/1 -> out_OUT_DigitalOutputsSTATIC.OUT_03/1, Data Type Conversion10/1
  MOD_OutputDiag_Ctrl_02/1 -> out_OUT_DigitalOutputsSTATIC.OUT_02/1, Data Type Conversion9/1
  in_IN_PCAN.Rx_Ctrl.Out_Ctrl.Out_02_Ctrl/1 -> MOD_OutputDiag_Ctrl_02/1
  [boCtrlValid] -> MOD_OutputDiag_Ctrl_03/3, MOD_OutputDiag_Ctrl_05/3, MOD_OutputDiag_Ctrl_09/3, MOD_OutputDiag_Ctrl_10/3, MOD_OutputDiag_Ctrl_11/3, MOD_OutputDiag_Ctrl_16/3, MOD_OutputDiag_Ctrl_17/3, MOD_OutputDiag_Ctrl_19/3, MOD_OutputDiag_Ctrl_02/3
  EQ/1(y) -> [boCtrlValid]
  Constant1/1 -> EQ/2(u2)
  in_IN_PCAN.Rx_Ctrl.Out_Ctrl.MessageState/1 -> EQ/1(u1)
  Constant/1 -> out_OUT_PCAN.Rx_Ctrl.Out_Ctrl.MessageEnable/1
  in_IN_DigitalOutputsSTATIC.OUT_19_SENSE/1 -> out_OUT_PCAN.Tx_Out.Out_19_Sts.Out_SENSE/1
  in_DIAG_DigitalOutputsSTATIC.OUT_19_DIAG/1 -> out_OUT_PCAN.Tx_Out.Out_19_Sts.Out_DIAG/1, [boOut_18_DIAG]
  in_IN_DigitalOutputsSTATIC.OUT_17_SENSE/1 -> out_OUT_PCAN.Tx_Out.Out_17_Sts.Out_SENSE/1
  in_DIAG_DigitalOutputsSTATIC.OUT_17_DIAG/1 -> out_OUT_PCAN.Tx_Out.Out_17_Sts.Out_DIAG/1, [boOut_17_DIAG]
  in_IN_DigitalOutputsSTATIC.OUT_16_SENSE/1 -> out_OUT_PCAN.Tx_Out.Out_16_Sts.Out_SENSE/1
  in_DIAG_DigitalOutputsSTATIC.OUT_16_DIAG/1 -> out_OUT_PCAN.Tx_Out.Out_16_Sts.Out_DIAG/1, [boOut_16_DIAG]
  in_DIAG_DigitalOutputsSTATIC.OUT_15_TD_DIAG/1 -> [u16Out_15_TD_DIAG], out_OUT_PCAN.Tx_Out.Out_15_Sts.Out_TD_DIAG/1
  in_IN_DigitalOutputsSTATIC.OUT_15_TD/1 -> [boOut_15_TD], out_OUT_PCAN.Tx_Out.Out_15_Sts.Out_TD/1
  in_IN_DigitalOutputsSTATIC.OUT_15_SENSE/1 -> out_OUT_PCAN.Tx_Out.Out_15_Sts.Out_SENSE/1
  in_DIAG_DigitalOutputsSTATIC.OUT_15_DIAG/1 -> out_OUT_PCAN.Tx_Out.Out_15_Sts.Out_DIAG/1, [boOut_15_DIAG]
  in_DIAG_DigitalOutputsSTATIC.OUT_14_TD_DIAG/1 -> [u16Out_14_TD_DIAG], out_OUT_PCAN.Tx_Out.Out_14_Sts.Out_TD_DIAG/1
  in_IN_DigitalOutputsSTATIC.OUT_14_TD/1 -> [boOut_14_TD], out_OUT_PCAN.Tx_Out.Out_14_Sts.Out_TD/1
  in_IN_DigitalOutputsSTATIC.OUT_14_SENSE/1 -> out_OUT_PCAN.Tx_Out.Out_14_Sts.Out_SENSE/1
  in_DIAG_DigitalOutputsSTATIC.OUT_14_DIAG/1 -> out_OUT_PCAN.Tx_Out.Out_14_Sts.Out_DIAG/1, [boOut_14_DIAG]
  in_IN_DigitalOutputsSTATIC.OUT_13_TD/1 -> [boOut_13_TD], out_OUT_PCAN.Tx_Out.Out_13_Sts.Out_TD/1
  in_DIAG_DigitalOutputsSTATIC.OUT_13_TD_DIAG/1 -> [u16Out_13_TD_DIAG], out_OUT_PCAN.Tx_Out.Out_13_Sts.Out_TD_DIAG/1
  in_IN_DigitalOutputsSTATIC.OUT_13_SENSE/1 -> out_OUT_PCAN.Tx_Out.Out_13_Sts.Out_SENSE/1
  in_DIAG_DigitalOutputsSTATIC.OUT_13_DIAG/1 -> out_OUT_PCAN.Tx_Out.Out_13_Sts.Out_DIAG/1, [boOut_13_DIAG]
